simulink model "ImpedanceControl"  (R2017a)
(part 12 of 14)

-((imag(sin(q6).*(cos(q2-q3).*4.698463103929542e-1+sin(q2-q3).*sin(q4).*6.710100716628342e-1+cos(q5).*(cos(q2-q3).*8.191520442889917e-1-sin(q2-q3).*sin(q4).*5.735764363510462e-1).*5.735764363510462e-1-sin(q2-q3).*cos(q4).*sin(q5).*5.735764363510462e-1))+real(sqrt((cos(q2-q3).*3.289899283371657e-1+sin(q2-q3).*sin(q4).*4.698463103929542e-1-cos(q5).*(cos(q2-q3).*8.191520442889917e-1-sin(q2-q3).*sin(q4).*5.735764363510462e-1).*8.191520442889917e-1+sin(q2-q3).*cos(q4).*sin(q5).*8.191520442889917e-1).^2+(sin(q6).*(cos(q2-q3).*sin(q5).*8.191520442889917e-1+sin(q2-q3).*cos(q4).*cos(q5)-sin(q2-q3).*sin(q4).*sin(q5).*5.735764363510462e-1)-cos(q6).*(cos(q2-q3).*4.698463103929542e-1+sin(q2-q3).*sin(q4).*6.710100716628342e-1+cos(q5).*(cos(q2-q3).*8.191520442889917e-1-sin(q2-q3).*sin(q4).*5.735764363510462e-1).*5.735764363510462e-1-sin(q2-q3).*cos(q4).*sin(q5).*5.735764363510462e-1)).^2))+imag(cos(q6).*(cos(q2-q3).*sin(q5).*8.191520442889917e-1+sin(q2-q3).*cos(q4).*cos(q5)-sin(q2-q3).*sin(q4).*sin(q5).*5.735764363510462e-1))).^2.*((real(dq6.*sin(q6).*(cos(q2-q3).*cos(q5).*(-8.191520442889917e-1)+sin(q2-q3).*cos(q4).*sin(q5)+sin(q2-q3).*cos(q5).*sin(q4).*5.735764363510462e-1))-real(cos(q6).*(dq5.*cos(q2-q3).*sin(q5).*8.191520442889917e-1+sin(q2-q3).*cos(q5).*(dq2-dq3).*8.191520442889917e-1+dq4.*sin(q2-q3).*cos(q4).*cos(q5).*5.735764363510462e-1+dq5.*sin(q2-q3).*cos(q4).*cos(q5)-dq4.*sin(q2-q3).*sin(q4).*sin(q5)-dq5.*sin(q2-q3).*sin(q4).*sin(q5).*5.735764363510462e-1+cos(q2-q3).*cos(q4).*sin(q5).*(dq2-dq3)+cos(q2-q3).*cos(q5).*sin(q4).*(dq2-dq3).*5.735764363510462e-1))+imag(1.0./sqrt((cos(q2-q3).*3.289899283371657e-1+sin(q2-q3).*sin(q4).*4.698463103929542e-1-cos(q5).*(cos(q2-q3).*8.191520442889917e-1-sin(q2-q3).*sin(q4).*5.735764363510462e-1).*8.191520442889917e-1+sin(q2-q3).*cos(q4).*sin(q5).*8.191520442889917e-1).^2+(sin(q6).*(cos(q2-q3).*sin(q5).*8.191520442889917e-1+sin(q2-q3).*cos(q4).*cos(q5)-sin(q2-q3).*sin(q4).*sin(q5).*5.735764363510462e-1)-cos(q6).*(cos(q2-q3).*4.698463103929542e-1+sin(q2-q3).*sin(q4).*6.710100716628342e-1+cos(q5).*(cos(q2-q3).*8.191520442889917e-1-sin(q2-q3).*sin(q4).*5.735764363510462e-1).*5.735764363510462e-1-sin(q2-q3).*cos(q4).*sin(q5).*5.735764363510462e-1)).^2).*((cos(q2-q3).*3.289899283371657e-1+sin(q2-q3).*sin(q4).*4.698463103929542e-1-cos(q5).*(cos(q2-q3).*8.191520442889917e-1-sin(q2-q3).*sin(q4).*5.735764363510462e-1).*8.191520442889917e-1+sin(q2-q3).*cos(q4).*sin(q5).*8.191520442889917e-1).*(sin(q5).*(sin(q2-q3).*(dq2-dq3).*8.191520442889917e-1+dq4.*sin(q2-q3).*cos(q4).*5.735764363510462e-1+cos(q2-q3).*sin(q4).*(dq2-dq3).*5.735764363510462e-1).*8.191520442889917e-1-dq5.*cos(q5).*(cos(q2-q3).*8.191520442889917e-1-sin(q2-q3).*sin(q4).*5.735764363510462e-1).*8.191520442889917e-1+dq4.*sin(q2-q3).*cos(q5).*sin(q4).*8.191520442889917e-1+dq5.*sin(q2-q3).*cos(q4).*sin(q5).*8.191520442889917e-1-cos(q2-q3).*cos(q4).*cos(q5).*(dq2-dq3).*8.191520442889917e-1).*2.0-(cos(q6).*(sin(q5).*(cos(q2-q3).*8.191520442889917e-1-sin(q2-q3).*sin(q4).*5.735764363510462e-1).*5.735764363510462e-1+sin(q2-q3).*cos(q4).*cos(q5).*5.735764363510462e-1)-sin(q6).*(cos(q2-q3).*cos(q5).*(-8.191520442889917e-1)+sin(q2-q3).*cos(q4).*sin(q5)+sin(q2-q3).*cos(q5).*sin(q4).*5.735764363510462e-1)).*(cos(q6).*(cos(q5).*(sin(q2-q3).*(dq2-dq3).*8.191520442889917e-1+dq4.*sin(q2-q3).*cos(q4).*5.735764363510462e-1+cos(q2-q3).*sin(q4).*(dq2-dq3).*5.735764363510462e-1).*5.735764363510462e-1+sin(q2-q3).*(dq2-dq3).*4.698463103929542e-1-dq4.*sin(q2-q3).*cos(q4).*6.710100716628342e-1-cos(q2-q3).*sin(q4).*(dq2-dq3).*6.710100716628342e-1+dq5.*sin(q5).*(cos(q2-q3).*8.191520442889917e-1-sin(q2-q3).*sin(q4).*5.735764363510462e-1).*5.735764363510462e-1+dq5.*sin(q2-q3).*cos(q4).*cos(q5).*5.735764363510462e-1-dq4.*sin(q2-q3).*sin(q4).*sin(q5).*5.735764363510462e-1+cos(q2-q3).*cos(q4).*sin(q5).*(dq2-dq3).*5.735764363510462e-1)-sin(q6).*(dq5.*cos(q2-q3).*cos(q5).*(-8.191520442889917e-1)+sin(q2-q3).*sin(q5).*(dq2-dq3).*8.191520442889917e-1+dq4.*sin(q2-q3).*cos(q4).*sin(q5).*5.735764363510462e-1+dq4.*sin(q2-q3).*cos(q5).*sin(q4)+dq5.*sin(q2-q3).*cos(q4).*sin(q5)+dq5.*sin(q2-q3).*cos(q5).*sin(q4).*5.735764363510462e-1-cos(q2-q3).*cos(q4).*cos(q5).*(dq2-dq3)+cos(q2-q3).*sin(q4).*sin(q5).*(dq2-dq3).*5.735764363510462e-1)+dq6.*sin(q6).*(cos(q2-q3).*4.698463103929542e-1+sin(q2-q3).*sin(q4).*6.710100716628342e-1+cos(q5).*(cos(q2-q3).*8.191520442889917e-1-sin(q2-q3).*sin(q4).*5.735764363510462e-1).*5.735764363510462e-1-sin(q2-q3).*cos(q4).*sin(q5).*5.735764363510462e-1)+dq6.*cos(q6).*(cos(q2-q3).*sin(q5).*8.191520442889917e-1+sin(q2-q3).*cos(q4).*cos(q5)-sin(q2-q3).*sin(q4).*sin(q5).*5.735764363510462e-1)).*2.0-(sin(q5).*(cos(q2-q3).*8.191520442889917e-1-sin(q2-q3).*sin(q4).*5.735764363510462e-1).*8.191520442889917e-1+sin(q2-q3).*cos(q4).*cos(q5).*8.191520442889917e-1).*(cos(q5).*(sin(q2-q3).*(dq2-dq3).*8.191520442889917e-1+dq4.*sin(q2-q3).*cos(q4).*5.735764363510462e-1+cos(q2-q3).*sin(q4).*(dq2-dq3).*5.735764363510462e-1).*8.191520442889917e-1-sin(q2-q3).*(dq2-dq3).*3.289899283371657e-1+dq4.*sin(q2-q3).*cos(q4).*4.698463103929542e-1+cos(q2-q3).*sin(q4).*(dq2-dq3).*4.698463103929542e-1+dq5.*sin(q5).*(cos(q2-q3).*8.191520442889917e-1-sin(q2-q3).*sin(q4).*5.735764363510462e-1).*8.191520442889917e-1+dq5.*sin(q2-q3).*cos(q4).*cos(q5).*8.191520442889917e-1-dq4.*sin(q2-q3).*sin(q4).*sin(q5).*8.191520442889917e-1+cos(q2-q3).*cos(q4).*sin(q5).*(dq2-dq3).*8.191520442889917e-1).*2.0+(sin(q6).*(cos(q2-q3).*sin(q5).*8.191520442889917e-1+sin(q2-q3).*cos(q4).*cos(q5)-sin(q2-q3).*sin(q4).*sin(q5).*5.735764363510462e-1)-cos(q6).*(cos(q2-q3).*4.698463103929542e-1+sin(q2-q3).*sin(q4).*6.710100716628342e-1+cos(q5).*(cos(q2-q3).*8.191520442889917e-1-sin(q2-q3).*sin(q4).*5.735764363510462e-1).*5.735764363510462e-1-sin(q2-q3).*cos(q4).*sin(q5).*5.735764363510462e-1)).*(cos(q6).*(sin(q5).*(sin(q2-q3).*(dq2-dq3).*8.191520442889917e-1+dq4.*sin(q2-q3).*cos(q4).*5.735764363510462e-1+cos(q2-q3).*sin(q4).*(dq2-dq3).*5.735764363510462e-1).*5.735764363510462e-1-dq5.*cos(q5).*(cos(q2-q3).*8.191520442889917e-1-sin(q2-q3).*sin(q4).*5.735764363510462e-1).*5.735764363510462e-1+dq4.*sin(q2-q3).*cos(q5).*sin(q4).*5.735764363510462e-1+dq5.*sin(q2-q3).*cos(q4).*sin(q5).*5.735764363510462e-1-cos(q2-q3).*cos(q4).*cos(q5).*(dq2-dq3).*5.735764363510462e-1)+sin(q6).*(dq5.*cos(q2-q3).*sin(q5).*8.191520442889917e-1+sin(q2-q3).*cos(q5).*(dq2-dq3).*8.191520442889917e-1+dq4.*sin(q2-q3).*cos(q4).*cos(q5).*5.735764363510462e-1+dq5.*sin(q2-q3).*cos(q4).*cos(q5)-dq4.*sin(q2-q3).*sin(q4).*sin(q5)-dq5.*sin(q2-q3).*sin(q4).*sin(q5).*5.735764363510462e-1+cos(q2-q3).*cos(q4).*sin(q5).*(dq2-dq3)+cos(q2-q3).*cos(q5).*sin(q4).*(dq2-dq3).*5.735764363510462e-1)+dq6.*sin(q6).*(sin(q5).*(cos(q2-q3).*8.191520442889917e-1-sin(q2-q3).*sin(q4).*5.735764363510462e-1).*5.735764363510462e-1+sin(q2-q3).*cos(q4).*cos(q5).*5.735764363510462e-1)+dq6.*cos(q6).*(cos(q2-q3).*cos(q5).*(-8.191520442889917e-1)+sin(q2-q3).*cos(q4).*sin(q5)+sin(q2-q3).*cos(q5).*sin(q4).*5.735764363510462e-1)).*2.0)).*(1.0./2.0)+imag(1.0./((cos(q2-q3).*3.289899283371657e-1+sin(q2-q3).*sin(q4).*4.698463103929542e-1-cos(q5).*(cos(q2-q3).*8.191520442889917e-1-sin(q2-q3).*sin(q4).*5.735764363510462e-1).*8.191520442889917e-1+sin(q2-q3).*cos(q4).*sin(q5).*8.191520442889917e-1).^2+(sin(q6).*(cos(q2-q3).*sin(q5).*8.191520442889917e-1+sin(q2-q3).*cos(q4).*cos(q5)-sin(q2-q3).*sin(q4).*sin(q5).*5.735764363510462e-1)-cos(q6).*(cos(q2-q3).*4.698463103929542e-1+sin(q2-q3).*sin(q4).*6.710100716628342e-1+cos(q5).*(cos(q2-q3).*8.191520442889917e-1-sin(q2-q3).*sin(q4).*5.735764363510462e-1).*5.735764363510462e-1-sin(q2-q3).*cos(q4).*sin(q5).*5.735764363510462e-1)).^2).^(3.0./2.0).*((sin(q6).*(cos(q2-q3).*sin(q5).*8.191520442889917e-1+sin(q2-q3).*cos(q4).*cos(q5)-sin(q2-q3).*sin(q4).*sin(q5).*5.735764363510462e-1)-cos(q6).*(cos(q2-q3).*4.698463103929542e-1+sin(q2-q3).*sin(q4).*6.710100716628342e-1+cos(q5).*(cos(q2-q3).*8.191520442889917e-1-sin(q2-q3).*sin(q4).*5.735764363510462e-1).*5.735764363510462e-1-sin(q2-q3).*cos(q4).*sin(q5).*5.735764363510462e-1)).*(cos(q6).*(cos(q5).*(sin(q2-q3).*(dq2-dq3).*8.191520442889917e-1+dq4.*sin(q2-q3).*cos(q4).*5.735764363510462e-1+cos(q2-q3).*sin(q4).*(dq2-dq3).*5.735764363510462e-1).*5.735764363510462e-1+sin(q2-q3).*(dq2-dq3).*4.698463103929542e-1-dq4.*sin(q2-q3).*cos(q4).*6.710100716628342e-1-cos(q2-q3).*sin(q4).*(dq2-dq3).*6.710100716628342e-1+dq5.*sin(q5).*(cos(q2-q3).*8.191520442889917e-1-sin(q2-q3).*sin(q4).*5.735764363510462e-1).*5.735764363510462e-1+dq5.*sin(q2-q3).*cos(q4).*cos(q5).*5.735764363510462e-1-dq4.*sin(q2-q3).*sin(q4).*sin(q5).*5.735764363510462e-1+cos(q2-q3).*cos(q4).*sin(q5).*(dq2-dq3).*5.735764363510462e-1)-sin(q6).*(dq5.*cos(q2-q3).*cos(q5).*(-8.191520442889917e-1)+sin(q2-q3).*sin(q5).*(dq2-dq3).*8.191520442889917e-1+dq4.*sin(q2-q3).*cos(q4).*sin(q5).*5.735764363510462e-1+dq4.*sin(q2-q3).*cos(q5).*sin(q4)+dq5.*sin(q2-q3).*cos(q4).*sin(q5)+dq5.*sin(q2-q3).*cos(q5).*sin(q4).*5.735764363510462e-1-cos(q2-q3).*cos(q4).*cos(q5).*(dq2-dq3)+cos(q2-q3).*sin(q4).*sin(q5).*(dq2-dq3).*5.735764363510462e-1)+dq6.*sin(q6).*(cos(q2-q3).*4.698463103929542e-1+sin(q2-q3).*sin(q4).*6.710100716628342e-1+cos(q5).*(cos(q2-q3).*8.191520442889917e-1-sin(q2-q3).*sin(q4).*5.735764363510462e-1).*5.735764363510462e-1-sin(q2-q3).*cos(q4).*sin(q5).*5.735764363510462e-1)+dq6.*cos(q6).*(cos(q2-q3).*sin(q5).*8.191520442889917e-1+sin(q2-q3).*cos(q4).*cos(q5)-sin(q2-q3).*sin(q4).*sin(q5).*5.735764363510462e-1)).*2.0+(cos(q2-q3).*3.289899283371657e-1+sin(q2-q3).*sin(q4).*4.698463103929542e-1-cos(q5).*(cos(q2-q3).*8.191520442889917e-1-sin(q2-q3).*sin(q4).*5.735764363510462e-1).*8.191520442889917e-1+sin(q2-q3).*cos(q4).*sin(q5).*8.191520442889917e-1).*(cos(q5).*(sin(q2-q3).*(dq2-dq3).*8.191520442889917e-1+dq4.*sin(q2-q3).*cos(q4).*5.735764363510462e-1+cos(q2-q3).*sin(q4).*(dq2-dq3).*5.735764363510462e-1).*8.191520442889917e-1-sin(q2-q3).*(dq2-dq3).*3.289899283371657e-1+dq4.*sin(q2-q3).*cos(q4).*4.698463103929542e-1+cos(q2-q3).*sin(q4).*(dq2-dq3).*4.698463103929542e-1+dq5.*sin(q5).*(cos(q2-q3).*8.191520442889917e-1-sin(q2-q3).*sin(q4).*5.735764363510462e-1).*8.191520442889917e-1+dq5.*sin(q2-q3).*cos(q4).*cos(q5).*8.191520442889917e-1-dq4.*sin(q2-q3).*sin(q4).*sin(q5).*8.191520442889917e-1+cos(q2-q3).*cos(q4).*sin(q5).*(dq2-dq3).*8.191520442889917e-1).*2.0).*((sin(q6).*(cos(q2-q3).*sin(q5).*8.191520442889917e-1+sin(q2-q3).*cos(q4).*cos(q5)-sin(q2-q3).*sin(q4).*sin(q5).*5.735764363510462e-1)-cos(q6).*(cos(q2-q3).*4.698463103929542e-1+sin(q2-q3).*sin(q4).*6.710100716628342e-1+cos(q5).*(cos(q2-q3).*8.191520442889917e-1-sin(q2-q3).*sin(q4).*5.735764363510462e-1).*5.735764363510462e-1-sin(q2-q3).*cos(q4).*sin(q5).*5.735764363510462e-1)).*(cos(q6).*(sin(q5).*(cos(q2-q3).*8.191520442889917e-1-sin(q2-q3).*sin(q4).*5.735764363510462e-1).*5.735764363510462e-1+sin(q2-q3).*cos(q4).*cos(q5).*5.735764363510462e-1)-sin(q6).*(cos(q2-q3).*cos(q5).*(-8.191520442889917e-1)+sin(q2-q3).*cos(q4).*sin(q5)+sin(q2-q3).*cos(q5).*sin(q4).*5.735764363510462e-1)).*2.0+(sin(q5).*(cos(q2-q3).*8.191520442889917e-1-sin(q2-q3).*sin(q4).*5.735764363510462e-1).*8.191520442889917e-1+sin(q2-q3).*cos(q4).*cos(q5).*8.191520442889917e-1).*(cos(q2-q3).*3.289899283371657e-1+sin(q2-q3).*sin(q4).*4.698463103929542e-1-cos(q5).*(cos(q2-q3).*8.191520442889917e-1-sin(q2-q3).*sin(q4).*5.735764363510462e-1).*8.191520442889917e-1+sin(q2-q3).*cos(q4).*sin(q5).*8.191520442889917e-1).*2.0)).*(1.0./4.0)+real(sin(q6).*(sin(q5).*(sin(q2-q3).*(dq2-dq3).*8.191520442889917e-1+dq4.*sin(q2-q3).*cos(q4).*5.735764363510462e-1+cos(q2-q3).*sin(q4).*(dq2-dq3).*5.735764363510462e-1).*5.735764363510462e-1-dq5.*cos(q5).*(cos(q2-q3).*8.191520442889917e-1-sin(q2-q3).*sin(q4).*5.735764363510462e-1).*5.735764363510462e-1+dq4.*sin(q2-q3).*cos(q5).*sin(q4).*5.735764363510462e-1+dq5.*sin(q2-q3).*cos(q4).*sin(q5).*5.735764363510462e-1-cos(q2-q3).*cos(q4).*cos(q5).*(dq2-dq3).*5.735764363510462e-1))-real(dq6.*cos(q6).*(sin(q5).*(cos(q2-q3).*8.191520442889917e-1-sin(q2-q3).*sin(q4).*5.735764363510462e-1).*5.735764363510462e-1+sin(q2-q3).*cos(q4).*cos(q5).*5.735764363510462e-1)))./(imag(sin(q6).*(cos(q2-q3).*4.698463103929542e-1+sin(q2-q3).*sin(q4).*6.710100716628342e-1+cos(q5).*(cos(q2-q3).*8.191520442889917e-1-sin(q2-q3).*sin(q4).*5.735764363510462e-1).*5.735764363510462e-1-sin(q2-q3).*cos(q4).*sin(q5).*5.735764363510462e-1))+real(sqrt((cos(q2-q3).*3.289899283371657e-1+sin(q2-q3).*sin(q4).*4.698463103929542e-1-cos(q5).*(cos(q2-q3).*8.191520442889917e-1-sin(q2-q3).*sin(q4).*5.735764363510462e-1).*8.191520442889917e-1+sin(q2-q3).*cos(q4).*sin(q5).*8.191520442889917e-1).^2+(sin(q6).*(cos(q2-q3).*sin(q5).*8.191520442889917e-1+sin(q2-q3).*cos(q4).*cos(q5)-sin(q2-q3).*sin(q4).*sin(q5).*5.735764363510462e-1)-cos(q6).*(cos(q2-q3).*4.698463103929542e-1+sin(q2-q3).*sin(q4).*6.710100716628342e-1+cos(q5).*(cos(q2-q3).*8.191520442889917e-1-sin(q2-q3).*sin(q4).*5.735764363510462e-1).*5.735764363510462e-1-sin(q2-q3).*cos(q4).*sin(q5).*5.735764363510462e-1)).^2))+imag(cos(q6).*(cos(q2-q3).*sin(q5).*8.191520442889917e-1+sin(q2-q3).*cos(q4).*cos(q5)-sin(q2-q3).*sin(q4).*sin(q5).*5.735764363510462e-1)))+1.0./(imag(sin(q6).*(cos(q2-q3).*4.698463103929542e-1+sin(q2-q3).*sin(q4).*6.710100716628342e-1+cos(q5).*(cos(q2-q3).*8.191520442889917e-1-sin(q2-q3).*sin(q4).*5.735764363510462e-1).*5.735764363510462e-1-sin(q2-q3).*cos(q4).*sin(q5).*5.735764363510462e-1))+real(sqrt((cos(q2-q3).*3.289899283371657e-1+sin(q2-q3).*sin(q4).*4.698463103929542e-1-cos(q5).*(cos(q2-q3).*8.191520442889917e-1-sin(q2-q3).*sin(q4).*5.735764363510462e-1).*8.191520442889917e-1+sin(q2-q3).*cos(q4).*sin(q5).*8.191520442889917e-1).^2+(sin(q6).*(cos(q2-q3).*sin(q5).*8.191520442889917e-1+sin(q2-q3).*cos(q4).*cos(q5)-sin(q2-q3).*sin(q4).*sin(q5).*5.735764363510462e-1)-cos(q6).*(cos(q2-q3).*4.698463103929542e-1+sin(q2-q3).*sin(q4).*6.710100716628342e-1+cos(q5).*(cos(q2-q3).*8.191520442889917e-1-sin(q2-q3).*sin(q4).*5.735764363510462e-1).*5.735764363510462e-1-sin(q2-q3).*cos(q4).*sin(q5).*5.735764363510462e-1)).^2))+imag(cos(q6).*(cos(q2-q3).*sin(q5).*8.191520442889917e-1+sin(q2-q3).*cos(q4).*cos(q5)-sin(q2-q3).*sin(q4).*sin(q5).*5.735764363510462e-1))).^2.*(real(sin(q6).*(cos(q2-q3).*4.698463103929542e-1+sin(q2-q3).*sin(q4).*6.710100716628342e-1+cos(q5).*(cos(q2-q3).*8.191520442889917e-1-sin(q2-q3).*sin(q4).*5.735764363510462e-1).*5.735764363510462e-1-sin(q2-q3).*cos(q4).*sin(q5).*5.735764363510462e-1))-imag(sqrt((cos(q2-q3).*3.289899283371657e-1+sin(q2-q3).*sin(q4).*4.698463103929542e-1-cos(q5).*(cos(q2-q3).*8.191520442889917e-1-sin(q2-q3).*sin(q4).*5.735764363510462e-1).*8.191520442889917e-1+sin(q2-q3).*cos(q4).*sin(q5).*8.191520442889917e-1).^2+(sin(q6).*(cos(q2-q3).*sin(q5).*8.191520442889917e-1+sin(q2-q3).*cos(q4).*cos(q5)-sin(q2-q3).*sin(q4).*sin(q5).*5.735764363510462e-1)-cos(q6).*(cos(q2-q3).*4.698463103929542e-1+sin(q2-q3).*sin(q4).*6.710100716628342e-1+cos(q5).*(cos(q2-q3).*8.191520442889917e-1-sin(q2-q3).*sin(q4).*5.735764363510462e-1).*5.735764363510462e-1-sin(q2-q3).*cos(q4).*sin(q5).*5.735764363510462e-1)).^2))+real(cos(q6).*(cos(q2-q3).*sin(q5).*8.191520442889917e-1+sin(q2-q3).*cos(q4).*cos(q5)-sin(q2-q3).*sin(q4).*sin(q5).*5.735764363510462e-1))).*(-imag(dq6.*sin(q6).*(cos(q2-q3).*cos(q5).*(-8.191520442889917e-1)+sin(q2-q3).*cos(q4).*sin(q5)+sin(q2-q3).*cos(q5).*sin(q4).*5.735764363510462e-1))+imag(cos(q6).*(dq5.*cos(q2-q3).*sin(q5).*8.191520442889917e-1+sin(q2-q3).*cos(q5).*(dq2-dq3).*8.191520442889917e-1+dq4.*sin(q2-q3).*cos(q4).*cos(q5).*5.735764363510462e-1+dq5.*sin(q2-q3).*cos(q4).*cos(q5)-dq4.*sin(q2-q3).*sin(q4).*sin(q5)-dq5.*sin(q2-q3).*sin(q4).*sin(q5).*5.735764363510462e-1+cos(q2-q3).*cos(q4).*sin(q5).*(dq2-dq3)+cos(q2-q3).*cos(q5).*sin(q4).*(dq2-dq3).*5.735764363510462e-1))+real(1.0./sqrt((cos(q2-q3).*3.289899283371657e-1+sin(q2-q3).*sin(q4).*4.698463103929542e-1-cos(q5).*(cos(q2-q3).*8.191520442889917e-1-sin(q2-q3).*sin(q4).*5.735764363510462e-1).*8.191520442889917e-1+sin(q2-q3).*cos(q4).*sin(q5).*8.191520442889917e-1).^2+(sin(q6).*(cos(q2-q3).*sin(q5).*8.191520442889917e-1+sin(q2-q3).*cos(q4).*cos(q5)-sin(q2-q3).*sin(q4).*sin(q5).*5.735764363510462e-1)-cos(q6).*(cos(q2-q3).*4.698463103929542e-1+sin(q2-q3).*sin(q4).*6.710100716628342e-1+cos(q5).*(cos(q2-q3).*8.191520442889917e-1-sin(q2-q3).*sin(q4).*5.735764363510462e-1).*5.735764363510462e-1-sin(q2-q3).*cos(q4).*sin(q5).*5.735764363510462e-1)).^2).*((cos(q2-q3).*3.289899283371657e-1+sin(q2-q3).*sin(q4).*4.698463103929542e-1-cos(q5).*(cos(q2-q3).*8.191520442889917e-1-sin(q2-q3).*sin(q4).*5.735764363510462e-1).*8.191520442889917e-1+sin(q2-q3).*cos(q4).*sin(q5).*8.191520442889917e-1).*(sin(q5).*(sin(q2-q3).*(dq2-dq3).*8.191520442889917e-1+dq4.*sin(q2-q3).*cos(q4).*5.735764363510462e-1+cos(q2-q3).*sin(q4).*(dq2-dq3).*5.735764363510462e-1).*8.191520442889917e-1-dq5.*cos(q5).*(cos(q2-q3).*8.191520442889917e-1-sin(q2-q3).*sin(q4).*5.735764363510462e-1).*8.191520442889917e-1+dq4.*sin(q2-q3).*cos(q5).*sin(q4).*8.191520442889917e-1+dq5.*sin(q2-q3).*cos(q4).*sin(q5).*8.191520442889917e-1-cos(q2-q3).*cos(q4).*cos(q5).*(dq2-dq3).*8.191520442889917e-1).*2.0-(cos(q6).*(sin(q5).*(cos(q2-q3).*8.191520442889917e-1-sin(q2-q3).*sin(q4).*5.735764363510462e-1).*5.735764363510462e-1+sin(q2-q3).*cos(q4).*cos(q5).*5.735764363510462e-1)-sin(q6).*(cos(q2-q3).*cos(q5).*(-8.191520442889917e-1)+sin(q2-q3).*cos(q4).*sin(q5)+sin(q2-q3).*cos(q5).*sin(q4).*5.735764363510462e-1)).*(cos(q6).*(cos(q5).*(sin(q2-q3).*(dq2-dq3).*8.191520442889917e-1+dq4.*sin(q2-q3).*cos(q4).*5.735764363510462e-1+cos(q2-q3).*sin(q4).*(dq2-dq3).*5.735764363510462e-1).*5.735764363510462e-1+sin(q2-q3).*(dq2-dq3).*4.698463103929542e-1-dq4.*sin(q2-q3).*cos(q4).*6.710100716628342e-1-cos(q2-q3).*sin(q4).*(dq2-dq3).*6.710100716628342e-1+dq5.*sin(q5).*(cos(q2-q3).*8.191520442889917e-1-sin(q2-q3).*sin(q4).*5.735764363510462e-1).*5.735764363510462e-1+dq5.*sin(q2-q3).*cos(q4).*cos(q5).*5.735764363510462e-1-dq4.*sin(q2-q3).*sin(q4).*sin(q5).*5.735764363510462e-1+cos(q2-q3).*cos(q4).*sin(q5).*(dq2-dq3).*5.735764363510462e-1)-sin(q6).*(dq5.*cos(q2-q3).*cos(q5).*(-8.191520442889917e-1)+sin(q2-q3).*sin(q5).*(dq2-dq3).*8.191520442889917e-1+dq4.*sin(q2-q3).*cos(q4).*sin(q5).*5.735764363510462e-1+dq4.*sin(q2-q3).*cos(q5).*sin(q4)+dq5.*sin(q2-q3).*cos(q4).*sin(q5)+dq5.*sin(q2-q3).*cos(q5).*sin(q4).*5.735764363510462e-1-cos(q2-q3).*cos(q4).*cos(q5).*(dq2-dq3)+cos(q2-q3).*sin(q4).*sin(q5).*(dq2-dq3).*5.735764363510462e-1)+dq6.*sin(q6).*(cos(q2-q3).*4.698463103929542e-1+sin(q2-q3).*sin(q4).*6.710100716628342e-1+cos(q5).*(cos(q2-q3).*8.191520442889917e-1-sin(q2-q3).*sin(q4).*5.735764363510462e-1).*5.735764363510462e-1-sin(q2-q3).*cos(q4).*sin(q5).*5.735764363510462e-1)+dq6.*cos(q6).*(cos(q2-q3).*sin(q5).*8.191520442889917e-1+sin(q2-q3).*cos(q4).*cos(q5)-sin(q2-q3).*sin(q4).*sin(q5).*5.735764363510462e-1)).*2.0-(sin(q5).*(cos(q2-q3).*8.191520442889917e-1-sin(q2-q3).*sin(q4).*5.735764363510462e-1).*8.191520442889917e-1+sin(q2-q3).*cos(q4).*cos(q5).*8.191520442889917e-1).*(cos(q5).*(sin(q2-q3).*(dq2-dq3).*8.191520442889917e-1+dq4.*sin(q2-q3).*cos(q4).*5.735764363510462e-1+cos(q2-q3).*sin(q4).*(dq2-dq3).*5.735764363510462e-1).*8.191520442889917e-1-sin(q2-q3).*(dq2-dq3).*3.289899283371657e-1+dq4.*sin(q2-q3).*cos(q4).*4.698463103929542e-1+cos(q2-q3).*sin(q4).*(dq2-dq3).*4.698463103929542e-1+dq5.*sin(q5).*(cos(q2-q3).*8.191520442889917e-1-sin(q2-q3).*sin(q4).*5.735764363510462e-1).*8.191520442889917e-1+dq5.*sin(q2-q3).*cos(q4).*cos(q5).*8.191520442889917e-1-dq4.*sin(q2-q3).*sin(q4).*sin(q5).*8.191520442889917e-1+cos(q2-q3).*cos(q4).*sin(q5).*(dq2-dq3).*8.191520442889917e-1).*2.0+(sin(q6).*(cos(q2-q3).*sin(q5).*8.191520442889917e-1+sin(q2-q3).*cos(q4).*cos(q5)-sin(q2-q3).*sin(q4).*sin(q5).*5.735764363510462e-1)-cos(q6).*(cos(q2-q3).*4.698463103929542e-1+sin(q2-q3).*sin(q4).*6.710100716628342e-1+cos(q5).*(cos(q2-q3).*8.191520442889917e-1-sin(q2-q3).*sin(q4).*5.735764363510462e-1).*5.735764363510462e-1-sin(q2-q3).*cos(q4).*sin(q5).*5.735764363510462e-1)).*(cos(q6).*(sin(q5).*(sin(q2-q3).*(dq2-dq3).*8.191520442889917e-1+dq4.*sin(q2-q3).*cos(q4).*5.735764363510462e-1+cos(q2-q3).*sin(q4).*(dq2-dq3).*5.735764363510462e-1).*5.735764363510462e-1-dq5.*cos(q5).*(cos(q2-q3).*8.191520442889917e-1-sin(q2-q3).*sin(q4).*5.735764363510462e-1).*5.735764363510462e-1+dq4.*sin(q2-q3).*cos(q5).*sin(q4).*5.735764363510462e-1+dq5.*sin(q2-q3).*cos(q4).*sin(q5).*5.735764363510462e-1-cos(q2-q3).*cos(q4).*cos(q5).*(dq2-dq3).*5.735764363510462e-1)+sin(q6).*(dq5.*cos(q2-q3).*sin(q5).*8.191520442889917e-1+sin(q2-q3).*cos(q5).*(dq2-dq3).*8.191520442889917e-1+dq4.*sin(q2-q3).*cos(q4).*cos(q5).*5.735764363510462e-1+dq5.*sin(q2-q3).*cos(q4).*cos(q5)-dq4.*sin(q2-q3).*sin(q4).*sin(q5)-dq5.*sin(q2-q3).*sin(q4).*sin(q5).*5.735764363510462e-1+cos(q2-q3).*cos(q4).*sin(q5).*(dq2-dq3)+cos(q2-q3).*cos(q5).*sin(q4).*(dq2-dq3).*5.735764363510462e-1)+dq6.*sin(q6).*(sin(q5).*(cos(q2-q3).*8.191520442889917e-1-sin(q2-q3).*sin(q4).*5.735764363510462e-1).*5.735764363510462e-1+sin(q2-q3).*cos(q4).*cos(q5).*5.735764363510462e-1)+dq6.*cos(q6).*(cos(q2-q3).*cos(q5).*(-8.191520442889917e-1)+sin(q2-q3).*cos(q4).*sin(q5)+sin(q2-q3).*cos(q5).*sin(q4).*5.735764363510462e-1)).*2.0)).*(1.0./2.0)+real(1.0./((cos(q2-q3).*3.289899283371657e-1+sin(q2-q3).*sin(q4).*4.698463103929542e-1-cos(q5).*(cos(q2-q3).*8.191520442889917e-1-sin(q2-q3).*sin(q4).*5.735764363510462e-1).*8.191520442889917e-1+sin(q2-q3).*cos(q4).*sin(q5).*8.191520442889917e-1).^2+(sin(q6).*(cos(q2-q3).*sin(q5).*8.191520442889917e-1+sin(q2-q3).*cos(q4).*cos(q5)-sin(q2-q3).*sin(q4).*sin(q5).*5.735764363510462e-1)-cos(q6).*(cos(q2-q3).*4.698463103929542e-1+sin(q2-q3).*sin(q4).*6.710100716628342e-1+cos(q5).*(cos(q2-q3).*8.191520442889917e-1-sin(q2-q3).*sin(q4).*5.735764363510462e-1).*5.735764363510462e-1-sin(q2-q3).*cos(q4).*sin(q5).*5.735764363510462e-1)).^2).^(3.0./2.0).*((sin(q6).*(cos(q2-q3).*sin(q5).*8.191520442889917e-1+sin(q2-q3).*cos(q4).*cos(q5)-sin(q2-q3).*sin(q4).*sin(q5).*5.735764363510462e-1)-cos(q6).*(cos(q2-q3).*4.698463103929542e-1+sin(q2-q3).*sin(q4).*6.710100716628342e-1+cos(q5).*(cos(q2-q3).*8.191520442889917e-1-sin(q2-q3).*sin(q4).*5.735764363510462e-1).*5.735764363510462e-1-sin(q2-q3).*cos(q4).*sin(q5).*5.735764363510462e-1)).*(cos(q6).*(cos(q5).*(sin(q2-q3).*(dq2-dq3).*8.191520442889917e-1+dq4.*sin(q2-q3).*cos(q4).*5.735764363510462e-1+cos(q2-q3).*sin(q4).*(dq2-dq3).*5.735764363510462e-1).*5.735764363510462e-1+sin(q2-q3).*(dq2-dq3).*4.698463103929542e-1-dq4.*sin(q2-q3).*cos(q4).*6.710100716628342e-1-cos(q2-q3).*sin(q4).*(dq2-dq3).*6.710100716628342e-1+dq5.*sin(q5).*(cos(q2-q3).*8.191520442889917e-1-sin(q2-q3).*sin(q4).*5.735764363510462e-1).*5.735764363510462e-1+dq5.*sin(q2-q3).*cos(q4).*cos(q5).*5.735764363510462e-1-dq4.*sin(q2-q3).*sin(q4).*sin(q5).*5.735764363510462e-1+cos(q2-q3).*cos(q4).*sin(q5).*(dq2-dq3).*5.735764363510462e-1)-sin(q6).*(dq5.*cos(q2-q3).*cos(q5).*(-8.191520442889917e-1)+sin(q2-q3).*sin(q5).*(dq2-dq3).*8.191520442889917e-1+dq4.*sin(q2-q3).*cos(q4).*sin(q5).*5.735764363510462e-1+dq4.*sin(q2-q3).*cos(q5).*sin(q4)+dq5.*sin(q2-q3).*cos(q4).*sin(q5)+dq5.*sin(q2-q3).*cos(q5).*sin(q4).*5.735764363510462e-1-cos(q2-q3).*cos(q4).*cos(q5).*(dq2-dq3)+cos(q2-q3).*sin(q4).*sin(q5).*(dq2-dq3).*5.735764363510462e-1)+dq6.*sin(q6).*(cos(q2-q3).*4.698463103929542e-1+sin(q2-q3).*sin(q4).*6.710100716628342e-1+cos(q5).*(cos(q2-q3).*8.191520442889917e-1-sin(q2-q3).*sin(q4).*5.735764363510462e-1).*5.735764363510462e-1-sin(q2-q3).*cos(q4).*sin(q5).*5.735764363510462e-1)+dq6.*cos(q6).*(cos(q2-q3).*sin(q5).*8.191520442889917e-1+sin(q2-q3).*cos(q4).*cos(q5)-sin(q2-q3).*sin(q4).*sin(q5).*5.735764363510462e-1)).*2.0+(cos(q2-q3).*3.289899283371657e-1+sin(q2-q3).*sin(q4).*4.698463103929542e-1-cos(q5).*(cos(q2-q3).*8.191520442889917e-1-sin(q2-q3).*sin(q4).*5.735764363510462e-1).*8.191520442889917e-1+sin(q2-q3).*cos(q4).*sin(q5).*8.191520442889917e-1).*(cos(q5).*(sin(q2-q3).*(dq2-dq3).*8.191520442889917e-1+dq4.*sin(q2-q3).*cos(q4).*5.735764363510462e-1+cos(q2-q3).*sin(q4).*(dq2-dq3).*5.735764363510462e-1).*8.191520442889917e-1-sin(q2-q3).*(dq2-dq3).*3.289899283371657e-1+dq4.*sin(q2-q3).*cos(q4).*4.698463103929542e-1+cos(q2-q3).*sin(q4).*(dq2-dq3).*4.698463103929542e-1+dq5.*sin(q5).*(cos(q2-q3).*8.191520442889917e-1-sin(q2-q3).*sin(q4).*5.735764363510462e-1).*8.191520442889917e-1+dq5.*sin(q2-q3).*cos(q4).*cos(q5).*8.191520442889917e-1-dq4.*sin(q2-q3).*sin(q4).*sin(q5).*8.191520442889917e-1+cos(q2-q3).*cos(q4).*sin(q5).*(dq2-dq3).*8.191520442889917e-1).*2.0).*((sin(q6).*(cos(q2-q3).*sin(q5).*8.191520442889917e-1+sin(q2-q3).*cos(q4).*cos(q5)-sin(q2-q3).*sin(q4).*sin(q5).*5.735764363510462e-1)-cos(q6).*(cos(q2-q3).*4.698463103929542e-1+sin(q2-q3).*sin(q4).*6.710100716628342e-1+cos(q5).*(cos(q2-q3).*8.191520442889917e-1-sin(q2-q3).*sin(q4).*5.735764363510462e-1).*5.735764363510462e-1-sin(q2-q3).*cos(q4).*sin(q5).*5.735764363510462e-1)).*(cos(q6).*(sin(q5).*(cos(q2-q3).*8.191520442889917e-1-sin(q2-q3).*sin(q4).*5.735764363510462e-1).*5.735764363510462e-1+sin(q2-q3).*cos(q4).*cos(q5).*5.735764363510462e-1)-sin(q6).*(cos(q2-q3).*cos(q5).*(-8.191520442889917e-1)+sin(q2-q3).*cos(q4).*sin(q5)+sin(q2-q3).*cos(q5).*sin(q4).*5.735764363510462e-1)).*2.0+(sin(q5).*(cos(q2-q3).*8.191520442889917e-1-sin(q2-q3).*sin(q4).*5.735764363510462e-1).*8.191520442889917e-1+sin(q2-q3).*cos(q4).*cos(q5).*8.191520442889917e-1).*(cos(q2-q3).*3.289899283371657e-1+sin(q2-q3).*sin(q4).*4.698463103929542e-1-cos(q5).*(cos(q2-q3).*8.191520442889917e-1-sin(q2-q3).*sin(q4).*5.735764363510462e-1).*8.191520442889917e-1+sin(q2-q3).*cos(q4).*sin(q5).*8.191520442889917e-1).*2.0)).*(1.0./4.0)-imag(sin(q6).*(sin(q5).*(sin(q2-q3).*(dq2-dq3).*8.191520442889917e-1+dq4.*sin(q2-q3).*cos(q4).*5.735764363510462e-1+cos(q2-q3).*sin(q4).*(dq2-dq3).*5.735764363510462e-1).*5.735764363510462e-1-dq5.*cos(q5).*(cos(q2-q3).*8.191520442889917e-1-sin(q2-q3).*sin(q4).*5.735764363510462e-1).*5.735764363510462e-1+dq4.*sin(q2-q3).*cos(q5).*sin(q4).*5.735764363510462e-1+dq5.*sin(q2-q3).*cos(q4).*sin(q5).*5.735764363510462e-1-cos(q2-q3).*cos(q4).*cos(q5).*(dq2-dq3).*5.735764363510462e-1))+imag(dq6.*cos(q6).*(sin(q5).*(cos(q2-q3).*8.191520442889917e-1-sin(q2-q3).*sin(q4).*5.735764363510462e-1).*5.735764363510462e-1+sin(q2-q3).*cos(q4).*cos(q5).*5.735764363510462e-1)))-1.0./(imag(sin(q6).*(cos(q2-q3).*4.698463103929542e-1+sin(q2-q3).*sin(q4).*6.710100716628342e-1+cos(q5).*(cos(q2-q3).*8.191520442889917e-1-sin(q2-q3).*sin(q4).*5.735764363510462e-1).*5.735764363510462e-1-sin(q2-q3).*cos(q4).*sin(q5).*5.735764363510462e-1))+real(sqrt((cos(q2-q3).*3.289899283371657e-1+sin(q2-q3).*sin(q4).*4.698463103929542e-1-cos(q5).*(cos(q2-q3).*8.191520442889917e-1-sin(q2-q3).*sin(q4).*5.735764363510462e-1).*8.191520442889917e-1+sin(q2-q3).*cos(q4).*sin(q5).*8.191520442889917e-1).^2+(sin(q6).*(cos(q2-q3).*sin(q5).*8.191520442889917e-1+sin(q2-q3).*cos(q4).*cos(q5)-sin(q2-q3).*sin(q4).*sin(q5).*5.735764363510462e-1)-cos(q6).*(cos(q2-q3).*4.698463103929542e-1+sin(q2-q3).*sin(q4).*6.710100716628342e-1+cos(q5).*(cos(q2-q3).*8.191520442889917e-1-sin(q2-q3).*sin(q4).*5.735764363510462e-1).*5.735764363510462e-1-sin(q2-q3).*cos(q4).*sin(q5).*5.735764363510462e-1)).^2))+imag(cos(q6).*(cos(q2-q3).*sin(q5).*8.191520442889917e-1+sin(q2-q3).*cos(q4).*cos(q5)-sin(q2-q3).*sin(q4).*sin(q5).*5.735764363510462e-1))).^2.*(real(sin(q6).*(sin(q5).*(cos(q2-q3).*8.191520442889917e-1-sin(q2-q3).*sin(q4).*5.735764363510462e-1).*5.735764363510462e-1+sin(q2-q3).*cos(q4).*cos(q5).*5.735764363510462e-1))+imag(1.0./sqrt((cos(q2-q3).*3.289899283371657e-1+sin(q2-q3).*sin(q4).*4.698463103929542e-1-cos(q5).*(cos(q2-q3).*8.191520442889917e-1-sin(q2-q3).*sin(q4).*5.735764363510462e-1).*8.191520442889917e-1+sin(q2-q3).*cos(q4).*sin(q5).*8.191520442889917e-1).^2+(sin(q6).*(cos(q2-q3).*sin(q5).*8.191520442889917e-1+sin(q2-q3).*cos(q4).*cos(q5)-sin(q2-q3).*sin(q4).*sin(q5).*5.735764363510462e-1)-cos(q6).*(cos(q2-q3).*4.698463103929542e-1+sin(q2-q3).*sin(q4).*6.710100716628342e-1+cos(q5).*(cos(q2-q3).*8.191520442889917e-1-sin(q2-q3).*sin(q4).*5.735764363510462e-1).*5.735764363510462e-1-sin(q2-q3).*cos(q4).*sin(q5).*5.735764363510462e-1)).^2).*((sin(q6).*(cos(q2-q3).*sin(q5).*8.191520442889917e-1+sin(q2-q3).*cos(q4).*cos(q5)-sin(q2-q3).*sin(q4).*sin(q5).*5.735764363510462e-1)-cos(q6).*(cos(q2-q3).*4.698463103929542e-1+sin(q2-q3).*sin(q4).*6.710100716628342e-1+cos(q5).*(cos(q2-q3).*8.191520442889917e-1-sin(q2-q3).*sin(q4).*5.735764363510462e-1).*5.735764363510462e-1-sin(q2-q3).*cos(q4).*sin(q5).*5.735764363510462e-1)).*(cos(q6).*(sin(q5).*(cos(q2-q3).*8.191520442889917e-1-sin(q2-q3).*sin(q4).*5.735764363510462e-1).*5.735764363510462e-1+sin(q2-q3).*cos(q4).*cos(q5).*5.735764363510462e-1)-sin(q6).*(cos(q2-q3).*cos(q5).*(-8.191520442889917e-1)+sin(q2-q3).*cos(q4).*sin(q5)+sin(q2-q3).*cos(q5).*sin(q4).*5.735764363510462e-1)).*2.0+(sin(q5).*(cos(q2-q3).*8.191520442889917e-1-sin(q2-q3).*sin(q4).*5.735764363510462e-1).*8.191520442889917e-1+sin(q2-q3).*cos(q4).*cos(q5).*8.191520442889917e-1).*(cos(q2-q3).*3.289899283371657e-1+sin(q2-q3).*sin(q4).*4.698463103929542e-1-cos(q5).*(cos(q2-q3).*8.191520442889917e-1-sin(q2-q3).*sin(q4).*5.735764363510462e-1).*8.191520442889917e-1+sin(q2-q3).*cos(q4).*sin(q5).*8.191520442889917e-1).*2.0)).*(1.0./2.0)+real(cos(q6).*(cos(q2-q3).*cos(q5).*(-8.191520442889917e-1)+sin(q2-q3).*cos(q4).*sin(q5)+sin(q2-q3).*cos(q5).*sin(q4).*5.735764363510462e-1))).*(imag(dq6.*sin(q6).*(cos(q2-q3).*sin(q5).*8.191520442889917e-1+sin(q2-q3).*cos(q4).*cos(q5)-sin(q2-q3).*sin(q4).*sin(q5).*5.735764363510462e-1))+imag(cos(q6).*(dq5.*cos(q2-q3).*cos(q5).*(-8.191520442889917e-1)+sin(q2-q3).*sin(q5).*(dq2-dq3).*8.191520442889917e-1+dq4.*sin(q2-q3).*cos(q4).*sin(q5).*5.735764363510462e-1+dq4.*sin(q2-q3).*cos(q5).*sin(q4)+dq5.*sin(q2-q3).*cos(q4).*sin(q5)+dq5.*sin(q2-q3).*cos(q5).*sin(q4).*5.735764363510462e-1-cos(q2-q3).*cos(q4).*cos(q5).*(dq2-dq3)+cos(q2-q3).*sin(q4).*sin(q5).*(dq2-dq3).*5.735764363510462e-1))-imag(dq6.*cos(q6).*(cos(q2-q3).*4.698463103929542e-1+sin(q2-q3).*sin(q4).*6.710100716628342e-1+cos(q5).*(cos(q2-q3).*8.191520442889917e-1-sin(q2-q3).*sin(q4).*5.735764363510462e-1).*5.735764363510462e-1-sin(q2-q3).*cos(q4).*sin(q5).*5.735764363510462e-1))+imag(sin(q6).*(cos(q5).*(sin(q2-q3).*(dq2-dq3).*8.191520442889917e-1+dq4.*sin(q2-q3).*cos(q4).*5.735764363510462e-1+cos(q2-q3).*sin(q4).*(dq2-dq3).*5.735764363510462e-1).*5.735764363510462e-1+sin(q2-q3).*(dq2-dq3).*4.698463103929542e-1-dq4.*sin(q2-q3).*cos(q4).*6.710100716628342e-1-cos(q2-q3).*sin(q4).*(dq2-dq3).*6.710100716628342e-1+dq5.*sin(q5).*(cos(q2-q3).*8.191520442889917e-1-sin(q2-q3).*sin(q4).*5.735764363510462e-1).*5.735764363510462e-1+dq5.*sin(q2-q3).*cos(q4).*cos(q5).*5.735764363510462e-1-dq4.*sin(q2-q3).*sin(q4).*sin(q5).*5.735764363510462e-1+cos(q2-q3).*cos(q4).*sin(q5).*(dq2-dq3).*5.735764363510462e-1))-real(1.0./sqrt((cos(q2-q3).*3.289899283371657e-1+sin(q2-q3).*sin(q4).*4.698463103929542e-1-cos(q5).*(cos(q2-q3).*8.191520442889917e-1-sin(q2-q3).*sin(q4).*5.735764363510462e-1).*8.191520442889917e-1+sin(q2-q3).*cos(q4).*sin(q5).*8.191520442889917e-1).^2+(sin(q6).*(cos(q2-q3).*sin(q5).*8.191520442889917e-1+sin(q2-q3).*cos(q4).*cos(q5)-sin(q2-q3).*sin(q4).*sin(q5).*5.735764363510462e-1)-cos(q6).*(cos(q2-q3).*4.698463103929542e-1+sin(q2-q3).*sin(q4).*6.710100716628342e-1+cos(q5).*(cos(q2-q3).*8.191520442889917e-1-sin(q2-q3).*sin(q4).*5.735764363510462e-1).*5.735764363510462e-1-sin(q2-q3).*cos(q4).*sin(q5).*5.735764363510462e-1)).^2).*((sin(q6).*(cos(q2-q3).*sin(q5).*8.191520442889917e-1+sin(q2-q3).*cos(q4).*cos(q5)-sin(q2-q3).*sin(q4).*sin(q5).*5.735764363510462e-1)-cos(q6).*(cos(q2-q3).*4.698463103929542e-1+sin(q2-q3).*sin(q4).*6.710100716628342e-1+cos(q5).*(cos(q2-q3).*8.191520442889917e-1-sin(q2-q3).*sin(q4).*5.735764363510462e-1).*5.735764363510462e-1-sin(q2-q3).*cos(q4).*sin(q5).*5.735764363510462e-1)).*(cos(q6).*(cos(q5).*(sin(q2-q3).*(dq2-dq3).*8.191520442889917e-1+dq4.*sin(q2-q3).*cos(q4).*5.735764363510462e-1+cos(q2-q3).*sin(q4).*(dq2-dq3).*5.735764363510462e-1).*5.735764363510462e-1+sin(q2-q3).*(dq2-dq3).*4.698463103929542e-1-dq4.*sin(q2-q3).*cos(q4).*6.710100716628342e-1-cos(q2-q3).*sin(q4).*(dq2-dq3).*6.710100716628342e-1+dq5.*sin(q5).*(cos(q2-q3).*8.191520442889917e-1-sin(q2-q3).*sin(q4).*5.735764363510462e-1).*5.735764363510462e-1+dq5.*sin(q2-q3).*cos(q4).*cos(q5).*5.735764363510462e-1-dq4.*sin(q2-q3).*sin(q4).*sin(q5).*5.735764363510462e-1+cos(q2-q3).*cos(q4).*sin(q5).*(dq2-dq3).*5.735764363510462e-1)-sin(q6).*(dq5.*cos(q2-q3).*cos(q5).*(-8.191520442889917e-1)+sin(q2-q3).*sin(q5).*(dq2-dq3).*8.191520442889917e-1+dq4.*sin(q2-q3).*cos(q4).*sin(q5).*5.735764363510462e-1+dq4.*sin(q2-q3).*cos(q5).*sin(q4)+dq5.*sin(q2-q3).*cos(q4).*sin(q5)+dq5.*sin(q2-q3).*cos(q5).*sin(q4).*5.735764363510462e-1-cos(q2-q3).*cos(q4).*cos(q5).*(dq2-dq3)+cos(q2-q3).*sin(q4).*sin(q5).*(dq2-dq3).*5.735764363510462e-1)+dq6.*sin(q6).*(cos(q2-q3).*4.698463103929542e-1+sin(q2-q3).*sin(q4).*6.710100716628342e-1+cos(q5).*(cos(q2-q3).*8.191520442889917e-1-sin(q2-q3).*sin(q4).*5.735764363510462e-1).*5.735764363510462e-1-sin(q2-q3).*cos(q4).*sin(q5).*5.735764363510462e-1)+dq6.*cos(q6).*(cos(q2-q3).*sin(q5).*8.191520442889917e-1+sin(q2-q3).*cos(q4).*cos(q5)-sin(q2-q3).*sin(q4).*sin(q5).*5.735764363510462e-1)).*2.0+(cos(q2-q3).*3.289899283371657e-1+sin(q2-q3).*sin(q4).*4.698463103929542e-1-cos(q5).*(cos(q2-q3).*8.191520442889917e-1-sin(q2-q3).*sin(q4).*5.735764363510462e-1).*8.191520442889917e-1+sin(q2-q3).*cos(q4).*sin(q5).*8.191520442889917e-1).*(cos(q5).*(sin(q2-q3).*(dq2-dq3).*8.191520442889917e-1+dq4.*sin(q2-q3).*cos(q4).*5.735764363510462e-1+cos(q2-q3).*sin(q4).*(dq2-dq3).*5.735764363510462e-1).*8.191520442889917e-1-sin(q2-q3).*(dq2-dq3).*3.289899283371657e-1+dq4.*sin(q2-q3).*cos(q4).*4.698463103929542e-1+cos(q2-q3).*sin(q4).*(dq2-dq3).*4.698463103929542e-1+dq5.*sin(q5).*(cos(q2-q3).*8.191520442889917e-1-sin(q2-q3).*sin(q4).*5.735764363510462e-1).*8.191520442889917e-1+dq5.*sin(q2-q3).*cos(q4).*cos(q5).*8.191520442889917e-1-dq4.*sin(q2-q3).*sin(q4).*sin(q5).*8.191520442889917e-1+cos(q2-q3).*cos(q4).*sin(q5).*(dq2-dq3).*8.191520442889917e-1).*2.0)).*(1.0./2.0))-1.0./(imag(sin(q6).*(cos(q2-q3).*4.698463103929542e-1+sin(q2-q3).*sin(q4).*6.710100716628342e-1+cos(q5).*(cos(q2-q3).*8.191520442889917e-1-sin(q2-q3).*sin(q4).*5.735764363510462e-1).*5.735764363510462e-1-sin(q2-q3).*cos(q4).*sin(q5).*5.735764363510462e-1))+real(sqrt((cos(q2-q3).*3.289899283371657e-1+sin(q2-q3).*sin(q4).*4.698463103929542e-1-cos(q5).*(cos(q2-q3).*8.191520442889917e-1-sin(q2-q3).*sin(q4).*5.735764363510462e-1).*8.191520442889917e-1+sin(q2-q3).*cos(q4).*sin(q5).*8.191520442889917e-1).^2+(sin(q6).*(cos(q2-q3).*sin(q5).*8.191520442889917e-1+sin(q2-q3).*cos(q4).*cos(q5)-sin(q2-q3).*sin(q4).*sin(q5).*5.735764363510462e-1)-cos(q6).*(cos(q2-q3).*4.698463103929542e-1+sin(q2-q3).*sin(q4).*6.710100716628342e-1+cos(q5).*(cos(q2-q3).*8.191520442889917e-1-sin(q2-q3).*sin(q4).*5.735764363510462e-1).*5.735764363510462e-1-sin(q2-q3).*cos(q4).*sin(q5).*5.735764363510462e-1)).^2))+imag(cos(q6).*(cos(q2-q3).*sin(q5).*8.191520442889917e-1+sin(q2-q3).*cos(q4).*cos(q5)-sin(q2-q3).*sin(q4).*sin(q5).*5.735764363510462e-1))).^2.*(imag(sin(q6).*(sin(q5).*(cos(q2-q3).*8.191520442889917e-1-sin(q2-q3).*sin(q4).*5.735764363510462e-1).*5.735764363510462e-1+sin(q2-q3).*cos(q4).*cos(q5).*5.735764363510462e-1))+imag(cos(q6).*(cos(q2-q3).*cos(q5).*(-8.191520442889917e-1)+sin(q2-q3).*cos(q4).*sin(q5)+sin(q2-q3).*cos(q5).*sin(q4).*5.735764363510462e-1))-real(1.0./sqrt((cos(q2-q3).*3.289899283371657e-1+sin(q2-q3).*sin(q4).*4.698463103929542e-1-cos(q5).*(cos(q2-q3).*8.191520442889917e-1-sin(q2-q3).*sin(q4).*5.735764363510462e-1).*8.191520442889917e-1+sin(q2-q3).*cos(q4).*sin(q5).*8.191520442889917e-1).^2+(sin(q6).*(cos(q2-q3).*sin(q5).*8.191520442889917e-1+sin(q2-q3).*cos(q4).*cos(q5)-sin(q2-q3).*sin(q4).*sin(q5).*5.735764363510462e-1)-cos(q6).*(cos(q2-q3).*4.698463103929542e-1+sin(q2-q3).*sin(q4).*6.710100716628342e-1+cos(q5).*(cos(q2-q3).*8.191520442889917e-1-sin(q2-q3).*sin(q4).*5.735764363510462e-1).*5.735764363510462e-1-sin(q2-q3).*cos(q4).*sin(q5).*5.735764363510462e-1)).^2).*((sin(q6).*(cos(q2-q3).*sin(q5).*8.191520442889917e-1+sin(q2-q3).*cos(q4).*cos(q5)-sin(q2-q3).*sin(q4).*sin(q5).*5.735764363510462e-1)-cos(q6).*(cos(q2-q3).*4.698463103929542e-1+sin(q2-q3).*sin(q4).*6.710100716628342e-1+cos(q5).*(cos(q2-q3).*8.191520442889917e-1-sin(q2-q3).*sin(q4).*5.735764363510462e-1).*5.735764363510462e-1-sin(q2-q3).*cos(q4).*sin(q5).*5.735764363510462e-1)).*(cos(q6).*(sin(q5).*(cos(q2-q3).*8.191520442889917e-1-sin(q2-q3).*sin(q4).*5.735764363510462e-1).*5.735764363510462e-1+sin(q2-q3).*cos(q4).*cos(q5).*5.735764363510462e-1)-sin(q6).*(cos(q2-q3).*cos(q5).*(-8.191520442889917e-1)+sin(q2-q3).*cos(q4).*sin(q5)+sin(q2-q3).*cos(q5).*sin(q4).*5.735764363510462e-1)).*2.0+(sin(q5).*(cos(q2-q3).*8.191520442889917e-1-sin(q2-q3).*sin(q4).*5.735764363510462e-1).*8.191520442889917e-1+sin(q2-q3).*cos(q4).*cos(q5).*8.191520442889917e-1).*(cos(q2-q3).*3.289899283371657e-1+sin(q2-q3).*sin(q4).*4.698463103929542e-1-cos(q5).*(cos(q2-q3).*8.191520442889917e-1-sin(q2-q3).*sin(q4).*5.735764363510462e-1).*8.191520442889917e-1+sin(q2-q3).*cos(q4).*sin(q5).*8.191520442889917e-1).*2.0)).*(1.0./2.0)).*(real(dq6.*sin(q6).*(cos(q2-q3).*sin(q5).*8.191520442889917e-1+sin(q2-q3).*cos(q4).*cos(q5)-sin(q2-q3).*sin(q4).*sin(q5).*5.735764363510462e-1))+real(cos(q6).*(dq5.*cos(q2-q3).*cos(q5).*(-8.191520442889917e-1)+sin(q2-q3).*sin(q5).*(dq2-dq3).*8.191520442889917e-1+dq4.*sin(q2-q3).*cos(q4).*sin(q5).*5.735764363510462e-1+dq4.*sin(q2-q3).*cos(q5).*sin(q4)+dq5.*sin(q2-q3).*cos(q4).*sin(q5)+dq5.*sin(q2-q3).*cos(q5).*sin(q4).*5.735764363510462e-1-cos(q2-q3).*cos(q4).*cos(q5).*(dq2-dq3)+cos(q2-q3).*sin(q4).*sin(q5).*(dq2-dq3).*5.735764363510462e-1))-real(dq6.*cos(q6).*(cos(q2-q3).*4.698463103929542e-1+sin(q2-q3).*sin(q4).*6.710100716628342e-1+cos(q5).*(cos(q2-q3).*8.191520442889917e-1-sin(q2-q3).*sin(q4).*5.735764363510462e-1).*5.735764363510462e-1-sin(q2-q3).*cos(q4).*sin(q5).*5.735764363510462e-1))+real(sin(q6).*(cos(q5).*(sin(q2-q3).*(dq2-dq3).*8.191520442889917e-1+dq4.*sin(q2-q3).*cos(q4).*5.735764363510462e-1+cos(q2-q3).*sin(q4).*(dq2-dq3).*5.735764363510462e-1).*5.735764363510462e-1+sin(q2-q3).*(dq2-dq3).*4.698463103929542e-1-dq4.*sin(q2-q3).*cos(q4).*6.710100716628342e-1-cos(q2-q3).*sin(q4).*(dq2-dq3).*6.710100716628342e-1+dq5.*sin(q5).*(cos(q2-q3).*8.191520442889917e-1-sin(q2-q3).*sin(q4).*5.735764363510462e-1).*5.735764363510462e-1+dq5.*sin(q2-q3).*cos(q4).*cos(q5).*5.735764363510462e-1-dq4.*sin(q2-q3).*sin(q4).*sin(q5).*5.735764363510462e-1+cos(q2-q3).*cos(q4).*sin(q5).*(dq2-dq3).*5.735764363510462e-1))+imag(1.0./sqrt((cos(q2-q3).*3.289899283371657e-1+sin(q2-q3).*sin(q4).*4.698463103929542e-1-cos(q5).*(cos(q2-q3).*8.191520442889917e-1-sin(q2-q3).*sin(q4).*5.735764363510462e-1).*8.191520442889917e-1+sin(q2-q3).*cos(q4).*sin(q5).*8.191520442889917e-1).^2+(sin(q6).*(cos(q2-q3).*sin(q5).*8.191520442889917e-1+sin(q2-q3).*cos(q4).*cos(q5)-sin(q2-q3).*sin(q4).*sin(q5).*5.735764363510462e-1)-cos(q6).*(cos(q2-q3).*4.698463103929542e-1+sin(q2-q3).*sin(q4).*6.710100716628342e-1+cos(q5).*(cos(q2-q3).*8.191520442889917e-1-sin(q2-q3).*sin(q4).*5.735764363510462e-1).*5.735764363510462e-1-sin(q2-q3).*cos(q4).*sin(q5).*5.735764363510462e-1)).^2).*((sin(q6).*(cos(q2-q3).*sin(q5).*8.191520442889917e-1+sin(q2-q3).*cos(q4).*cos(q5)-sin(q2-q3).*sin(q4).*sin(q5).*5.735764363510462e-1)-cos(q6).*(cos(q2-q3).*4.698463103929542e-1+sin(q2-q3).*sin(q4).*6.710100716628342e-1+cos(q5).*(cos(q2-q3).*8.191520442889917e-1-sin(q2-q3).*sin(q4).*5.735764363510462e-1).*5.735764363510462e-1-sin(q2-q3).*cos(q4).*sin(q5).*5.735764363510462e-1)).*(cos(q6).*(cos(q5).*(sin(q2-q3).*(dq2-dq3).*8.191520442889917e-1+dq4.*sin(q2-q3).*cos(q4).*5.735764363510462e-1+cos(q2-q3).*sin(q4).*(dq2-dq3).*5.735764363510462e-1).*5.735764363510462e-1+sin(q2-q3).*(dq2-dq3).*4.698463103929542e-1-dq4.*sin(q2-q3).*cos(q4).*6.710100716628342e-1-cos(q2-q3).*sin(q4).*(dq2-dq3).*6.710100716628342e-1+dq5.*sin(q5).*(cos(q2-q3).*8.191520442889917e-1-sin(q2-q3).*sin(q4).*5.735764363510462e-1).*5.735764363510462e-1+dq5.*sin(q2-q3).*cos(q4).*cos(q5).*5.735764363510462e-1-dq4.*sin(q2-q3).*sin(q4).*sin(q5).*5.735764363510462e-1+cos(q2-q3).*cos(q4).*sin(q5).*(dq2-dq3).*5.735764363510462e-1)-sin(q6).*(dq5.*cos(q2-q3).*cos(q5).*(-8.191520442889917e-1)+sin(q2-q3).*sin(q5).*(dq2-dq3).*8.191520442889917e-1+dq4.*sin(q2-q3).*cos(q4).*sin(q5).*5.735764363510462e-1+dq4.*sin(q2-q3).*cos(q5).*sin(q4)+dq5.*sin(q2-q3).*cos(q4).*sin(q5)+dq5.*sin(q2-q3).*cos(q5).*sin(q4).*5.735764363510462e-1-cos(q2-q3).*cos(q4).*cos(q5).*(dq2-dq3)+cos(q2-q3).*sin(q4).*sin(q5).*(dq2-dq3).*5.735764363510462e-1)+dq6.*sin(q6).*(cos(q2-q3).*4.698463103929542e-1+sin(q2-q3).*sin(q4).*6.710100716628342e-1+cos(q5).*(cos(q2-q3).*8.191520442889917e-1-sin(q2-q3).*sin(q4).*5.735764363510462e-1).*5.735764363510462e-1-sin(q2-q3).*cos(q4).*sin(q5).*5.735764363510462e-1)+dq6.*cos(q6).*(cos(q2-q3).*sin(q5).*8.191520442889917e-1+sin(q2-q3).*cos(q4).*cos(q5)-sin(q2-q3).*sin(q4).*sin(q5).*5.735764363510462e-1)).*2.0+(cos(q2-q3).*3.289899283371657e-1+sin(q2-q3).*sin(q4).*4.698463103929542e-1-cos(q5).*(cos(q2-q3).*8.191520442889917e-1-sin(q2-q3).*sin(q4).*5.735764363510462e-1).*8.191520442889917e-1+sin(q2-q3).*cos(q4).*sin(q5).*8.191520442889917e-1).*(cos(q5).*(sin(q2-q3).*(dq2-dq3).*8.191520442889917e-1+dq4.*sin(q2-q3).*cos(q4).*5.735764363510462e-1+cos(q2-q3).*sin(q4).*(dq2-dq3).*5.735764363510462e-1).*8.191520442889917e-1-sin(q2-q3).*(dq2-dq3).*3.289899283371657e-1+dq4.*sin(q2-q3).*cos(q4).*4.698463103929542e-1+cos(q2-q3).*sin(q4).*(dq2-dq3).*4.698463103929542e-1+dq5.*sin(q5).*(cos(q2-q3).*8.191520442889917e-1-sin(q2-q3).*sin(q4).*5.735764363510462e-1).*8.191520442889917e-1+dq5.*sin(q2-q3).*cos(q4).*cos(q5).*8.191520442889917e-1-dq4.*sin(q2-q3).*sin(q4).*sin(q5).*8.191520442889917e-1+cos(q2-q3).*cos(q4).*sin(q5).*(dq2-dq3).*8.191520442889917e-1).*2.0)).*(1.0./2.0))+1.0./(imag(sin(q6).*(cos(q2-q3).*4.698463103929542e-1+sin(q2-q3).*sin(q4).*6.710100716628342e-1+cos(q5).*(cos(q2-q3).*8.191520442889917e-1-sin(q2-q3).*sin(q4).*5.735764363510462e-1).*5.735764363510462e-1-sin(q2-q3).*cos(q4).*sin(q5).*5.735764363510462e-1))+real(sqrt((cos(q2-q3).*3.289899283371657e-1+sin(q2-q3).*sin(q4).*4.698463103929542e-1-cos(q5).*(cos(q2-q3).*8.191520442889917e-1-sin(q2-q3).*sin(q4).*5.735764363510462e-1).*8.191520442889917e-1+sin(q2-q3).*cos(q4).*sin(q5).*8.191520442889917e-1).^2+(sin(q6).*(cos(q2-q3).*sin(q5).*8.191520442889917e-1+sin(q2-q3).*cos(q4).*cos(q5)-sin(q2-q3).*sin(q4).*sin(q5).*5.735764363510462e-1)-cos(q6).*(cos(q2-q3).*4.698463103929542e-1+sin(q2-q3).*sin(q4).*6.710100716628342e-1+cos(q5).*(cos(q2-q3).*8.191520442889917e-1-sin(q2-q3).*sin(q4).*5.735764363510462e-1).*5.735764363510462e-1-sin(q2-q3).*cos(q4).*sin(q5).*5.735764363510462e-1)).^2))+imag(cos(q6).*(cos(q2-q3).*sin(q5).*8.191520442889917e-1+sin(q2-q3).*cos(q4).*cos(q5)-sin(q2-q3).*sin(q4).*sin(q5).*5.735764363510462e-1))).^3.*(imag(sin(q6).*(sin(q5).*(cos(q2-q3).*8.191520442889917e-1-sin(q2-q3).*sin(q4).*5.735764363510462e-1).*5.735764363510462e-1+sin(q2-q3).*cos(q4).*cos(q5).*5.735764363510462e-1))+imag(cos(q6).*(cos(q2-q3).*cos(q5).*(-8.191520442889917e-1)+sin(q2-q3).*cos(q4).*sin(q5)+sin(q2-q3).*cos(q5).*sin(q4).*5.735764363510462e-1))-real(1.0./sqrt((cos(q2-q3).*3.289899283371657e-1+sin(q2-q3).*sin(q4).*4.698463103929542e-1-cos(q5).*(cos(q2-q3).*8.191520442889917e-1-sin(q2-q3).*sin(q4).*5.735764363510462e-1).*8.191520442889917e-1+sin(q2-q3).*cos(q4).*sin(q5).*8.191520442889917e-1).^2+(sin(q6).*(cos(q2-q3).*sin(q5).*8.191520442889917e-1+sin(q2-q3).*cos(q4).*cos(q5)-sin(q2-q3).*sin(q4).*sin(q5).*5.735764363510462e-1)-cos(q6).*(cos(q2-q3).*4.698463103929542e-1+sin(q2-q3).*sin(q4).*6.710100716628342e-1+cos(q5).*(cos(q2-q3).*8.191520442889917e-1-sin(q2-q3).*sin(q4).*5.735764363510462e-1).*5.735764363510462e-1-sin(q2-q3).*cos(q4).*sin(q5).*5.735764363510462e-1)).^2).*((sin(q6).*(cos(q2-q3).*sin(q5).*8.191520442889917e-1+sin(q2-q3).*cos(q4).*cos(q5)-sin(q2-q3).*sin(q4).*sin(q5).*5.735764363510462e-1)-cos(q6).*(cos(q2-q3).*4.698463103929542e-1+sin(q2-q3).*sin(q4).*6.710100716628342e-1+cos(q5).*(cos(q2-q3).*8.191520442889917e-1-sin(q2-q3).*sin(q4).*5.735764363510462e-1).*5.735764363510462e-1-sin(q2-q3).*cos(q4).*sin(q5).*5.735764363510462e-1)).*(cos(q6).*(sin(q5).*(cos(q2-q3).*8.191520442889917e-1-sin(q2-q3).*sin(q4).*5.735764363510462e-1).*5.735764363510462e-1+sin(q2-q3).*cos(q4).*cos(q5).*5.735764363510462e-1)-sin(q6).*(cos(q2-q3).*cos(q5).*(-8.191520442889917e-1)+sin(q2-q3).*cos(q4).*sin(q5)+sin(q2-q3).*cos(q5).*sin(q4).*5.735764363510462e-1)).*2.0+(sin(q5).*(cos(q2-q3).*8.191520442889917e-1-sin(q2-q3).*sin(q4).*5.735764363510462e-1).*8.191520442889917e-1+sin(q2-q3).*cos(q4).*cos(q5).*8.191520442889917e-1).*(cos(q2-q3).*3.289899283371657e-1+sin(q2-q3).*sin(q4).*4.698463103929542e-1-cos(q5).*(cos(q2-q3).*8.191520442889917e-1-sin(q2-q3).*sin(q4).*5.735764363510462e-1).*8.191520442889917e-1+sin(q2-q3).*cos(q4).*sin(q5).*8.191520442889917e-1).*2.0)).*(1.0./2.0)).*(real(sin(q6).*(cos(q2-q3).*4.698463103929542e-1+sin(q2-q3).*sin(q4).*6.710100716628342e-1+cos(q5).*(cos(q2-q3).*8.191520442889917e-1-sin(q2-q3).*sin(q4).*5.735764363510462e-1).*5.735764363510462e-1-sin(q2-q3).*cos(q4).*sin(q5).*5.735764363510462e-1))-imag(sqrt((cos(q2-q3).*3.289899283371657e-1+sin(q2-q3).*sin(q4).*4.698463103929542e-1-cos(q5).*(cos(q2-q3).*8.191520442889917e-1-sin(q2-q3).*sin(q4).*5.735764363510462e-1).*8.191520442889917e-1+sin(q2-q3).*cos(q4).*sin(q5).*8.191520442889917e-1).^2+(sin(q6).*(cos(q2-q3).*sin(q5).*8.191520442889917e-1+sin(q2-q3).*cos(q4).*cos(q5)-sin(q2-q3).*sin(q4).*sin(q5).*5.735764363510462e-1)-cos(q6).*(cos(q2-q3).*4.698463103929542e-1+sin(q2-q3).*sin(q4).*6.710100716628342e-1+cos(q5).*(cos(q2-q3).*8.191520442889917e-1-sin(q2-q3).*sin(q4).*5.735764363510462e-1).*5.735764363510462e-1-sin(q2-q3).*cos(q4).*sin(q5).*5.735764363510462e-1)).^2))+real(cos(q6).*(cos(q2-q3).*sin(q5).*8.191520442889917e-1+sin(q2-q3).*cos(q4).*cos(q5)-sin(q2-q3).*sin(q4).*sin(q5).*5.735764363510462e-1))).*(imag(dq6.*sin(q6).*(cos(q2-q3).*sin(q5).*8.191520442889917e-1+sin(q2-q3).*cos(q4).*cos(q5)-sin(q2-q3).*sin(q4).*sin(q5).*5.735764363510462e-1))+imag(cos(q6).*(dq5.*cos(q2-q3).*cos(q5).*(-8.191520442889917e-1)+sin(q2-q3).*sin(q5).*(dq2-dq3).*8.191520442889917e-1+dq4.*sin(q2-q3).*cos(q4).*sin(q5).*5.735764363510462e-1+dq4.*sin(q2-q3).*cos(q5).*sin(q4)+dq5.*sin(q2-q3).*cos(q4).*sin(q5)+dq5.*sin(q2-q3).*cos(q5).*sin(q4).*5.735764363510462e-1-cos(q2-q3).*cos(q4).*cos(q5).*(dq2-dq3)+cos(q2-q3).*sin(q4).*sin(q5).*(dq2-dq3).*5.735764363510462e-1))-imag(dq6.*cos(q6).*(cos(q2-q3).*4.698463103929542e-1+sin(q2-q3).*sin(q4).*6.710100716628342e-1+cos(q5).*(cos(q2-q3).*8.191520442889917e-1-sin(q2-q3).*sin(q4).*5.735764363510462e-1).*5.735764363510462e-1-sin(q2-q3).*cos(q4).*sin(q5).*5.735764363510462e-1))+imag(sin(q6).*(cos(q5).*(sin(q2-q3).*(dq2-dq3).*8.191520442889917e-1+dq4.*sin(q2-q3).*cos(q4).*5.735764363510462e-1+cos(q2-q3).*sin(q4).*(dq2-dq3).*5.735764363510462e-1).*5.735764363510462e-1+sin(q2-q3).*(dq2-dq3).*4.698463103929542e-1-dq4.*sin(q2-q3).*cos(q4).*6.710100716628342e-1-cos(q2-q3).*sin(q4).*(dq2-dq3).*6.710100716628342e-1+dq5.*sin(q5).*(cos(q2-q3).*8.191520442889917e-1-sin(q2-q3).*sin(q4).*5.735764363510462e-1).*5.735764363510462e-1+dq5.*sin(q2-q3).*cos(q4).*cos(q5).*5.735764363510462e-1-dq4.*sin(q2-q3).*sin(q4).*sin(q5).*5.735764363510462e-1+cos(q2-q3).*cos(q4).*sin(q5).*(dq2-dq3).*5.735764363510462e-1))-real(1.0./sqrt((cos(q2-q3).*3.289899283371657e-1+sin(q2-q3).*sin(q4).*4.698463103929542e-1-cos(q5).*(cos(q2-q3).*8.191520442889917e-1-sin(q2-q3).*sin(q4).*5.735764363510462e-1).*8.191520442889917e-1+sin(q2-q3).*cos(q4).*sin(q5).*8.191520442889917e-1).^2+(sin(q6).*(cos(q2-q3).*sin(q5).*8.191520442889917e-1+sin(q2-q3).*cos(q4).*cos(q5)-sin(q2-q3).*sin(q4).*sin(q5).*5.735764363510462e-1)-cos(q6).*(cos(q2-q3).*4.698463103929542e-1+sin(q2-q3).*sin(q4).*6.710100716628342e-1+cos(q5).*(cos(q2-q3).*8.191520442889917e-1-sin(q2-q3).*sin(q4).*5.735764363510462e-1).*5.735764363510462e-1-sin(q2-q3).*cos(q4).*sin(q5).*5.735764363510462e-1)).^2).*((sin(q6).*(cos(q2-q3).*sin(q5).*8.191520442889917e-1+sin(q2-q3).*cos(q4).*cos(q5)-sin(q2-q3).*sin(q4).*sin(q5).*5.735764363510462e-1)-cos(q6).*(cos(q2-q3).*4.698463103929542e-1+sin(q2-q3).*sin(q4).*6.710100716628342e-1+cos(q5).*(cos(q2-q3).*8.191520442889917e-1-sin(q2-q3).*sin(q4).*5.735764363510462e-1).*5.735764363510462e-1-sin(q2-q3).*cos(q4).*sin(q5).*5.735764363510462e-1)).*(cos(q6).*(cos(q5).*(sin(q2-q3).*(dq2-dq3).*8.191520442889917e-1+dq4.*sin(q2-q3).*cos(q4).*5.735764363510462e-1+cos(q2-q3).*sin(q4).*(dq2-dq3).*5.735764363510462e-1).*5.735764363510462e-1+sin(q2-q3).*(dq2-dq3).*4.698463103929542e-1-dq4.*sin(q2-q3).*cos(q4).*6.710100716628342e-1-cos(q2-q3).*sin(q4).*(dq2-dq3).*6.710100716628342e-1+dq5.*sin(q5).*(cos(q2-q3).*8.191520442889917e-1-sin(q2-q3).*sin(q4).*5.735764363510462e-1).*5.735764363510462e-1+dq5.*sin(q2-q3).*cos(q4).*cos(q5).*5.735764363510462e-1-dq4.*sin(q2-q3).*sin(q4).*sin(q5).*5.735764363510462e-1+cos(q2-q3).*cos(q4).*sin(q5).*(dq2-dq3).*5.735764363510462e-1)-sin(q6).*(dq5.*cos(q2-q3).*cos(q5).*(-8.191520442889917e-1)+sin(q2-q3).*sin(q5).*(dq2-dq3).*8.191520442889917e-1+dq4.*sin(q2-q3).*cos(q4).*sin(q5).*5.735764363510462e-1+dq4.*sin(q2-q3).*cos(q5).*sin(q4)+dq5.*sin(q2-q3).*cos(q4).*sin(q5)+dq5.*sin(q2-q3).*cos(q5).*sin(q4).*5.735764363510462e-1-cos(q2-q3).*cos(q4).*cos(q5).*(dq2-dq3)+cos(q2-q3).*sin(q4).*sin(q5).*(dq2-dq3).*5.735764363510462e-1)+dq6.*sin(q6).*(cos(q2-q3).*4.698463103929542e-1+sin(q2-q3).*sin(q4).*6.710100716628342e-1+cos(q5).*(cos(q2-q3).*8.191520442889917e-1-sin(q2-q3).*sin(q4).*5.735764363510462e-1).*5.735764363510462e-1-sin(q2-q3).*cos(q4).*sin(q5).*5.735764363510462e-1)+dq6.*cos(q6).*(cos(q2-q3).*sin(q5).*8.191520442889917e-1+sin(q2-q3).*cos(q4).*cos(q5)-sin(q2-q3).*sin(q4).*sin(q5).*5.735764363510462e-1)).*2.0+(cos(q2-q3).*3.289899283371657e-1+sin(q2-q3).*sin(q4).*4.698463103929542e-1-cos(q5).*(cos(q2-q3).*8.191520442889917e-1-sin(q2-q3).*sin(q4).*5.735764363510462e-1).*8.191520442889917e-1+sin(q2-q3).*cos(q4).*sin(q5).*8.191520442889917e-1).*(cos(q5).*(sin(q2-q3).*(dq2-dq3).*8.191520442889917e-1+dq4.*sin(q2-q3).*cos(q4).*5.735764363510462e-1+cos(q2-q3).*sin(q4).*(dq2-dq3).*5.735764363510462e-1).*8.191520442889917e-1-sin(q2-q3).*(dq2-dq3).*3.289899283371657e-1+dq4.*sin(q2-q3).*cos(q4).*4.698463103929542e-1+cos(q2-q3).*sin(q4).*(dq2-dq3).*4.698463103929542e-1+dq5.*sin(q5).*(cos(q2-q3).*8.191520442889917e-1-sin(q2-q3).*sin(q4).*5.735764363510462e-1).*8.191520442889917e-1+dq5.*sin(q2-q3).*cos(q4).*cos(q5).*8.191520442889917e-1-dq4.*sin(q2-q3).*sin(q4).*sin(q5).*8.191520442889917e-1+cos(q2-q3).*cos(q4).*sin(q5).*(dq2-dq3).*8.191520442889917e-1).*2.0)).*(1.0./2.0)).*2.0))./((real(sin(q6).*(cos(q2-q3).*4.698463103929542e-1+sin(q2-q3).*sin(q4).*6.710100716628342e-1+cos(q5).*(cos(q2-q3).*8.191520442889917e-1-sin(q2-q3).*sin(q4).*5.735764363510462e-1).*5.735764363510462e-1-sin(q2-q3).*cos(q4).*sin(q5).*5.735764363510462e-1))-imag(sqrt((cos(q2-q3).*3.289899283371657e-1+sin(q2-q3).*sin(q4).*4.698463103929542e-1-cos(q5).*(cos(q2-q3).*8.191520442889917e-1-sin(q2-q3).*sin(q4).*5.735764363510462e-1).*8.191520442889917e-1+sin(q2-q3).*cos(q4).*sin(q5).*8.191520442889917e-1).^2+(sin(q6).*(cos(q2-q3).*sin(q5).*8.191520442889917e-1+sin(q2-q3).*cos(q4).*cos(q5)-sin(q2-q3).*sin(q4).*sin(q5).*5.735764363510462e-1)-cos(q6).*(cos(q2-q3).*4.698463103929542e-1+sin(q2-q3).*sin(q4).*6.710100716628342e-1+cos(q5).*(cos(q2-q3).*8.191520442889917e-1-sin(q2-q3).*sin(q4).*5.735764363510462e-1).*5.735764363510462e-1-sin(q2-q3).*cos(q4).*sin(q5).*5.735764363510462e-1)).^2))+real(cos(q6).*(cos(q2-q3).*sin(q5).*8.191520442889917e-1+sin(q2-q3).*cos(q4).*cos(q5)-sin(q2-q3).*sin(q4).*sin(q5).*5.735764363510462e-1))).^2+(imag(sin(q6).*(cos(q2-q3).*4.698463103929542e-1+sin(q2-q3).*sin(q4).*6.710100716628342e-1+cos(q5).*(cos(q2-q3).*8.191520442889917e-1-sin(q2-q3).*sin(q4).*5.735764363510462e-1).*5.735764363510462e-1-sin(q2-q3).*cos(q4).*sin(q5).*5.735764363510462e-1))+real(sqrt((cos(q2-q3).*3.289899283371657e-1+sin(q2-q3).*sin(q4).*4.698463103929542e-1-cos(q5).*(cos(q2-q3).*8.191520442889917e-1-sin(q2-q3).*sin(q4).*5.735764363510462e-1).*8.191520442889917e-1+sin(q2-q3).*cos(q4).*sin(q5).*8.191520442889917e-1).^2+(sin(q6).*(cos(q2-q3).*sin(q5).*8.191520442889917e-1+sin(q2-q3).*cos(q4).*cos(q5)-sin(q2-q3).*sin(q4).*sin(q5).*5.735764363510462e-1)-cos(q6).*(cos(q2-q3).*4.698463103929542e-1+sin(q2-q3).*sin(q4).*6.710100716628342e-1+cos(q5).*(cos(q2-q3).*8.191520442889917e-1-sin(q2-q3).*sin(q4).*5.735764363510462e-1).*5.735764363510462e-1-sin(q2-q3).*cos(q4).*sin(q5).*5.735764363510462e-1)).^2))+imag(cos(q6).*(cos(q2-q3).*sin(q5).*8.191520442889917e-1+sin(q2-q3).*cos(q4).*cos(q5)-sin(q2-q3).*sin(q4).*sin(q5).*5.735764363510462e-1))).^2)+((real(sin(q6).*(cos(q2-q3).*4.698463103929542e-1+sin(q2-q3).*sin(q4).*6.710100716628342e-1+cos(q5).*(cos(q2-q3).*8.191520442889917e-1-sin(q2-q3).*sin(q4).*5.735764363510462e-1).*5.735764363510462e-1-sin(q2-q3).*cos(q4).*sin(q5).*5.735764363510462e-1))-imag(sqrt((cos(q2-q3).*3.289899283371657e-1+sin(q2-q3).*sin(q4).*4.698463103929542e-1-cos(q5).*(cos(q2-q3).*8.191520442889917e-1-sin(q2-q3).*sin(q4).*5.735764363510462e-1).*8.191520442889917e-1+sin(q2-q3).*cos(q4).*sin(q5).*8.191520442889917e-1).^2+(sin(q6).*(cos(q2-q3).*sin(q5).*8.191520442889917e-1+sin(q2-q3).*cos(q4).*cos(q5)-sin(q2-q3).*sin(q4).*sin(q5).*5.735764363510462e-1)-cos(q6).*(cos(q2-q3).*4.698463103929542e-1+sin(q2-q3).*sin(q4).*6.710100716628342e-1+cos(q5).*(cos(q2-q3).*8.191520442889917e-1-sin(q2-q3).*sin(q4).*5.735764363510462e-1).*5.735764363510462e-1-sin(q2-q3).*cos(q4).*sin(q5).*5.735764363510462e-1)).^2))+real(cos(q6).*(cos(q2-q3).*sin(q5).*8.191520442889917e-1+sin(q2-q3).*cos(q4).*cos(q5)-sin(q2-q3).*sin(q4).*sin(q5).*5.735764363510462e-1))).*(real(dq6.*sin(q6).*(cos(q2-q3).*sin(q5).*8.191520442889917e-1+sin(q2-q3).*cos(q4).*cos(q5)-sin(q2-q3).*sin(q4).*sin(q5).*5.735764363510462e-1))+real(cos(q6).*(dq5.*cos(q2-q3).*cos(q5).*(-8.191520442889917e-1)+sin(q2-q3).*sin(q5).*(dq2-dq3).*8.191520442889917e-1+dq4.*sin(q2-q3).*cos(q4).*sin(q5).*5.735764363510462e-1+dq4.*sin(q2-q3).*cos(q5).*sin(q4)+dq5.*sin(q2-q3).*cos(q4).*sin(q5)+dq5.*sin(q2-q3).*cos(q5).*sin(q4).*5.735764363510462e-1-cos(q2-q3).*cos(q4).*cos(q5).*(dq2-dq3)+cos(q2-q3).*sin(q4).*sin(q5).*(dq2-dq3).*5.735764363510462e-1))-real(dq6.*cos(q6).*(cos(q2-q3).*4.698463103929542e-1+sin(q2-q3).*sin(q4).*6.710100716628342e-1+cos(q5).*(cos(q2-q3).*8.191520442889917e-1-sin(q2-q3).*sin(q4).*5.735764363510462e-1).*5.735764363510462e-1-sin(q2-q3).*cos(q4).*sin(q5).*5.735764363510462e-1))+real(sin(q6).*(cos(q5).*(sin(q2-q3).*(dq2-dq3).*8.191520442889917e-1+dq4.*sin(q2-q3).*cos(q4).*5.735764363510462e-1+cos(q2-q3).*sin(q4).*(dq2-dq3).*5.735764363510462e-1).*5.735764363510462e-1+sin(q2-q3).*(dq2-dq3).*4.698463103929542e-1-dq4.*sin(q2-q3).*cos(q4).*6.710100716628342e-1-cos(q2-q3).*sin(q4).*(dq2-dq3).*6.710100716628342e-1+dq5.*sin(q5).*(cos(q2-q3).*8.191520442889917e-1-sin(q2-q3).*sin(q4).*5.735764363510462e-1).*5.735764363510462e-1+dq5.*sin(q2-q3).*cos(q4).*cos(q5).*5.735764363510462e-1-dq4.*sin(q2-q3).*sin(q4).*sin(q5).*5.735764363510462e-1+cos(q2-q3).*cos(q4).*sin(q5).*(dq2-dq3).*5.735764363510462e-1))+imag(1.0./sqrt((cos(q2-q3).*3.289899283371657e-1+sin(q2-q3).*sin(q4).*4.698463103929542e-1-cos(q5).*(cos(q2-q3).*8.191520442889917e-1-sin(q2-q3).*sin(q4).*5.735764363510462e-1).*8.191520442889917e-1+sin(q2-q3).*cos(q4).*sin(q5).*8.191520442889917e-1).^2+(sin(q6).*(cos(q2-q3).*sin(q5).*8.191520442889917e-1+sin(q2-q3).*cos(q4).*cos(q5)-sin(q2-q3).*sin(q4).*sin(q5).*5.735764363510462e-1)-cos(q6).*(cos(q2-q3).*4.698463103929542e-1+sin(q2-q3).*sin(q4).*6.710100716628342e-1+cos(q5).*(cos(q2-q3).*8.191520442889917e-1-sin(q2-q3).*sin(q4).*5.735764363510462e-1).*5.735764363510462e-1-sin(q2-q3).*cos(q4).*sin(q5).*5.735764363510462e-1)).^2).*((sin(q6).*(cos(q2-q3).*sin(q5).*8.191520442889917e-1+sin(q2-q3).*cos(q4).*cos(q5)-sin(q2-q3).*sin(q4).*sin(q5).*5.735764363510462e-1)-cos(q6).*(cos(q2-q3).*4.698463103929542e-1+sin(q2-q3).*sin(q4).*6.710100716628342e-1+cos(q5).*(cos(q2-q3).*8.191520442889917e-1-sin(q2-q3).*sin(q4).*5.735764363510462e-1).*5.735764363510462e-1-sin(q2-q3).*cos(q4).*sin(q5).*5.735764363510462e-1)).*(cos(q6).*(cos(q5).*(sin(q2-q3).*(dq2-dq3).*8.191520442889917e-1+dq4.*sin(q2-q3).*cos(q4).*5.735764363510462e-1+cos(q2-q3).*sin(q4).*(dq2-dq3).*5.735764363510462e-1).*5.735764363510462e-1+sin(q2-q3).*(dq2-dq3).*4.698463103929542e-1-dq4.*sin(q2-q3).*cos(q4).*6.710100716628342e-1-cos(q2-q3).*sin(q4).*(dq2-dq3).*6.710100716628342e-1+dq5.*sin(q5).*(cos(q2-q3).*8.191520442889917e-1-sin(q2-q3).*sin(q4).*5.735764363510462e-1).*5.735764363510462e-1+dq5.*sin(q2-q3).*cos(q4).*cos(q5).*5.735764363510462e-1-dq4.*sin(q2-q3).*sin(q4).*sin(q5).*5.735764363510462e-1+cos(q2-q3).*cos(q4).*sin(q5).*(dq2-dq3).*5.735764363510462e-1)-sin(q6).*(dq5.*cos(q2-q3).*cos(q5).*(-8.191520442889917e-1)+sin(q2-q3).*sin(q5).*(dq2-dq3).*8.191520442889917e-1+dq4.*sin(q2-q3).*cos(q4).*sin(q5).*5.735764363510462e-1+dq4.*sin(q2-q3).*cos(q5).*sin(q4)+dq5.*sin(q2-q3).*cos(q4).*sin(q5)+dq5.*sin(q2-q3).*cos(q5).*sin(q4).*5.735764363510462e-1-cos(q2-q3).*cos(q4).*cos(q5).*(dq2-dq3)+cos(q2-q3).*sin(q4).*sin(q5).*(dq2-dq3).*5.735764363510462e-1)+dq6.*sin(q6).*(cos(q2-q3).*4.698463103929542e-1+sin(q2-q3).*sin(q4).*6.710100716628342e-1+cos(q5).*(cos(q2-q3).*8.191520442889917e-1-sin(q2-q3).*sin(q4).*5.735764363510462e-1).*5.735764363510462e-1-sin(q2-q3).*cos(q4).*sin(q5).*5.735764363510462e-1)+dq6.*cos(q6).*(cos(q2-q3).*sin(q5).*8.191520442889917e-1+sin(q2-q3).*cos(q4).*cos(q5)-sin(q2-q3).*sin(q4).*sin(q5).*5.735764363510462e-1)).*2.0+(cos(q2-q3).*3.289899283371657e-1+sin(q2-q3).*sin(q4).*4.698463103929542e-1-cos(q5).*(cos(q2-q3).*8.191520442889917e-1-sin(q2-q3).*sin(q4).*5.735764363510462e-1).*8.191520442889917e-1+sin(q2-q3).*cos(q4).*sin(q5).*8.191520442889917e-1).*(cos(q5).*(sin(q2-q3).*(dq2-dq3).*8.191520442889917e-1+dq4.*sin(q2-q3).*cos(q4).*5.735764363510462e-1+cos(q2-q3).*sin(q4).*(dq2-dq3).*5.735764363510462e-1).*8.191520442889917e-1-sin(q2-q3).*(dq2-dq3).*3.289899283371657e-1+dq4.*sin(q2-q3).*cos(q4).*4.698463103929542e-1+cos(q2-q3).*sin(q4).*(dq2-dq3).*4.698463103929542e-1+dq5.*sin(q5).*(cos(q2-q3).*8.191520442889917e-1-sin(q2-q3).*sin(q4).*5.735764363510462e-1).*8.191520442889917e-1+dq5.*sin(q2-q3).*cos(q4).*cos(q5).*8.191520442889917e-1-dq4.*sin(q2-q3).*sin(q4).*sin(q5).*8.191520442889917e-1+cos(q2-q3).*cos(q4).*sin(q5).*(dq2-dq3).*8.191520442889917e-1).*2.0)).*(1.0./2.0)).*2.0+(imag(sin(q6).*(cos(q2-q3).*4.698463103929542e-1+sin(q2-q3).*sin(q4).*6.710100716628342e-1+cos(q5).*(cos(q2-q3).*8.191520442889917e-1-sin(q2-q3).*sin(q4).*5.735764363510462e-1).*5.735764363510462e-1-sin(q2-q3).*cos(q4).*sin(q5).*5.735764363510462e-1))+real(sqrt((cos(q2-q3).*3.289899283371657e-1+sin(q2-q3).*sin(q4).*4.698463103929542e-1-cos(q5).*(cos(q2-q3).*8.191520442889917e-1-sin(q2-q3).*sin(q4).*5.735764363510462e-1).*8.191520442889917e-1+sin(q2-q3).*cos(q4).*sin(q5).*8.191520442889917e-1).^2+(sin(q6).*(cos(q2-q3).*sin(q5).*8.191520442889917e-1+sin(q2-q3).*cos(q4).*cos(q5)-sin(q2-q3).*sin(q4).*sin(q5).*5.735764363510462e-1)-cos(q6).*(cos(q2-q3).*4.698463103929542e-1+sin(q2-q3).*sin(q4).*6.710100716628342e-1+cos(q5).*(cos(q2-q3).*8.191520442889917e-1-sin(q2-q3).*sin(q4).*5.735764363510462e-1).*5.735764363510462e-1-sin(q2-q3).*cos(q4).*sin(q5).*5.735764363510462e-1)).^2))+imag(cos(q6).*(cos(q2-q3).*sin(q5).*8.191520442889917e-1+sin(q2-q3).*cos(q4).*cos(q5)-sin(q2-q3).*sin(q4).*sin(q5).*5.735764363510462e-1))).*(imag(dq6.*sin(q6).*(cos(q2-q3).*sin(q5).*8.191520442889917e-1+sin(q2-q3).*cos(q4).*cos(q5)-sin(q2-q3).*sin(q4).*sin(q5).*5.735764363510462e-1))+imag(cos(q6).*(dq5.*cos(q2-q3).*cos(q5).*(-8.191520442889917e-1)+sin(q2-q3).*sin(q5).*(dq2-dq3).*8.191520442889917e-1+dq4.*sin(q2-q3).*cos(q4).*sin(q5).*5.735764363510462e-1+dq4.*sin(q2-q3).*cos(q5).*sin(q4)+dq5.*sin(q2-q3).*cos(q4).*sin(q5)+dq5.*sin(q2-q3).*cos(q5).*sin(q4).*5.735764363510462e-1-cos(q2-q3).*cos(q4).*cos(q5).*(dq2-dq3)+cos(q2-q3).*sin(q4).*sin(q5).*(dq2-dq3).*5.735764363510462e-1))-imag(dq6.*cos(q6).*(cos(q2-q3).*4.698463103929542e-1+sin(q2-q3).*sin(q4).*6.710100716628342e-1+cos(q5).*(cos(q2-q3).*8.191520442889917e-1-sin(q2-q3).*sin(q4).*5.735764363510462e-1).*5.735764363510462e-1-sin(q2-q3).*cos(q4).*sin(q5).*5.735764363510462e-1))+imag(sin(q6).*(cos(q5).*(sin(q2-q3).*(dq2-dq3).*8.191520442889917e-1+dq4.*sin(q2-q3).*cos(q4).*5.735764363510462e-1+cos(q2-q3).*sin(q4).*(dq2-dq3).*5.735764363510462e-1).*5.735764363510462e-1+sin(q2-q3).*(dq2-dq3).*4.698463103929542e-1-dq4.*sin(q2-q3).*cos(q4).*6.710100716628342e-1-cos(q2-q3).*sin(q4).*(dq2-dq3).*6.710100716628342e-1+dq5.*sin(q5).*(cos(q2-q3).*8.191520442889917e-1-sin(q2-q3).*sin(q4).*5.735764363510462e-1).*5.735764363510462e-1+dq5.*sin(q2-q3).*cos(q4).*cos(q5).*5.735764363510462e-1-dq4.*sin(q2-q3).*sin(q4).*sin(q5).*5.735764363510462e-1+cos(q2-q3).*cos(q4).*sin(q5).*(dq2-dq3).*5.735764363510462e-1))-real(1.0./sqrt((cos(q2-q3).*3.289899283371657e-1+sin(q2-q3).*sin(q4).*4.698463103929542e-1-cos(q5).*(cos(q2-q3).*8.191520442889917e-1-sin(q2-q3).*sin(q4).*5.735764363510462e-1).*8.191520442889917e-1+sin(q2-q3).*cos(q4).*sin(q5).*8.191520442889917e-1).^2+(sin(q6).*(cos(q2-q3).*sin(q5).*8.191520442889917e-1+sin(q2-q3).*cos(q4).*cos(q5)-sin(q2-q3).*sin(q4).*sin(q5).*5.735764363510462e-1)-cos(q6).*(cos(q2-q3).*4.698463103929542e-1+sin(q2-q3).*sin(q4).*6.710100716628342e-1+cos(q5).*(cos(q2-q3).*8.191520442889917e-1-sin(q2-q3).*sin(q4).*5.735764363510462e-1).*5.735764363510462e-1-sin(q2-q3).*cos(q4).*sin(q5).*5.735764363510462e-1)).^2).*((sin(q6).*(cos(q2-q3).*sin(q5).*8.191520442889917e-1+sin(q2-q3).*cos(q4).*cos(q5)-sin(q2-q3).*sin(q4).*sin(q5).*5.735764363510462e-1)-cos(q6).*(cos(q2-q3).*4.698463103929542e-1+sin(q2-q3).*sin(q4).*6.710100716628342e-1+cos(q5).*(cos(q2-q3).*8.191520442889917e-1-sin(q2-q3).*sin(q4).*5.735764363510462e-1).*5.735764363510462e-1-sin(q2-q3).*cos(q4).*sin(q5).*5.735764363510462e-1)).*(cos(q6).*(cos(q5).*(sin(q2-q3).*(dq2-dq3).*8.191520442889917e-1+dq4.*sin(q2-q3).*cos(q4).*5.735764363510462e-1+cos(q2-q3).*sin(q4).*(dq2-dq3).*5.735764363510462e-1).*5.735764363510462e-1+sin(q2-q3).*(dq2-dq3).*4.698463103929542e-1-dq4.*sin(q2-q3).*cos(q4).*6.710100716628342e-1-cos(q2-q3).*sin(q4).*(dq2-dq3).*6.710100716628342e-1+dq5.*sin(q5).*(cos(q2-q3).*8.191520442889917e-1-sin(q2-q3).*sin(q4).*5.735764363510462e-1).*5.735764363510462e-1+dq5.*sin(q2-q3).*cos(q4).*cos(q5).*5.735764363510462e-1-dq4.*sin(q2-q3).*sin(q4).*sin(q5).*5.735764363510462e-1+cos(q2-q3).*cos(q4).*sin(q5).*(dq2-dq3).*5.735764363510462e-1)-sin(q6).*(dq5.*cos(q2-q3).*cos(q5).*(-8.191520442889917e-1)+sin(q2-q3).*sin(q5).*(dq2-dq3).*8.191520442889917e-1+dq4.*sin(q2-q3).*cos(q4).*sin(q5).*5.735764363510462e-1+dq4.*sin(q2-q3).*cos(q5).*sin(q4)+dq5.*sin(q2-q3).*cos(q4).*sin(q5)+dq5.*sin(q2-q3).*cos(q5).*sin(q4).*5.735764363510462e-1-cos(q2-q3).*cos(q4).*cos(q5).*(dq2-dq3)+cos(q2-q3).*sin(q4).*sin(q5).*(dq2-dq3).*5.735764363510462e-1)+dq6.*sin(q6).*(cos(q2-q3).*4.698463103929542e-1+sin(q2-q3).*sin(q4).*6.710100716628342e-1+cos(q5).*(cos(q2-q3).*8.191520442889917e-1-sin(q2-q3).*sin(q4).*5.735764363510462e-1).*5.735764363510462e-1-sin(q2-q3).*cos(q4).*sin(q5).*5.735764363510462e-1)+dq6.*cos(q6).*(cos(q2-q3).*sin(q5).*8.191520442889917e-1+sin(q2-q3).*cos(q4).*cos(q5)-sin(q2-q3).*sin(q4).*sin(q5).*5.735764363510462e-1)).*2.0+(cos(q2-q3).*3.289899283371657e-1+sin(q2-q3).*sin(q4).*4.698463103929542e-1-cos(q5).*(cos(q2-q3).*8.191520442889917e-1-sin(q2-q3).*sin(q4).*5.735764363510462e-1).*8.191520442889917e-1+sin(q2-q3).*cos(q4).*sin(q5).*8.191520442889917e-1).*(cos(q5).*(sin(q2-q3).*(dq2-dq3).*8.191520442889917e-1+dq4.*sin(q2-q3).*cos(q4).*5.735764363510462e-1+cos(q2-q3).*sin(q4).*(dq2-dq3).*5.735764363510462e-1).*8.191520442889917e-1-sin(q2-q3).*(dq2-dq3).*3.289899283371657e-1+dq4.*sin(q2-q3).*cos(q4).*4.698463103929542e-1+cos(q2-q3).*sin(q4).*(dq2-dq3).*4.698463103929542e-1+dq5.*sin(q5).*(cos(q2-q3).*8.191520442889917e-1-sin(q2-q3).*sin(q4).*5.735764363510462e-1).*8.191520442889917e-1+dq5.*sin(q2-q3).*cos(q4).*cos(q5).*8.191520442889917e-1-dq4.*sin(q2-q3).*sin(q4).*sin(q5).*8.191520442889917e-1+cos(q2-q3).*cos(q4).*sin(q5).*(dq2-dq3).*8.191520442889917e-1).*2.0)).*(1.0./2.0)).*2.0).*1.0./((real(sin(q6).*(cos(q2-q3).*4.698463103929542e-1+sin(q2-q3).*sin(q4).*6.710100716628342e-1+cos(q5).*(cos(q2-q3).*8.191520442889917e-1-sin(q2-q3).*sin(q4).*5.735764363510462e-1).*5.735764363510462e-1-sin(q2-q3).*cos(q4).*sin(q5).*5.735764363510462e-1))-imag(sqrt((cos(q2-q3).*3.289899283371657e-1+sin(q2-q3).*sin(q4).*4.698463103929542e-1-cos(q5).*(cos(q2-q3).*8.191520442889917e-1-sin(q2-q3).*sin(q4).*5.735764363510462e-1).*8.191520442889917e-1+sin(q2-q3).*cos(q4).*sin(q5).*8.191520442889917e-1).^2+(sin(q6).*(cos(q2-q3).*sin(q5).*8.191520442889917e-1+sin(q2-q3).*cos(q4).*cos(q5)-sin(q2-q3).*sin(q4).*sin(q5).*5.735764363510462e-1)-cos(q6).*(cos(q2-q3).*4.698463103929542e-1+sin(q2-q3).*sin(q4).*6.710100716628342e-1+cos(q5).*(cos(q2-q3).*8.191520442889917e-1-sin(q2-q3).*sin(q4).*5.735764363510462e-1).*5.735764363510462e-1-sin(q2-q3).*cos(q4).*sin(q5).*5.735764363510462e-1)).^2))+real(cos(q6).*(cos(q2-q3).*sin(q5).*8.191520442889917e-1+sin(q2-q3).*cos(q4).*cos(q5)-sin(q2-q3).*sin(q4).*sin(q5).*5.735764363510462e-1))).^2+(imag(sin(q6).*(cos(q2-q3).*4.698463103929542e-1+sin(q2-q3).*sin(q4).*6.710100716628342e-1+cos(q5).*(cos(q2-q3).*8.191520442889917e-1-sin(q2-q3).*sin(q4).*5.735764363510462e-1).*5.735764363510462e-1-sin(q2-q3).*cos(q4).*sin(q5).*5.735764363510462e-1))+real(sqrt((cos(q2-q3).*3.289899283371657e-1+sin(q2-q3).*sin(q4).*4.698463103929542e-1-cos(q5).*(cos(q2-q3).*8.191520442889917e-1-sin(q2-q3).*sin(q4).*5.735764363510462e-1).*8.191520442889917e-1+sin(q2-q3).*cos(q4).*sin(q5).*8.191520442889917e-1).^2+(sin(q6).*(cos(q2-q3).*sin(q5).*8.191520442889917e-1+sin(q2-q3).*cos(q4).*cos(q5)-sin(q2-q3).*sin(q4).*sin(q5).*5.735764363510462e-1)-cos(q6).*(cos(q2-q3).*4.698463103929542e-1+sin(q2-q3).*sin(q4).*6.710100716628342e-1+cos(q5).*(cos(q2-q3).*8.191520442889917e-1-sin(q2-q3).*sin(q4).*5.735764363510462e-1).*5.735764363510462e-1-sin(q2-q3).*cos(q4).*sin(q5).*5.735764363510462e-1)).^2))+imag(cos(q6).*(cos(q2-q3).*sin(q5).*8.191520442889917e-1+sin(q2-q3).*cos(q4).*cos(q5)-sin(q2-q3).*sin(q4).*sin(q5).*5.735764363510462e-1))).^2).^2.*((real(sin(q6).*(sin(q5).*(cos(q2-q3).*8.191520442889917e-1-sin(q2-q3).*sin(q4).*5.735764363510462e-1).*5.735764363510462e-1+sin(q2-q3).*cos(q4).*cos(q5).*5.735764363510462e-1))+imag(1.0./sqrt((cos(q2-q3).*3.289899283371657e-1+sin(q2-q3).*sin(q4).*4.698463103929542e-1-cos(q5).*(cos(q2-q3).*8.191520442889917e-1-sin(q2-q3).*sin(q4).*5.735764363510462e-1).*8.191520442889917e-1+sin(q2-q3).*cos(q4).*sin(q5).*8.191520442889917e-1).^2+(sin(q6).*(cos(q2-q3).*sin(q5).*8.191520442889917e-1+sin(q2-q3).*cos(q4).*cos(q5)-sin(q2-q3).*sin(q4).*sin(q5).*5.735764363510462e-1)-cos(q6).*(cos(q2-q3).*4.698463103929542e-1+sin(q2-q3).*sin(q4).*6.710100716628342e-1+cos(q5).*(cos(q2-q3).*8.191520442889917e-1-sin(q2-q3).*sin(q4).*5.735764363510462e-1).*5.735764363510462e-1-sin(q2-q3).*cos(q4).*sin(q5).*5.735764363510462e-1)).^2).*((sin(q6).*(cos(q2-q3).*sin(q5).*8.191520442889917e-1+sin(q2-q3).*cos(q4).*cos(q5)-sin(q2-q3).*sin(q4).*sin(q5).*5.735764363510462e-1)-cos(q6).*(cos(q2-q3).*4.698463103929542e-1+sin(q2-q3).*sin(q4).*6.710100716628342e-1+cos(q5).*(cos(q2-q3).*8.191520442889917e-1-sin(q2-q3).*sin(q4).*5.735764363510462e-1).*5.735764363510462e-1-sin(q2-q3).*cos(q4).*sin(q5).*5.735764363510462e-1)).*(cos(q6).*(sin(q5).*(cos(q2-q3).*8.191520442889917e-1-sin(q2-q3).*sin(q4).*5.735764363510462e-1).*5.735764363510462e-1+sin(q2-q3).*cos(q4).*cos(q5).*5.735764363510462e-1)-sin(q6).*(cos(q2-q3).*cos(q5).*(-8.191520442889917e-1)+sin(q2-q3).*cos(q4).*sin(q5)+sin(q2-q3).*cos(q5).*sin(q4).*5.735764363510462e-1)).*2.0+(sin(q5).*(cos(q2-q3).*8.191520442889917e-1-sin(q2-q3).*sin(q4).*5.735764363510462e-1).*8.191520442889917e-1+sin(q2-q3).*cos(q4).*cos(q5).*8.191520442889917e-1).*(cos(q2-q3).*3.289899283371657e-1+sin(q2-q3).*sin(q4).*4.698463103929542e-1-cos(q5).*(cos(q2-q3).*8.191520442889917e-1-sin(q2-q3).*sin(q4).*5.735764363510462e-1).*8.191520442889917e-1+sin(q2-q3).*cos(q4).*sin(q5).*8.191520442889917e-1).*2.0)).*(1.0./2.0)+real(cos(q6).*(cos(q2-q3).*cos(q5).*(-8.191520442889917e-1)+sin(q2-q3).*cos(q4).*sin(q5)+sin(q2-q3).*cos(q5).*sin(q4).*5.735764363510462e-1)))./(imag(sin(q6).*(cos(q2-q3).*4.698463103929542e-1+sin(q2-q3).*sin(q4).*6.710100716628342e-1+cos(q5).*(cos(q2-q3).*8.191520442889917e-1-sin(q2-q3).*sin(q4).*5.735764363510462e-1).*5.735764363510462e-1-sin(q2-q3).*cos(q4).*sin(q5).*5.735764363510462e-1))+real(sqrt((cos(q2-q3).*3.289899283371657e-1+sin(q2-q3).*sin(q4).*4.698463103929542e-1-cos(q5).*(cos(q2-q3).*8.191520442889917e-1-sin(q2-q3).*sin(q4).*5.735764363510462e-1).*8.191520442889917e-1+sin(q2-q3).*cos(q4).*sin(q5).*8.191520442889917e-1).^2+(sin(q6).*(cos(q2-q3).*sin(q5).*8.191520442889917e-1+sin(q2-q3).*cos(q4).*cos(q5)-sin(q2-q3).*sin(q4).*sin(q5).*5.735764363510462e-1)-cos(q6).*(cos(q2-q3).*4.698463103929542e-1+sin(q2-q3).*sin(q4).*6.710100716628342e-1+cos(q5).*(cos(q2-q3).*8.191520442889917e-1-sin(q2-q3).*sin(q4).*5.735764363510462e-1).*5.735764363510462e-1-sin(q2-q3).*cos(q4).*sin(q5).*5.735764363510462e-1)).^2))+imag(cos(q6).*(cos(q2-q3).*sin(q5).*8.191520442889917e-1+sin(q2-q3).*cos(q4).*cos(q5)-sin(q2-q3).*sin(q4).*sin(q5).*5.735764363510462e-1)))-1.0./(imag(sin(q6).*(cos(q2-q3).*4.698463103929542e-1+sin(q2-q3).*sin(q4).*6.710100716628342e-1+cos(q5).*(cos(q2-q3).*8.191520442889917e-1-sin(q2-q3).*sin(q4).*5.735764363510462e-1).*5.735764363510462e-1-sin(q2-q3).*cos(q4).*sin(q5).*5.735764363510462e-1))+real(sqrt((cos(q2-q3).*3.289899283371657e-1+sin(q2-q3).*sin(q4).*4.698463103929542e-1-cos(q5).*(cos(q2-q3).*8.191520442889917e-1-sin(q2-q3).*sin(q4).*5.735764363510462e-1).*8.191520442889917e-1+sin(q2-q3).*cos(q4).*sin(q5).*8.191520442889917e-1).^2+(sin(q6).*(cos(q2-q3).*sin(q5).*8.191520442889917e-1+sin(q2-q3).*cos(q4).*cos(q5)-sin(q2-q3).*sin(q4).*sin(q5).*5.735764363510462e-1)-cos(q6).*(cos(q2-q3).*4.698463103929542e-1+sin(q2-q3).*sin(q4).*6.710100716628342e-1+cos(q5).*(cos(q2-q3).*8.191520442889917e-1-sin(q2-q3).*sin(q4).*5.735764363510462e-1).*5.735764363510462e-1-sin(q2-q3).*cos(q4).*sin(q5).*5.735764363510462e-1)).^2))+imag(cos(q6).*(cos(q2-q3).*sin(q5).*8.191520442889917e-1+sin(q2-q3).*cos(q4).*cos(q5)-sin(q2-q3).*sin(q4).*sin(q5).*5.735764363510462e-1))).^2.*(imag(sin(q6).*(sin(q5).*(cos(q2-q3).*8.191520442889917e-1-sin(q2-q3).*sin(q4).*5.735764363510462e-1).*5.735764363510462e-1+sin(q2-q3).*cos(q4).*cos(q5).*5.735764363510462e-1))+imag(cos(q6).*(cos(q2-q3).*cos(q5).*(-8.191520442889917e-1)+sin(q2-q3).*cos(q4).*sin(q5)+sin(q2-q3).*cos(q5).*sin(q4).*5.735764363510462e-1))-real(1.0./sqrt((cos(q2-q3).*3.289899283371657e-1+sin(q2-q3).*sin(q4).*4.698463103929542e-1-cos(q5).*(cos(q2-q3).*8.191520442889917e-1-sin(q2-q3).*sin(q4).*5.735764363510462e-1).*8.191520442889917e-1+sin(q2-q3).*cos(q4).*sin(q5).*8.191520442889917e-1).^2+(sin(q6).*(cos(q2-q3).*sin(q5).*8.191520442889917e-1+sin(q2-q3).*cos(q4).*cos(q5)-sin(q2-q3).*sin(q4).*sin(q5).*5.735764363510462e-1)-cos(q6).*(cos(q2-q3).*4.698463103929542e-1+sin(q2-q3).*sin(q4).*6.710100716628342e-1+cos(q5).*(cos(q2-q3).*8.191520442889917e-1-sin(q2-q3).*sin(q4).*5.735764363510462e-1).*5.735764363510462e-1-sin(q2-q3).*cos(q4).*sin(q5).*5.735764363510462e-1)).^2).*((sin(q6).*(cos(q2-q3).*sin(q5).*8.191520442889917e-1+sin(q2-q3).*cos(q4).*cos(q5)-sin(q2-q3).*sin(q4).*sin(q5).*5.735764363510462e-1)-cos(q6).*(cos(q2-q3).*4.698463103929542e-1+sin(q2-q3).*sin(q4).*6.710100716628342e-1+cos(q5).*(cos(q2-q3).*8.191520442889917e-1-sin(q2-q3).*sin(q4).*5.735764363510462e-1).*5.735764363510462e-1-sin(q2-q3).*cos(q4).*sin(q5).*5.735764363510462e-1)).*(cos(q6).*(sin(q5).*(cos(q2-q3).*8.191520442889917e-1-sin(q2-q3).*sin(q4).*5.735764363510462e-1).*5.735764363510462e-1+sin(q2-q3).*cos(q4).*cos(q5).*5.735764363510462e-1)-sin(q6).*(cos(q2-q3).*cos(q5).*(-8.191520442889917e-1)+sin(q2-q3).*cos(q4).*sin(q5)+sin(q2-q3).*cos(q5).*sin(q4).*5.735764363510462e-1)).*2.0+(sin(q5).*(cos(q2-q3).*8.191520442889917e-1-sin(q2-q3).*sin(q4).*5.735764363510462e-1).*8.191520442889917e-1+sin(q2-q3).*cos(q4).*cos(q5).*8.191520442889917e-1).*(cos(q2-q3).*3.289899283371657e-1+sin(q2-q3).*sin(q4).*4.698463103929542e-1-cos(q5).*(cos(q2-q3).*8.191520442889917e-1-sin(q2-q3).*sin(q4).*5.735764363510462e-1).*8.191520442889917e-1+sin(q2-q3).*cos(q4).*sin(q5).*8.191520442889917e-1).*2.0)).*(1.0./2.0)).*(real(sin(q6).*(cos(q2-q3).*4.698463103929542e-1+sin(q2-q3).*sin(q4).*6.710100716628342e-1+cos(q5).*(cos(q2-q3).*8.191520442889917e-1-sin(q2-q3).*sin(q4).*5.735764363510462e-1).*5.735764363510462e-1-sin(q2-q3).*cos(q4).*sin(q5).*5.735764363510462e-1))-imag(sqrt((cos(q2-q3).*3.289899283371657e-1+sin(q2-q3).*sin(q4).*4.698463103929542e-1-cos(q5).*(cos(q2-q3).*8.191520442889917e-1-sin(q2-q3).*sin(q4).*5.735764363510462e-1).*8.191520442889917e-1+sin(q2-q3).*cos(q4).*sin(q5).*8.191520442889917e-1).^2+(sin(q6).*(cos(q2-q3).*sin(q5).*8.191520442889917e-1+sin(q2-q3).*cos(q4).*cos(q5)-sin(q2-q3).*sin(q4).*sin(q5).*5.735764363510462e-1)-cos(q6).*(cos(q2-q3).*4.698463103929542e-1+sin(q2-q3).*sin(q4).*6.710100716628342e-1+cos(q5).*(cos(q2-q3).*8.191520442889917e-1-sin(q2-q3).*sin(q4).*5.735764363510462e-1).*5.735764363510462e-1-sin(q2-q3).*cos(q4).*sin(q5).*5.735764363510462e-1)).^2))+real(cos(q6).*(cos(q2-q3).*sin(q5).*8.191520442889917e-1+sin(q2-q3).*cos(q4).*cos(q5)-sin(q2-q3).*sin(q4).*sin(q5).*5.735764363510462e-1)))).*(imag(sin(q6).*(cos(q2-q3).*4.698463103929542e-1+sin(q2-q3).*sin(q4).*6.710100716628342e-1+cos(q5).*(cos(q2-q3).*8.191520442889917e-1-sin(q2-q3).*sin(q4).*5.735764363510462e-1).*5.735764363510462e-1-sin(q2-q3).*cos(q4).*sin(q5).*5.735764363510462e-1))+real(sqrt((cos(q2-q3).*3.289899283371657e-1+sin(q2-q3).*sin(q4).*4.698463103929542e-1-cos(q5).*(cos(q2-q3).*8.191520442889917e-1-sin(q2-q3).*sin(q4).*5.735764363510462e-1).*8.191520442889917e-1+sin(q2-q3).*cos(q4).*sin(q5).*8.191520442889917e-1).^2+(sin(q6).*(cos(q2-q3).*sin(q5).*8.191520442889917e-1+sin(q2-q3).*cos(q4).*cos(q5)-sin(q2-q3).*sin(q4).*sin(q5).*5.735764363510462e-1)-cos(q6).*(cos(q2-q3).*4.698463103929542e-1+sin(q2-q3).*sin(q4).*6.710100716628342e-1+cos(q5).*(cos(q2-q3).*8.191520442889917e-1-sin(q2-q3).*sin(q4).*5.735764363510462e-1).*5.735764363510462e-1-sin(q2-q3).*cos(q4).*sin(q5).*5.735764363510462e-1)).^2))+imag(cos(q6).*(cos(q2-q3).*sin(q5).*8.191520442889917e-1+sin(q2-q3).*cos(q4).*cos(q5)-sin(q2-q3).*sin(q4).*sin(q5).*5.735764363510462e-1))).^2-(((real(sin(q6).*(sin(q5).*(cos(q2-q3).*8.191520442889917e-1-sin(q2-q3).*sin(q4).*5.735764363510462e-1).*5.735764363510462e-1+sin(q2-q3).*cos(q4).*cos(q5).*5.735764363510462e-1))+imag(1.0./sqrt((cos(q2-q3).*3.289899283371657e-1+sin(q2-q3).*sin(q4).*4.698463103929542e-1-cos(q5).*(cos(q2-q3).*8.191520442889917e-1-sin(q2-q3).*sin(q4).*5.735764363510462e-1).*8.191520442889917e-1+sin(q2-q3).*cos(q4).*sin(q5).*8.191520442889917e-1).^2+(sin(q6).*(cos(q2-q3).*sin(q5).*8.191520442889917e-1+sin(q2-q3).*cos(q4).*cos(q5)-sin(q2-q3).*sin(q4).*sin(q5).*5.735764363510462e-1)-cos(q6).*(cos(q2-q3).*4.698463103929542e-1+sin(q2-q3).*sin(q4).*6.710100716628342e-1+cos(q5).*(cos(q2-q3).*8.191520442889917e-1-sin(q2-q3).*sin(q4).*5.735764363510462e-1).*5.735764363510462e-1-sin(q2-q3).*cos(q4).*sin(q5).*5.735764363510462e-1)).^2).*((sin(q6).*(cos(q2-q3).*sin(q5).*8.191520442889917e-1+sin(q2-q3).*cos(q4).*cos(q5)-sin(q2-q3).*sin(q4).*sin(q5).*5.735764363510462e-1)-cos(q6).*(cos(q2-q3).*4.698463103929542e-1+sin(q2-q3).*sin(q4).*6.710100716628342e-1+cos(q5).*(cos(q2-q3).*8.191520442889917e-1-sin(q2-q3).*sin(q4).*5.735764363510462e-1).*5.735764363510462e-1-sin(q2-q3).*cos(q4).*sin(q5).*5.735764363510462e-1)).*(cos(q6).*(sin(q5).*(cos(q2-q3).*8.191520442889917e-1-sin(q2-q3).*sin(q4).*5.735764363510462e-1).*5.735764363510462e-1+sin(q2-q3).*cos(q4).*cos(q5).*5.735764363510462e-1)-sin(q6).*(cos(q2-q3).*cos(q5).*(-8.191520442889917e-1)+sin(q2-q3).*cos(q4).*sin(q5)+sin(q2-q3).*cos(q5).*sin(q4).*5.735764363510462e-1)).*2.0+(sin(q5).*(cos(q2-q3).*8.191520442889917e-1-sin(q2-q3).*sin(q4).*5.735764363510462e-1).*8.191520442889917e-1+sin(q2-q3).*cos(q4).*cos(q5).*8.191520442889917e-1).*(cos(q2-q3).*3.289899283371657e-1+sin(q2-q3).*sin(q4).*4.698463103929542e-1-cos(q5).*(cos(q2-q3).*8.191520442889917e-1-sin(q2-q3).*sin(q4).*5.735764363510462e-1).*8.191520442889917e-1+sin(q2-q3).*cos(q4).*sin(q5).*8.191520442889917e-1).*2.0)).*(1.0./2.0)+real(cos(q6).*(cos(q2-q3).*cos(q5).*(-8.191520442889917e-1)+sin(q2-q3).*cos(q4).*sin(q5)+sin(q2-q3).*cos(q5).*sin(q4).*5.735764363510462e-1)))./(imag(sin(q6).*(cos(q2-q3).*4.698463103929542e-1+sin(q2-q3).*sin(q4).*6.710100716628342e-1+cos(q5).*(cos(q2-q3).*8.191520442889917e-1-sin(q2-q3).*sin(q4).*5.735764363510462e-1).*5.735764363510462e-1-sin(q2-q3).*cos(q4).*sin(q5).*5.735764363510462e-1))+real(sqrt((cos(q2-q3).*3.289899283371657e-1+sin(q2-q3).*sin(q4).*4.698463103929542e-1-cos(q5).*(cos(q2-q3).*8.191520442889917e-1-sin(q2-q3).*sin(q4).*5.735764363510462e-1).*8.191520442889917e-1+sin(q2-q3).*cos(q4).*sin(q5).*8.191520442889917e-1).^2+(sin(q6).*(cos(q2-q3).*sin(q5).*8.191520442889917e-1+sin(q2-q3).*cos(q4).*cos(q5)-sin(q2-q3).*sin(q4).*sin(q5).*5.735764363510462e-1)-cos(q6).*(cos(q2-q3).*4.698463103929542e-1+sin(q2-q3).*sin(q4).*6.710100716628342e-1+cos(q5).*(cos(q2-q3).*8.191520442889917e-1-sin(q2-q3).*sin(q4).*5.735764363510462e-1).*5.735764363510462e-1-sin(q2-q3).*cos(q4).*sin(q5).*5.735764363510462e-1)).^2))+imag(cos(q6).*(cos(q2-q3).*sin(q5).*8.191520442889917e-1+sin(q2-q3).*cos(q4).*cos(q5)-sin(q2-q3).*sin(q4).*sin(q5).*5.735764363510462e-1)))-1.0./(imag(sin(q6).*(cos(q2-q3).*4.698463103929542e-1+sin(q2-q3).*sin(q4).*6.710100716628342e-1+cos(q5).*(cos(q2-q3).*8.191520442889917e-1-sin(q2-q3).*sin(q4).*5.735764363510462e-1).*5.735764363510462e-1-sin(q2-q3).*cos(q4).*sin(q5).*5.735764363510462e-1))+real(sqrt((cos(q2-q3).*3.289899283371657e-1+sin(q2-q3).*sin(q4).*4.698463103929542e-1-cos(q5).*(cos(q2-q3).*8.191520442889917e-1-sin(q2-q3).*sin(q4).*5.735764363510462e-1).*8.191520442889917e-1+sin(q2-q3).*cos(q4).*sin(q5).*8.191520442889917e-1).^2+(sin(q6).*(cos(q2-q3).*sin(q5).*8.191520442889917e-1+sin(q2-q3).*cos(q4).*cos(q5)-sin(q2-q3).*sin(q4).*sin(q5).*5.735764363510462e-1)-cos(q6).*(cos(q2-q3).*4.698463103929542e-1+sin(q2-q3).*sin(q4).*6.710100716628342e-1+cos(q5).*(cos(q2-q3).*8.191520442889917e-1-sin(q2-q3).*sin(q4).*5.735764363510462e-1).*5.735764363510462e-1-sin(q2-q3).*cos(q4).*sin(q5).*5.735764363510462e-1)).^2))+imag(cos(q6).*(cos(q2-q3).*sin(q5).*8.191520442889917e-1+sin(q2-q3).*cos(q4).*cos(q5)-sin(q2-q3).*sin(q4).*sin(q5).*5.735764363510462e-1))).^2.*(imag(sin(q6).*(sin(q5).*(cos(q2-q3).*8.191520442889917e-1-sin(q2-q3).*sin(q4).*5.735764363510462e-1).*5.735764363510462e-1+sin(q2-q3).*cos(q4).*cos(q5).*5.735764363510462e-1))+imag(cos(q6).*(cos(q2-q3).*cos(q5).*(-8.191520442889917e-1)+sin(q2-q3).*cos(q4).*sin(q5)+sin(q2-q3).*cos(q5).*sin(q4).*5.735764363510462e-1))-real(1.0./sqrt((cos(q2-q3).*3.289899283371657e-1+sin(q2-q3).*sin(q4).*4.698463103929542e-1-cos(q5).*(cos(q2-q3).*8.191520442889917e-1-sin(q2-q3).*sin(q4).*5.735764363510462e-1).*8.191520442889917e-1+sin(q2-q3).*cos(q4).*sin(q5).*8.191520442889917e-1).^2+(sin(q6).*(cos(q2-q3).*sin(q5).*8.191520442889917e-1+sin(q2-q3).*cos(q4).*cos(q5)-sin(q2-q3).*sin(q4).*sin(q5).*5.735764363510462e-1)-cos(q6).*(cos(q2-q3).*4.698463103929542e-1+sin(q2-q3).*sin(q4).*6.710100716628342e-1+cos(q5).*(cos(q2-q3).*8.191520442889917e-1-sin(q2-q3).*sin(q4).*5.735764363510462e-1).*5.735764363510462e-1-sin(q2-q3).*cos(q4).*sin(q5).*5.735764363510462e-1)).^2).*((sin(q6).*(cos(q2-q3).*sin(q5).*8.191520442889917e-1+sin(q2-q3).*cos(q4).*cos(q5)-sin(q2-q3).*sin(q4).*sin(q5).*5.735764363510462e-1)-cos(q6).*(cos(q2-q3).*4.698463103929542e-1+sin(q2-q3).*sin(q4).*6.710100716628342e-1+cos(q5).*(cos(q2-q3).*8.191520442889917e-1-sin(q2-q3).*sin(q4).*5.735764363510462e-1).*5.735764363510462e-1-sin(q2-q3).*cos(q4).*sin(q5).*5.735764363510462e-1)).*(cos(q6).*(sin(q5).*(cos(q2-q3).*8.191520442889917e-1-sin(q2-q3).*sin(q4).*5.735764363510462e-1).*5.735764363510462e-1+sin(q2-q3).*cos(q4).*cos(q5).*5.735764363510462e-1)-sin(q6).*(cos(q2-q3).*cos(q5).*(-8.191520442889917e-1)+sin(q2-q3).*cos(q4).*sin(q5)+sin(q2-q3).*cos(q5).*sin(q4).*5.735764363510462e-1)).*2.0+(sin(q5).*(cos(q2-q3).*8.191520442889917e-1-sin(q2-q3).*sin(q4).*5.735764363510462e-1).*8.191520442889917e-1+sin(q2-q3).*cos(q4).*cos(q5).*8.191520442889917e-1).*(cos(q2-q3).*3.289899283371657e-1+sin(q2-q3).*sin(q4).*4.698463103929542e-1-cos(q5).*(cos(q2-q3).*8.191520442889917e-1-sin(q2-q3).*sin(q4).*5.735764363510462e-1).*8.191520442889917e-1+sin(q2-q3).*cos(q4).*sin(q5).*8.191520442889917e-1).*2.0)).*(1.0./2.0)).*(real(sin(q6).*(cos(q2-q3).*4.698463103929542e-1+sin(q2-q3).*sin(q4).*6.710100716628342e-1+cos(q5).*(cos(q2-q3).*8.191520442889917e-1-sin(q2-q3).*sin(q4).*5.735764363510462e-1).*5.735764363510462e-1-sin(q2-q3).*cos(q4).*sin(q5).*5.735764363510462e-1))-imag(sqrt((cos(q2-q3).*3.289899283371657e-1+sin(q2-q3).*sin(q4).*4.698463103929542e-1-cos(q5).*(cos(q2-q3).*8.191520442889917e-1-sin(q2-q3).*sin(q4).*5.735764363510462e-1).*8.191520442889917e-1+sin(q2-q3).*cos(q4).*sin(q5).*8.191520442889917e-1).^2+(sin(q6).*(cos(q2-q3).*sin(q5).*8.191520442889917e-1+sin(q2-q3).*cos(q4).*cos(q5)-sin(q2-q3).*sin(q4).*sin(q5).*5.735764363510462e-1)-cos(q6).*(cos(q2-q3).*4.698463103929542e-1+sin(q2-q3).*sin(q4).*6.710100716628342e-1+cos(q5).*(cos(q2-q3).*8.191520442889917e-1-sin(q2-q3).*sin(q4).*5.735764363510462e-1).*5.735764363510462e-1-sin(q2-q3).*cos(q4).*sin(q5).*5.735764363510462e-1)).^2))+real(cos(q6).*(cos(q2-q3).*sin(q5).*8.191520442889917e-1+sin(q2-q3).*cos(q4).*cos(q5)-sin(q2-q3).*sin(q4).*sin(q5).*5.735764363510462e-1)))).*(imag(sin(q6).*(cos(q2-q3).*4.698463103929542e-1+sin(q2-q3).*sin(q4).*6.710100716628342e-1+cos(q5).*(cos(q2-q3).*8.191520442889917e-1-sin(q2-q3).*sin(q4).*5.735764363510462e-1).*5.735764363510462e-1-sin(q2-q3).*cos(q4).*sin(q5).*5.735764363510462e-1))+real(sqrt((cos(q2-q3).*3.289899283371657e-1+sin(q2-q3).*sin(q4).*4.698463103929542e-1-cos(q5).*(cos(q2-q3).*8.191520442889917e-1-sin(q2-q3).*sin(q4).*5.735764363510462e-1).*8.191520442889917e-1+sin(q2-q3).*cos(q4).*sin(q5).*8.191520442889917e-1).^2+(sin(q6).*(cos(q2-q3).*sin(q5).*8.191520442889917e-1+sin(q2-q3).*cos(q4).*cos(q5)-sin(q2-q3).*sin(q4).*sin(q5).*5.735764363510462e-1)-cos(q6).*(cos(q2-q3).*4.698463103929542e-1+sin(q2-q3).*sin(q4).*6.710100716628342e-1+cos(q5).*(cos(q2-q3).*8.191520442889917e-1-sin(q2-q3).*sin(q4).*5.735764363510462e-1).*5.735764363510462e-1-sin(q2-q3).*cos(q4).*sin(q5).*5.735764363510462e-1)).^2))+imag(cos(q6).*(cos(q2-q3).*sin(q5).*8.191520442889917e-1+sin(q2-q3).*cos(q4).*cos(q5)-sin(q2-q3).*sin(q4).*sin(q5).*5.735764363510462e-1))).*(imag(dq6.*sin(q6).*(cos(q2-q3).*sin(q5).*8.191520442889917e-1+sin(q2-q3).*cos(q4).*cos(q5)-sin(q2-q3).*sin(q4).*sin(q5).*5.735764363510462e-1))+imag(cos(q6).*(dq5.*cos(q2-q3).*cos(q5).*(-8.191520442889917e-1)+sin(q2-q3).*sin(q5).*(dq2-dq3).*8.191520442889917e-1+dq4.*sin(q2-q3).*cos(q4).*sin(q5).*5.735764363510462e-1+dq4.*sin(q2-q3).*cos(q5).*sin(q4)+dq5.*sin(q2-q3).*cos(q4).*sin(q5)+dq5.*sin(q2-q3).*cos(q5).*sin(q4).*5.735764363510462e-1-cos(q2-q3).*cos(q4).*cos(q5).*(dq2-dq3)+cos(q2-q3).*sin(q4).*sin(q5).*(dq2-dq3).*5.735764363510462e-1))-imag(dq6.*cos(q6).*(cos(q2-q3).*4.698463103929542e-1+sin(q2-q3).*sin(q4).*6.710100716628342e-1+cos(q5).*(cos(q2-q3).*8.191520442889917e-1-sin(q2-q3).*sin(q4).*5.735764363510462e-1).*5.735764363510462e-1-sin(q2-q3).*cos(q4).*sin(q5).*5.735764363510462e-1))+imag(sin(q6).*(cos(q5).*(sin(q2-q3).*(dq2-dq3).*8.191520442889917e-1+dq4.*sin(q2-q3).*cos(q4).*5.735764363510462e-1+cos(q2-q3).*sin(q4).*(dq2-dq3).*5.735764363510462e-1).*5.735764363510462e-1+sin(q2-q3).*(dq2-dq3).*4.698463103929542e-1-dq4.*sin(q2-q3).*cos(q4).*6.710100716628342e-1-cos(q2-q3).*sin(q4).*(dq2-dq3).*6.710100716628342e-1+dq5.*sin(q5).*(cos(q2-q3).*8.191520442889917e-1-sin(q2-q3).*sin(q4).*5.735764363510462e-1).*5.735764363510462e-1+dq5.*sin(q2-q3).*cos(q4).*cos(q5).*5.735764363510462e-1-dq4.*sin(q2-q3).*sin(q4).*sin(q5).*5.735764363510462e-1+cos(q2-q3).*cos(q4).*sin(q5).*(dq2-dq3).*5.735764363510462e-1))-real(1.0./sqrt((cos(q2-q3).*3.289899283371657e-1+sin(q2-q3).*sin(q4).*4.698463103929542e-1-cos(q5).*(cos(q2-q3).*8.191520442889917e-1-sin(q2-q3).*sin(q4).*5.735764363510462e-1).*8.191520442889917e-1+sin(q2-q3).*cos(q4).*sin(q5).*8.191520442889917e-1).^2+(sin(q6).*(cos(q2-q3).*sin(q5).*8.191520442889917e-1+sin(q2-q3).*cos(q4).*cos(q5)-sin(q2-q3).*sin(q4).*sin(q5).*5.735764363510462e-1)-cos(q6).*(cos(q2-q3).*4.698463103929542e-1+sin(q2-q3).*sin(q4).*6.710100716628342e-1+cos(q5).*(cos(q2-q3).*8.191520442889917e-1-sin(q2-q3).*sin(q4).*5.735764363510462e-1).*5.735764363510462e-1-sin(q2-q3).*cos(q4).*sin(q5).*5.735764363510462e-1)).^2).*((sin(q6).*(cos(q2-q3).*sin(q5).*8.191520442889917e-1+sin(q2-q3).*cos(q4).*cos(q5)-sin(q2-q3).*sin(q4).*sin(q5).*5.735764363510462e-1)-cos(q6).*(cos(q2-q3).*4.698463103929542e-1+sin(q2-q3).*sin(q4).*6.710100716628342e-1+cos(q5).*(cos(q2-q3).*8.191520442889917e-1-sin(q2-q3).*sin(q4).*5.735764363510462e-1).*5.735764363510462e-1-sin(q2-q3).*cos(q4).*sin(q5).*5.735764363510462e-1)).*(cos(q6).*(cos(q5).*(sin(q2-q3).*(dq2-dq3).*8.191520442889917e-1+dq4.*sin(q2-q3).*cos(q4).*5.735764363510462e-1+cos(q2-q3).*sin(q4).*(dq2-dq3).*5.735764363510462e-1).*5.735764363510462e-1+sin(q2-q3).*(dq2-dq3).*4.698463103929542e-1-dq4.*sin(q2-q3).*cos(q4).*6.710100716628342e-1-cos(q2-q3).*sin(q4).*(dq2-dq3).*6.710100716628342e-1+dq5.*sin(q5).*(cos(q2-q3).*8.191520442889917e-1-sin(q2-q3).*sin(q4).*5.735764363510462e-1).*5.735764363510462e-1+dq5.*sin(q2-q3).*cos(q4).*cos(q5).*5.735764363510462e-1-dq4.*sin(q2-q3).*sin(q4).*sin(q5).*5.735764363510462e-1+cos(q2-q3).*cos(q4).*sin(q5).*(dq2-dq3).*5.735764363510462e-1)-sin(q6).*(dq5.*cos(q2-q3).*cos(q5).*(-8.191520442889917e-1)+sin(q2-q3).*sin(q5).*(dq2-dq3).*8.191520442889917e-1+dq4.*sin(q2-q3).*cos(q4).*sin(q5).*5.735764363510462e-1+dq4.*sin(q2-q3).*cos(q5).*sin(q4)+dq5.*sin(q2-q3).*cos(q4).*sin(q5)+dq5.*sin(q2-q3).*cos(q5).*sin(q4).*5.735764363510462e-1-cos(q2-q3).*cos(q4).*cos(q5).*(dq2-dq3)+cos(q2-q3).*sin(q4).*sin(q5).*(dq2-dq3).*5.735764363510462e-1)+dq6.*sin(q6).*(cos(q2-q3).*4.698463103929542e-1+sin(q2-q3).*sin(q4).*6.710100716628342e-1+cos(q5).*(cos(q2-q3).*8.191520442889917e-1-sin(q2-q3).*sin(q4).*5.735764363510462e-1).*5.735764363510462e-1-sin(q2-q3).*cos(q4).*sin(q5).*5.735764363510462e-1)+dq6.*cos(q6).*(cos(q2-q3).*sin(q5).*8.191520442889917e-1+sin(q2-q3).*cos(q4).*cos(q5)-sin(q2-q3).*sin(q4).*sin(q5).*5.735764363510462e-1)).*2.0+(cos(q2-q3).*3.289899283371657e-1+sin(q2-q3).*sin(q4).*4.698463103929542e-1-cos(q5).*(cos(q2-q3).*8.191520442889917e-1-sin(q2-q3).*sin(q4).*5.735764363510462e-1).*8.191520442889917e-1+sin(q2-q3).*cos(q4).*sin(q5).*8.191520442889917e-1).*(cos(q5).*(sin(q2-q3).*(dq2-dq3).*8.191520442889917e-1+dq4.*sin(q2-q3).*cos(q4).*5.735764363510462e-1+cos(q2-q3).*sin(q4).*(dq2-dq3).*5.735764363510462e-1).*8.191520442889917e-1-sin(q2-q3).*(dq2-dq3).*3.289899283371657e-1+dq4.*sin(q2-q3).*cos(q4).*4.698463103929542e-1+cos(q2-q3).*sin(q4).*(dq2-dq3).*4.698463103929542e-1+dq5.*sin(q5).*(cos(q2-q3).*8.191520442889917e-1-sin(q2-q3).*sin(q4).*5.735764363510462e-1).*8.191520442889917e-1+dq5.*sin(q2-q3).*cos(q4).*cos(q5).*8.191520442889917e-1-dq4.*sin(q2-q3).*sin(q4).*sin(q5).*8.191520442889917e-1+cos(q2-q3).*cos(q4).*sin(q5).*(dq2-dq3).*8.191520442889917e-1).*2.0)).*(1.0./2.0)).*2.0)./((real(sin(q6).*(cos(q2-q3).*4.698463103929542e-1+sin(q2-q3).*sin(q4).*6.710100716628342e-1+cos(q5).*(cos(q2-q3).*8.191520442889917e-1-sin(q2-q3).*sin(q4).*5.735764363510462e-1).*5.735764363510462e-1-sin(q2-q3).*cos(q4).*sin(q5).*5.735764363510462e-1))-imag(sqrt((cos(q2-q3).*3.289899283371657e-1+sin(q2-q3).*sin(q4).*4.698463103929542e-1-cos(q5).*(cos(q2-q3).*8.191520442889917e-1-sin(q2-q3).*sin(q4).*5.735764363510462e-1).*8.191520442889917e-1+sin(q2-q3).*cos(q4).*sin(q5).*8.191520442889917e-1).^2+(sin(q6).*(cos(q2-q3).*sin(q5).*8.191520442889917e-1+sin(q2-q3).*cos(q4).*cos(q5)-sin(q2-q3).*sin(q4).*sin(q5).*5.735764363510462e-1)-cos(q6).*(cos(q2-q3).*4.698463103929542e-1+sin(q2-q3).*sin(q4).*6.710100716628342e-1+cos(q5).*(cos(q2-q3).*8.191520442889917e-1-sin(q2-q3).*sin(q4).*5.735764363510462e-1).*5.735764363510462e-1-sin(q2-q3).*cos(q4).*sin(q5).*5.735764363510462e-1)).^2))+real(cos(q6).*(cos(q2-q3).*sin(q5).*8.191520442889917e-1+sin(q2-q3).*cos(q4).*cos(q5)-sin(q2-q3).*sin(q4).*sin(q5).*5.735764363510462e-1))).^2+(imag(sin(q6).*(cos(q2-q3).*4.698463103929542e-1+sin(q2-q3).*sin(q4).*6.710100716628342e-1+cos(q5).*(cos(q2-q3).*8.191520442889917e-1-sin(q2-q3).*sin(q4).*5.735764363510462e-1).*5.735764363510462e-1-sin(q2-q3).*cos(q4).*sin(q5).*5.735764363510462e-1))+real(sqrt((cos(q2-q3).*3.289899283371657e-1+sin(q2-q3).*sin(q4).*4.698463103929542e-1-cos(q5).*(cos(q2-q3).*8.191520442889917e-1-sin(q2-q3).*sin(q4).*5.735764363510462e-1).*8.191520442889917e-1+sin(q2-q3).*cos(q4).*sin(q5).*8.191520442889917e-1).^2+(sin(q6).*(cos(q2-q3).*sin(q5).*8.191520442889917e-1+sin(q2-q3).*cos(q4).*cos(q5)-sin(q2-q3).*sin(q4).*sin(q5).*5.735764363510462e-1)-cos(q6).*(cos(q2-q3).*4.698463103929542e-1+sin(q2-q3).*sin(q4).*6.710100716628342e-1+cos(q5).*(cos(q2-q3).*8.191520442889917e-1-sin(q2-q3).*sin(q4).*5.735764363510462e-1).*5.735764363510462e-1-sin(q2-q3).*cos(q4).*sin(q5).*5.735764363510462e-1)).^2))+imag(cos(q6).*(cos(q2-q3).*sin(q5).*8.191520442889917e-1+sin(q2-q3).*cos(q4).*cos(q5)-sin(q2-q3).*sin(q4).*sin(q5).*5.735764363510462e-1))).^2),(((real(dq6.*cos(q6).*(cos(q2-q3).*cos(q5).*(-8.191520442889917e-1)+sin(q2-q3).*cos(q4).*sin(q5)+sin(q2-q3).*cos(q5).*sin(q4).*5.735764363510462e-1))+imag(dq5.*cos(q5).*(cos(q2-q3).*8.191520442889917e-1-sin(q2-q3).*sin(q4).*5.735764363510462e-1)).*8.191520442889917e-1+real(sin(q6).*(dq5.*cos(q2-q3).*sin(q5).*8.191520442889917e-1+sin(q2-q3).*cos(q5).*(dq2-dq3).*8.191520442889917e-1+dq4.*sin(q2-q3).*cos(q4).*cos(q5).*5.735764363510462e-1+dq5.*sin(q2-q3).*cos(q4).*cos(q5)-dq4.*sin(q2-q3).*sin(q4).*sin(q5)-dq5.*sin(q2-q3).*sin(q4).*sin(q5).*5.735764363510462e-1+cos(q2-q3).*cos(q4).*sin(q5).*(dq2-dq3)+cos(q2-q3).*cos(q5).*sin(q4).*(dq2-dq3).*5.735764363510462e-1))-imag(sin(q5).*(sin(q2-q3).*(dq2-dq3).*8.191520442889917e-1+dq4.*sin(q2-q3).*cos(q4).*5.735764363510462e-1+cos(q2-q3).*sin(q4).*(dq2-dq3).*5.735764363510462e-1)).*8.191520442889917e-1+real(cos(q6).*(sin(q5).*(sin(q2-q3).*(dq2-dq3).*8.191520442889917e-1+dq4.*sin(q2-q3).*cos(q4).*5.735764363510462e-1+cos(q2-q3).*sin(q4).*(dq2-dq3).*5.735764363510462e-1).*5.735764363510462e-1-dq5.*cos(q5).*(cos(q2-q3).*8.191520442889917e-1-sin(q2-q3).*sin(q4).*5.735764363510462e-1).*5.735764363510462e-1+dq4.*sin(q2-q3).*cos(q5).*sin(q4).*5.735764363510462e-1+dq5.*sin(q2-q3).*cos(q4).*sin(q5).*5.735764363510462e-1-cos(q2-q3).*cos(q4).*cos(q5).*(dq2-dq3).*5.735764363510462e-1))-imag(dq4.*sin(q2-q3).*cos(q5).*sin(q4)).*8.191520442889917e-1-imag(dq5.*sin(q2-q3).*cos(q4).*sin(q5)).*8.191520442889917e-1+imag(cos(q2-q3).*cos(q4).*cos(q5).*(dq2-dq3)).*8.191520442889917e-1+real(dq6.*sin(q6).*(sin(q5).*(cos(q2-q3).*8.191520442889917e-1-sin(q2-q3).*sin(q4).*5.735764363510462e-1).*5.735764363510462e-1+sin(q2-q3).*cos(q4).*cos(q5).*5.735764363510462e-1)))./(real(cos(q2-q3)).*3.289899283371657e-1+real(sin(q2-q3).*cos(q4).*sin(q5)).*8.191520442889917e-1+real(sin(q2-q3).*sin(q4)).*4.698463103929542e-1+imag(sin(q6).*(cos(q2-q3).*sin(q5).*8.191520442889917e-1+sin(q2-q3).*cos(q4).*cos(q5)-sin(q2-q3).*sin(q4).*sin(q5).*5.735764363510462e-1))-real(cos(q5).*(cos(q2-q3).*8.191520442889917e-1-sin(q2-q3).*sin(q4).*5.735764363510462e-1)).*8.191520442889917e-1-imag(cos(q6).*(cos(q2-q3).*4.698463103929542e-1+sin(q2-q3).*sin(q4).*6.710100716628342e-1+cos(q5).*(cos(q2-q3).*8.191520442889917e-1-sin(q2-q3).*sin(q4).*5.735764363510462e-1).*5.735764363510462e-1-sin(q2-q3).*cos(q4).*sin(q5).*5.735764363510462e-1)))-(imag(sin(q2-q3).*cos(q4).*cos(q5)).*8.191520442889917e-1-real(cos(q6).*(sin(q5).*(cos(q2-q3).*8.191520442889917e-1-sin(q2-q3).*sin(q4).*5.735764363510462e-1).*5.735764363510462e-1+sin(q2-q3).*cos(q4).*cos(q5).*5.735764363510462e-1))+real(sin(q6).*(cos(q2-q3).*cos(q5).*(-8.191520442889917e-1)+sin(q2-q3).*cos(q4).*sin(q5)+sin(q2-q3).*cos(q5).*sin(q4).*5.735764363510462e-1))+imag(sin(q5).*(cos(q2-q3).*8.191520442889917e-1-sin(q2-q3).*sin(q4).*5.735764363510462e-1)).*8.191520442889917e-1).*1.0./(real(cos(q2-q3)).*3.289899283371657e-1+real(sin(q2-q3).*cos(q4).*sin(q5)).*8.191520442889917e-1+real(sin(q2-q3).*sin(q4)).*4.698463103929542e-1+imag(sin(q6).*(cos(q2-q3).*sin(q5).*8.191520442889917e-1+sin(q2-q3).*cos(q4).*cos(q5)-sin(q2-q3).*sin(q4).*sin(q5).*5.735764363510462e-1))-real(cos(q5).*(cos(q2-q3).*8.191520442889917e-1-sin(q2-q3).*sin(q4).*5.735764363510462e-1)).*8.191520442889917e-1-imag(cos(q6).*(cos(q2-q3).*4.698463103929542e-1+sin(q2-q3).*sin(q4).*6.710100716628342e-1+cos(q5).*(cos(q2-q3).*8.191520442889917e-1-sin(q2-q3).*sin(q4).*5.735764363510462e-1).*5.735764363510462e-1-sin(q2-q3).*cos(q4).*sin(q5).*5.735764363510462e-1))).^2.*(imag(dq6.*cos(q6).*(cos(q2-q3).*sin(q5).*8.191520442889917e-1+sin(q2-q3).*cos(q4).*cos(q5)-sin(q2-q3).*sin(q4).*sin(q5).*5.735764363510462e-1))+real(cos(q2-q3).*sin(q4).*(dq2-dq3)).*4.698463103929542e-1-imag(sin(q6).*(dq5.*cos(q2-q3).*cos(q5).*(-8.191520442889917e-1)+sin(q2-q3).*sin(q5).*(dq2-dq3).*8.191520442889917e-1+dq4.*sin(q2-q3).*cos(q4).*sin(q5).*5.735764363510462e-1+dq4.*sin(q2-q3).*cos(q5).*sin(q4)+dq5.*sin(q2-q3).*cos(q4).*sin(q5)+dq5.*sin(q2-q3).*cos(q5).*sin(q4).*5.735764363510462e-1-cos(q2-q3).*cos(q4).*cos(q5).*(dq2-dq3)+cos(q2-q3).*sin(q4).*sin(q5).*(dq2-dq3).*5.735764363510462e-1))+real(dq5.*sin(q5).*(cos(q2-q3).*8.191520442889917e-1-sin(q2-q3).*sin(q4).*5.735764363510462e-1)).*8.191520442889917e-1-real(sin(q2-q3).*(dq2-dq3)).*3.289899283371657e-1+imag(cos(q6).*(cos(q5).*(sin(q2-q3).*(dq2-dq3).*8.191520442889917e-1+dq4.*sin(q2-q3).*cos(q4).*5.735764363510462e-1+cos(q2-q3).*sin(q4).*(dq2-dq3).*5.735764363510462e-1).*5.735764363510462e-1+sin(q2-q3).*(dq2-dq3).*4.698463103929542e-1-dq4.*sin(q2-q3).*cos(q4).*6.710100716628342e-1-cos(q2-q3).*sin(q4).*(dq2-dq3).*6.710100716628342e-1+dq5.*sin(q5).*(cos(q2-q3).*8.191520442889917e-1-sin(q2-q3).*sin(q4).*5.735764363510462e-1).*5.735764363510462e-1+dq5.*sin(q2-q3).*cos(q4).*cos(q5).*5.735764363510462e-1-dq4.*sin(q2-q3).*sin(q4).*sin(q5).*5.735764363510462e-1+cos(q2-q3).*cos(q4).*sin(q5).*(dq2-dq3).*5.735764363510462e-1))+imag(dq6.*sin(q6).*(cos(q2-q3).*4.698463103929542e-1+sin(q2-q3).*sin(q4).*6.710100716628342e-1+cos(q5).*(cos(q2-q3).*8.191520442889917e-1-sin(q2-q3).*sin(q4).*5.735764363510462e-1).*5.735764363510462e-1-sin(q2-q3).*cos(q4).*sin(q5).*5.735764363510462e-1))+real(cos(q5).*(sin(q2-q3).*(dq2-dq3).*8.191520442889917e-1+dq4.*sin(q2-q3).*cos(q4).*5.735764363510462e-1+cos(q2-q3).*sin(q4).*(dq2-dq3).*5.735764363510462e-1)).*8.191520442889917e-1+real(dq5.*sin(q2-q3).*cos(q4).*cos(q5)).*8.191520442889917e-1-real(dq4.*sin(q2-q3).*sin(q4).*sin(q5)).*8.191520442889917e-1+real(cos(q2-q3).*cos(q4).*sin(q5).*(dq2-dq3)).*8.191520442889917e-1+real(dq4.*sin(q2-q3).*cos(q4)).*4.698463103929542e-1)+(real(cos(q6).*(cos(q2-q3).*4.698463103929542e-1+sin(q2-q3).*sin(q4).*6.710100716628342e-1+cos(q5).*(cos(q2-q3).*8.191520442889917e-1-sin(q2-q3).*sin(q4).*5.735764363510462e-1).*5.735764363510462e-1-sin(q2-q3).*cos(q4).*sin(q5).*5.735764363510462e-1))+imag(cos(q2-q3)).*3.289899283371657e-1+imag(sin(q2-q3).*cos(q4).*sin(q5)).*8.191520442889917e-1+imag(sin(q2-q3).*sin(q4)).*4.698463103929542e-1-real(sin(q6).*(cos(q2-q3).*sin(q5).*8.191520442889917e-1+sin(q2-q3).*cos(q4).*cos(q5)-sin(q2-q3).*sin(q4).*sin(q5).*5.735764363510462e-1))-imag(cos(q5).*(cos(q2-q3).*8.191520442889917e-1-sin(q2-q3).*sin(q4).*5.735764363510462e-1)).*8.191520442889917e-1).*1.0./(real(cos(q2-q3)).*3.289899283371657e-1+real(sin(q2-q3).*cos(q4).*sin(q5)).*8.191520442889917e-1+real(sin(q2-q3).*sin(q4)).*4.698463103929542e-1+imag(sin(q6).*(cos(q2-q3).*sin(q5).*8.191520442889917e-1+sin(q2-q3).*cos(q4).*cos(q5)-sin(q2-q3).*sin(q4).*sin(q5).*5.735764363510462e-1))-real(cos(q5).*(cos(q2-q3).*8.191520442889917e-1-sin(q2-q3).*sin(q4).*5.735764363510462e-1)).*8.191520442889917e-1-imag(cos(q6).*(cos(q2-q3).*4.698463103929542e-1+sin(q2-q3).*sin(q4).*6.710100716628342e-1+cos(q5).*(cos(q2-q3).*8.191520442889917e-1-sin(q2-q3).*sin(q4).*5.735764363510462e-1).*5.735764363510462e-1-sin(q2-q3).*cos(q4).*sin(q5).*5.735764363510462e-1))).^2.*(real(dq5.*cos(q5).*(cos(q2-q3).*8.191520442889917e-1-sin(q2-q3).*sin(q4).*5.735764363510462e-1)).*(-8.191520442889917e-1)+imag(sin(q6).*(dq5.*cos(q2-q3).*sin(q5).*8.191520442889917e-1+sin(q2-q3).*cos(q5).*(dq2-dq3).*8.191520442889917e-1+dq4.*sin(q2-q3).*cos(q4).*cos(q5).*5.735764363510462e-1+dq5.*sin(q2-q3).*cos(q4).*cos(q5)-dq4.*sin(q2-q3).*sin(q4).*sin(q5)-dq5.*sin(q2-q3).*sin(q4).*sin(q5).*5.735764363510462e-1+cos(q2-q3).*cos(q4).*sin(q5).*(dq2-dq3)+cos(q2-q3).*cos(q5).*sin(q4).*(dq2-dq3).*5.735764363510462e-1))+imag(cos(q6).*(sin(q5).*(sin(q2-q3).*(dq2-dq3).*8.191520442889917e-1+dq4.*sin(q2-q3).*cos(q4).*5.735764363510462e-1+cos(q2-q3).*sin(q4).*(dq2-dq3).*5.735764363510462e-1).*5.735764363510462e-1-dq5.*cos(q5).*(cos(q2-q3).*8.191520442889917e-1-sin(q2-q3).*sin(q4).*5.735764363510462e-1).*5.735764363510462e-1+dq4.*sin(q2-q3).*cos(q5).*sin(q4).*5.735764363510462e-1+dq5.*sin(q2-q3).*cos(q4).*sin(q5).*5.735764363510462e-1-cos(q2-q3).*cos(q4).*cos(q5).*(dq2-dq3).*5.735764363510462e-1))+real(sin(q5).*(sin(q2-q3).*(dq2-dq3).*8.191520442889917e-1+dq4.*sin(q2-q3).*cos(q4).*5.735764363510462e-1+cos(q2-q3).*sin(q4).*(dq2-dq3).*5.735764363510462e-1)).*8.191520442889917e-1+imag(dq6.*sin(q6).*(sin(q5).*(cos(q2-q3).*8.191520442889917e-1-sin(q2-q3).*sin(q4).*5.735764363510462e-1).*5.735764363510462e-1+sin(q2-q3).*cos(q4).*cos(q5).*5.735764363510462e-1))+real(dq4.*sin(q2-q3).*cos(q5).*sin(q4)).*8.191520442889917e-1+real(dq5.*sin(q2-q3).*cos(q4).*sin(q5)).*8.191520442889917e-1-real(cos(q2-q3).*cos(q4).*cos(q5).*(dq2-dq3)).*8.191520442889917e-1+imag(dq6.*cos(q6).*(cos(q2-q3).*cos(q5).*(-8.191520442889917e-1)+sin(q2-q3).*cos(q4).*sin(q5)+sin(q2-q3).*cos(q5).*sin(q4).*5.735764363510462e-1)))-(imag(cos(q6).*(sin(q5).*(cos(q2-q3).*8.191520442889917e-1-sin(q2-q3).*sin(q4).*5.735764363510462e-1).*5.735764363510462e-1+sin(q2-q3).*cos(q4).*cos(q5).*5.735764363510462e-1))+real(sin(q2-q3).*cos(q4).*cos(q5)).*8.191520442889917e-1-imag(sin(q6).*(cos(q2-q3).*cos(q5).*(-8.191520442889917e-1)+sin(q2-q3).*cos(q4).*sin(q5)+sin(q2-q3).*cos(q5).*sin(q4).*5.735764363510462e-1))+real(sin(q5).*(cos(q2-q3).*8.191520442889917e-1-sin(q2-q3).*sin(q4).*5.735764363510462e-1)).*8.191520442889917e-1).*1.0./(real(cos(q2-q3)).*3.289899283371657e-1+real(sin(q2-q3).*cos(q4).*sin(q5)).*8.191520442889917e-1+real(sin(q2-q3).*sin(q4)).*4.698463103929542e-1+imag(sin(q6).*(cos(q2-q3).*sin(q5).*8.191520442889917e-1+sin(q2-q3).*cos(q4).*cos(q5)-sin(q2-q3).*sin(q4).*sin(q5).*5.735764363510462e-1))-real(cos(q5).*(cos(q2-q3).*8.191520442889917e-1-sin(q2-q3).*sin(q4).*5.735764363510462e-1)).*8.191520442889917e-1-imag(cos(q6).*(cos(q2-q3).*4.698463103929542e-1+sin(q2-q3).*sin(q4).*6.710100716628342e-1+cos(q5).*(cos(q2-q3).*8.191520442889917e-1-sin(q2-q3).*sin(q4).*5.735764363510462e-1).*5.735764363510462e-1-sin(q2-q3).*cos(q4).*sin(q5).*5.735764363510462e-1))).^2.*(-real(dq6.*cos(q6).*(cos(q2-q3).*sin(q5).*8.191520442889917e-1+sin(q2-q3).*cos(q4).*cos(q5)-sin(q2-q3).*sin(q4).*sin(q5).*5.735764363510462e-1))+imag(cos(q2-q3).*sin(q4).*(dq2-dq3)).*4.698463103929542e-1+imag(dq5.*sin(q5).*(cos(q2-q3).*8.191520442889917e-1-sin(q2-q3).*sin(q4).*5.735764363510462e-1)).*8.191520442889917e-1+real(sin(q6).*(dq5.*cos(q2-q3).*cos(q5).*(-8.191520442889917e-1)+sin(q2-q3).*sin(q5).*(dq2-dq3).*8.191520442889917e-1+dq4.*sin(q2-q3).*cos(q4).*sin(q5).*5.735764363510462e-1+dq4.*sin(q2-q3).*cos(q5).*sin(q4)+dq5.*sin(q2-q3).*cos(q4).*sin(q5)+dq5.*sin(q2-q3).*cos(q5).*sin(q4).*5.735764363510462e-1-cos(q2-q3).*cos(q4).*cos(q5).*(dq2-dq3)+cos(q2-q3).*sin(q4).*sin(q5).*(dq2-dq3).*5.735764363510462e-1))-imag(sin(q2-q3).*(dq2-dq3)).*3.289899283371657e-1-real(cos(q6).*(cos(q5).*(sin(q2-q3).*(dq2-dq3).*8.191520442889917e-1+dq4.*sin(q2-q3).*cos(q4).*5.735764363510462e-1+cos(q2-q3).*sin(q4).*(dq2-dq3).*5.735764363510462e-1).*5.735764363510462e-1+sin(q2-q3).*(dq2-dq3).*4.698463103929542e-1-dq4.*sin(q2-q3).*cos(q4).*6.710100716628342e-1-cos(q2-q3).*sin(q4).*(dq2-dq3).*6.710100716628342e-1+dq5.*sin(q5).*(cos(q2-q3).*8.191520442889917e-1-sin(q2-q3).*sin(q4).*5.735764363510462e-1).*5.735764363510462e-1+dq5.*sin(q2-q3).*cos(q4).*cos(q5).*5.735764363510462e-1-dq4.*sin(q2-q3).*sin(q4).*sin(q5).*5.735764363510462e-1+cos(q2-q3).*cos(q4).*sin(q5).*(dq2-dq3).*5.735764363510462e-1))+imag(cos(q5).*(sin(q2-q3).*(dq2-dq3).*8.191520442889917e-1+dq4.*sin(q2-q3).*cos(q4).*5.735764363510462e-1+cos(q2-q3).*sin(q4).*(dq2-dq3).*5.735764363510462e-1)).*8.191520442889917e-1-real(dq6.*sin(q6).*(cos(q2-q3).*4.698463103929542e-1+sin(q2-q3).*sin(q4).*6.710100716628342e-1+cos(q5).*(cos(q2-q3).*8.191520442889917e-1-sin(q2-q3).*sin(q4).*5.735764363510462e-1).*5.735764363510462e-1-sin(q2-q3).*cos(q4).*sin(q5).*5.735764363510462e-1))+imag(dq5.*sin(q2-q3).*cos(q4).*cos(q5)).*8.191520442889917e-1-imag(dq4.*sin(q2-q3).*sin(q4).*sin(q5)).*8.191520442889917e-1+imag(cos(q2-q3).*cos(q4).*sin(q5).*(dq2-dq3)).*8.191520442889917e-1+imag(dq4.*sin(q2-q3).*cos(q4)).*4.698463103929542e-1)+(imag(cos(q6).*(sin(q5).*(cos(q2-q3).*8.191520442889917e-1-sin(q2-q3).*sin(q4).*5.735764363510462e-1).*5.735764363510462e-1+sin(q2-q3).*cos(q4).*cos(q5).*5.735764363510462e-1))+real(sin(q2-q3).*cos(q4).*cos(q5)).*8.191520442889917e-1-imag(sin(q6).*(cos(q2-q3).*cos(q5).*(-8.191520442889917e-1)+sin(q2-q3).*cos(q4).*sin(q5)+sin(q2-q3).*cos(q5).*sin(q4).*5.735764363510462e-1))+real(sin(q5).*(cos(q2-q3).*8.191520442889917e-1-sin(q2-q3).*sin(q4).*5.735764363510462e-1)).*8.191520442889917e-1).*(real(cos(q6).*(cos(q2-q3).*4.698463103929542e-1+sin(q2-q3).*sin(q4).*6.710100716628342e-1+cos(q5).*(cos(q2-q3).*8.191520442889917e-1-sin(q2-q3).*sin(q4).*5.735764363510462e-1).*5.735764363510462e-1-sin(q2-q3).*cos(q4).*sin(q5).*5.735764363510462e-1))+imag(cos(q2-q3)).*3.289899283371657e-1+imag(sin(q2-q3).*cos(q4).*sin(q5)).*8.191520442889917e-1+imag(sin(q2-q3).*sin(q4)).*4.698463103929542e-1-real(sin(q6).*(cos(q2-q3).*sin(q5).*8.191520442889917e-1+sin(q2-q3).*cos(q4).*cos(q5)-sin(q2-q3).*sin(q4).*sin(q5).*5.735764363510462e-1))-imag(cos(q5).*(cos(q2-q3).*8.191520442889917e-1-sin(q2-q3).*sin(q4).*5.735764363510462e-1)).*8.191520442889917e-1).*1.0./(real(cos(q2-q3)).*3.289899283371657e-1+real(sin(q2-q3).*cos(q4).*sin(q5)).*8.191520442889917e-1+real(sin(q2-q3).*sin(q4)).*4.698463103929542e-1+imag(sin(q6).*(cos(q2-q3).*sin(q5).*8.191520442889917e-1+sin(q2-q3).*cos(q4).*cos(q5)-sin(q2-q3).*sin(q4).*sin(q5).*5.735764363510462e-1))-real(cos(q5).*(cos(q2-q3).*8.191520442889917e-1-sin(q2-q3).*sin(q4).*5.735764363510462e-1)).*8.191520442889917e-1-imag(cos(q6).*(cos(q2-q3).*4.698463103929542e-1+sin(q2-q3).*sin(q4).*6.710100716628342e-1+cos(q5).*(cos(q2-q3).*8.191520442889917e-1-sin(q2-q3).*sin(q4).*5.735764363510462e-1).*5.735764363510462e-1-sin(q2-q3).*cos(q4).*sin(q5).*5.735764363510462e-1))).^3.*(imag(dq6.*cos(q6).*(cos(q2-q3).*sin(q5).*8.191520442889917e-1+sin(q2-q3).*cos(q4).*cos(q5)-sin(q2-q3).*sin(q4).*sin(q5).*5.735764363510462e-1))+real(cos(q2-q3).*sin(q4).*(dq2-dq3)).*4.698463103929542e-1-imag(sin(q6).*(dq5.*cos(q2-q3).*cos(q5).*(-8.191520442889917e-1)+sin(q2-q3).*sin(q5).*(dq2-dq3).*8.191520442889917e-1+dq4.*sin(q2-q3).*cos(q4).*sin(q5).*5.735764363510462e-1+dq4.*sin(q2-q3).*cos(q5).*sin(q4)+dq5.*sin(q2-q3).*cos(q4).*sin(q5)+dq5.*sin(q2-q3).*cos(q5).*sin(q4).*5.735764363510462e-1-cos(q2-q3).*cos(q4).*cos(q5).*(dq2-dq3)+cos(q2-q3).*sin(q4).*sin(q5).*(dq2-dq3).*5.735764363510462e-1))+real(dq5.*sin(q5).*(cos(q2-q3).*8.191520442889917e-1-sin(q2-q3).*sin(q4).*5.735764363510462e-1)).*8.191520442889917e-1-real(sin(q2-q3).*(dq2-dq3)).*3.289899283371657e-1+imag(cos(q6).*(cos(q5).*(sin(q2-q3).*(dq2-dq3).*8.191520442889917e-1+dq4.*sin(q2-q3).*cos(q4).*5.735764363510462e-1+cos(q2-q3).*sin(q4).*(dq2-dq3).*5.735764363510462e-1).*5.735764363510462e-1+sin(q2-q3).*(dq2-dq3).*4.698463103929542e-1-dq4.*sin(q2-q3).*cos(q4).*6.710100716628342e-1-cos(q2-q3).*sin(q4).*(dq2-dq3).*6.710100716628342e-1+dq5.*sin(q5).*(cos(q2-q3).*8.191520442889917e-1-sin(q2-q3).*sin(q4).*5.735764363510462e-1).*5.735764363510462e-1+dq5.*sin(q2-q3).*cos(q4).*cos(q5).*5.735764363510462e-1-dq4.*sin(q2-q3).*sin(q4).*sin(q5).*5.735764363510462e-1+cos(q2-q3).*cos(q4).*sin(q5).*(dq2-dq3).*5.735764363510462e-1))+imag(dq6.*sin(q6).*(cos(q2-q3).*4.698463103929542e-1+sin(q2-q3).*sin(q4).*6.710100716628342e-1+cos(q5).*(cos(q2-q3).*8.191520442889917e-1-sin(q2-q3).*sin(q4).*5.735764363510462e-1).*5.735764363510462e-1-sin(q2-q3).*cos(q4).*sin(q5).*5.735764363510462e-1))+real(cos(q5).*(sin(q2-q3).*(dq2-dq3).*8.191520442889917e-1+dq4.*sin(q2-q3).*cos(q4).*5.735764363510462e-1+cos(q2-q3).*sin(q4).*(dq2-dq3).*5.735764363510462e-1)).*8.191520442889917e-1+real(dq5.*sin(q2-q3).*cos(q4).*cos(q5)).*8.191520442889917e-1-real(dq4.*sin(q2-q3).*sin(q4).*sin(q5)).*8.191520442889917e-1+real(cos(q2-q3).*cos(q4).*sin(q5).*(dq2-dq3)).*8.191520442889917e-1+real(dq4.*sin(q2-q3).*cos(q4)).*4.698463103929542e-1).*2.0).*(real(cos(q2-q3)).*3.289899283371657e-1+real(sin(q2-q3).*cos(q4).*sin(q5)).*8.191520442889917e-1+real(sin(q2-q3).*sin(q4)).*4.698463103929542e-1+imag(sin(q6).*(cos(q2-q3).*sin(q5).*8.191520442889917e-1+sin(q2-q3).*cos(q4).*cos(q5)-sin(q2-q3).*sin(q4).*sin(q5).*5.735764363510462e-1))-real(cos(q5).*(cos(q2-q3).*8.191520442889917e-1-sin(q2-q3).*sin(q4).*5.735764363510462e-1)).*8.191520442889917e-1-imag(cos(q6).*(cos(q2-q3).*4.698463103929542e-1+sin(q2-q3).*sin(q4).*6.710100716628342e-1+cos(q5).*(cos(q2-q3).*8.191520442889917e-1-sin(q2-q3).*sin(q4).*5.735764363510462e-1).*5.735764363510462e-1-sin(q2-q3).*cos(q4).*sin(q5).*5.735764363510462e-1))).^2)./((real(cos(q6).*(cos(q2-q3).*4.698463103929542e-1+sin(q2-q3).*sin(q4).*6.710100716628342e-1+cos(q5).*(cos(q2-q3).*8.191520442889917e-1-sin(q2-q3).*sin(q4).*5.735764363510462e-1).*5.735764363510462e-1-sin(q2-q3).*cos(q4).*sin(q5).*5.735764363510462e-1))+imag(cos(q2-q3)).*3.289899283371657e-1+imag(sin(q2-q3).*cos(q4).*sin(q5)).*8.191520442889917e-1+imag(sin(q2-q3).*sin(q4)).*4.698463103929542e-1-real(sin(q6).*(cos(q2-q3).*sin(q5).*8.191520442889917e-1+sin(q2-q3).*cos(q4).*cos(q5)-sin(q2-q3).*sin(q4).*sin(q5).*5.735764363510462e-1))-imag(cos(q5).*(cos(q2-q3).*8.191520442889917e-1-sin(q2-q3).*sin(q4).*5.735764363510462e-1)).*8.191520442889917e-1).^2+(real(cos(q2-q3)).*3.289899283371657e-1+real(sin(q2-q3).*cos(q4).*sin(q5)).*8.191520442889917e-1+real(sin(q2-q3).*sin(q4)).*4.698463103929542e-1+imag(sin(q6).*(cos(q2-q3).*sin(q5).*8.191520442889917e-1+sin(q2-q3).*cos(q4).*cos(q5)-sin(q2-q3).*sin(q4).*sin(q5).*5.735764363510462e-1))-real(cos(q5).*(cos(q2-q3).*8.191520442889917e-1-sin(q2-q3).*sin(q4).*5.735764363510462e-1)).*8.191520442889917e-1-imag(cos(q6).*(cos(q2-q3).*4.698463103929542e-1+sin(q2-q3).*sin(q4).*6.710100716628342e-1+cos(q5).*(cos(q2-q3).*8.191520442889917e-1-sin(q2-q3).*sin(q4).*5.735764363510462e-1).*5.735764363510462e-1-sin(q2-q3).*cos(q4).*sin(q5).*5.735764363510462e-1))).^2)+(((imag(sin(q2-q3).*cos(q4).*cos(q5)).*8.191520442889917e-1-real(cos(q6).*(sin(q5).*(cos(q2-q3).*8.191520442889917e-1-sin(q2-q3).*sin(q4).*5.735764363510462e-1).*5.735764363510462e-1+sin(q2-q3).*cos(q4).*cos(q5).*5.735764363510462e-1))+real(sin(q6).*(cos(q2-q3).*cos(q5).*(-8.191520442889917e-1)+sin(q2-q3).*cos(q4).*sin(q5)+sin(q2-q3).*cos(q5).*sin(q4).*5.735764363510462e-1))+imag(sin(q5).*(cos(q2-q3).*8.191520442889917e-1-sin(q2-q3).*sin(q4).*5.735764363510462e-1)).*8.191520442889917e-1)./(real(cos(q2-q3)).*3.289899283371657e-1+real(sin(q2-q3).*cos(q4).*sin(q5)).*8.191520442889917e-1+real(sin(q2-q3).*sin(q4)).*4.698463103929542e-1+imag(sin(q6).*(cos(q2-q3).*sin(q5).*8.191520442889917e-1+sin(q2-q3).*cos(q4).*cos(q5)-sin(q2-q3).*sin(q4).*sin(q5).*5.735764363510462e-1))-real(cos(q5).*(cos(q2-q3).*8.191520442889917e-1-sin(q2-q3).*sin(q4).*5.735764363510462e-1)).*8.191520442889917e-1-imag(cos(q6).*(cos(q2-q3).*4.698463103929542e-1+sin(q2-q3).*sin(q4).*6.710100716628342e-1+cos(q5).*(cos(q2-q3).*8.191520442889917e-1-sin(q2-q3).*sin(q4).*5.735764363510462e-1).*5.735764363510462e-1-sin(q2-q3).*cos(q4).*sin(q5).*5.735764363510462e-1)))-(imag(cos(q6).*(sin(q5).*(cos(q2-q3).*8.191520442889917e-1-sin(q2-q3).*sin(q4).*5.735764363510462e-1).*5.735764363510462e-1+sin(q2-q3).*cos(q4).*cos(q5).*5.735764363510462e-1))+real(sin(q2-q3).*cos(q4).*cos(q5)).*8.191520442889917e-1-imag(sin(q6).*(cos(q2-q3).*cos(q5).*(-8.191520442889917e-1)+sin(q2-q3).*cos(q4).*sin(q5)+sin(q2-q3).*cos(q5).*sin(q4).*5.735764363510462e-1))+real(sin(q5).*(cos(q2-q3).*8.191520442889917e-1-sin(q2-q3).*sin(q4).*5.735764363510462e-1)).*8.191520442889917e-1).*(real(cos(q6).*(cos(q2-q3).*4.698463103929542e-1+sin(q2-q3).*sin(q4).*6.710100716628342e-1+cos(q5).*(cos(q2-q3).*8.191520442889917e-1-sin(q2-q3).*sin(q4).*5.735764363510462e-1).*5.735764363510462e-1-sin(q2-q3).*cos(q4).*sin(q5).*5.735764363510462e-1))+imag(cos(q2-q3)).*3.289899283371657e-1+imag(sin(q2-q3).*cos(q4).*sin(q5)).*8.191520442889917e-1+imag(sin(q2-q3).*sin(q4)).*4.698463103929542e-1-real(sin(q6).*(cos(q2-q3).*sin(q5).*8.191520442889917e-1+sin(q2-q3).*cos(q4).*cos(q5)-sin(q2-q3).*sin(q4).*sin(q5).*5.735764363510462e-1))-imag(cos(q5).*(cos(q2-q3).*8.191520442889917e-1-sin(q2-q3).*sin(q4).*5.735764363510462e-1)).*8.191520442889917e-1).*1.0./(real(cos(q2-q3)).*3.289899283371657e-1+real(sin(q2-q3).*cos(q4).*sin(q5)).*8.191520442889917e-1+real(sin(q2-q3).*sin(q4)).*4.698463103929542e-1+imag(sin(q6).*(cos(q2-q3).*sin(q5).*8.191520442889917e-1+sin(q2-q3).*cos(q4).*cos(q5)-sin(q2-q3).*sin(q4).*sin(q5).*5.735764363510462e-1))-real(cos(q5).*(cos(q2-q3).*8.191520442889917e-1-sin(q2-q3).*sin(q4).*5.735764363510462e-1)).*8.191520442889917e-1-imag(cos(q6).*(cos(q2-q3).*4.698463103929542e-1+sin(q2-q3).*sin(q4).*6.710100716628342e-1+cos(q5).*(cos(q2-q3).*8.191520442889917e-1-sin(q2-q3).*sin(q4).*5.735764363510462e-1).*5.735764363510462e-1-sin(q2-q3).*cos(q4).*sin(q5).*5.735764363510462e-1))).^2).*(real(cos(q2-q3)).*3.289899283371657e-1+real(sin(q2-q3).*cos(q4).*sin(q5)).*8.191520442889917e-1+real(sin(q2-q3).*sin(q4)).*4.698463103929542e-1+imag(sin(q6).*(cos(q2-q3).*sin(q5).*8.191520442889917e-1+sin(q2-q3).*cos(q4).*cos(q5)-sin(q2-q3).*sin(q4).*sin(q5).*5.735764363510462e-1))-real(cos(q5).*(cos(q2-q3).*8.191520442889917e-1-sin(q2-q3).*sin(q4).*5.735764363510462e-1)).*8.191520442889917e-1-imag(cos(q6).*(cos(q2-q3).*4.698463103929542e-1+sin(q2-q3).*sin(q4).*6.710100716628342e-1+cos(q5).*(cos(q2-q3).*8.191520442889917e-1-sin(q2-q3).*sin(q4).*5.735764363510462e-1).*5.735764363510462e-1-sin(q2-q3).*cos(q4).*sin(q5).*5.735764363510462e-1))).*(imag(dq6.*cos(q6).*(cos(q2-q3).*sin(q5).*8.191520442889917e-1+sin(q2-q3).*cos(q4).*cos(q5)-sin(q2-q3).*sin(q4).*sin(q5).*5.735764363510462e-1))+real(cos(q2-q3).*sin(q4).*(dq2-dq3)).*4.698463103929542e-1-imag(sin(q6).*(dq5.*cos(q2-q3).*cos(q5).*(-8.191520442889917e-1)+sin(q2-q3).*sin(q5).*(dq2-dq3).*8.191520442889917e-1+dq4.*sin(q2-q3).*cos(q4).*sin(q5).*5.735764363510462e-1+dq4.*sin(q2-q3).*cos(q5).*sin(q4)+dq5.*sin(q2-q3).*cos(q4).*sin(q5)+dq5.*sin(q2-q3).*cos(q5).*sin(q4).*5.735764363510462e-1-cos(q2-q3).*cos(q4).*cos(q5).*(dq2-dq3)+cos(q2-q3).*sin(q4).*sin(q5).*(dq2-dq3).*5.735764363510462e-1))+real(dq5.*sin(q5).*(cos(q2-q3).*8.191520442889917e-1-sin(q2-q3).*sin(q4).*5.735764363510462e-1)).*8.191520442889917e-1-real(sin(q2-q3).*(dq2-dq3)).*3.289899283371657e-1+imag(cos(q6).*(cos(q5).*(sin(q2-q3).*(dq2-dq3).*8.191520442889917e-1+dq4.*sin(q2-q3).*cos(q4).*5.735764363510462e-1+cos(q2-q3).*sin(q4).*(dq2-dq3).*5.735764363510462e-1).*5.735764363510462e-1+sin(q2-q3).*(dq2-dq3).*4.698463103929542e-1-dq4.*sin(q2-q3).*cos(q4).*6.710100716628342e-1-cos(q2-q3).*sin(q4).*(dq2-dq3).*6.710100716628342e-1+dq5.*sin(q5).*(cos(q2-q3).*8.191520442889917e-1-sin(q2-q3).*sin(q4).*5.735764363510462e-1).*5.735764363510462e-1+dq5.*sin(q2-q3).*cos(q4).*cos(q5).*5.735764363510462e-1-dq4.*sin(q2-q3).*sin(q4).*sin(q5).*5.735764363510462e-1+cos(q2-q3).*cos(q4).*sin(q5).*(dq2-dq3).*5.735764363510462e-1))+imag(dq6.*sin(q6).*(cos(q2-q3).*4.698463103929542e-1+sin(q2-q3).*sin(q4).*6.710100716628342e-1+cos(q5).*(cos(q2-q3).*8.191520442889917e-1-sin(q2-q3).*sin(q4).*5.735764363510462e-1).*5.735764363510462e-1-sin(q2-q3).*cos(q4).*sin(q5).*5.735764363510462e-1))+real(cos(q5).*(sin(q2-q3).*(dq2-dq3).*8.191520442889917e-1+dq4.*sin(q2-q3).*cos(q4).*5.735764363510462e-1+cos(q2-q3).*sin(q4).*(dq2-dq3).*5.735764363510462e-1)).*8.191520442889917e-1+real(dq5.*sin(q2-q3).*cos(q4).*cos(q5)).*8.191520442889917e-1-real(dq4.*sin(q2-q3).*sin(q4).*sin(q5)).*8.191520442889917e-1+real(cos(q2-q3).*cos(q4).*sin(q5).*(dq2-dq3)).*8.191520442889917e-1+real(dq4.*sin(q2-q3).*cos(q4)).*4.698463103929542e-1).*2.0)./((real(cos(q6).*(cos(q2-q3).*4.698463103929542e-1+sin(q2-q3).*sin(q4).*6.710100716628342e-1+cos(q5).*(cos(q2-q3).*8.191520442889917e-1-sin(q2-q3).*sin(q4).*5.735764363510462e-1).*5.735764363510462e-1-sin(q2-q3).*cos(q4).*sin(q5).*5.735764363510462e-1))+imag(cos(q2-q3)).*3.289899283371657e-1+imag(sin(q2-q3).*cos(q4).*sin(q5)).*8.191520442889917e-1+imag(sin(q2-q3).*sin(q4)).*4.698463103929542e-1-real(sin(q6).*(cos(q2-q3).*sin(q5).*8.191520442889917e-1+sin(q2-q3).*cos(q4).*cos(q5)-sin(q2-q3).*sin(q4).*sin(q5).*5.735764363510462e-1))-imag(cos(q5).*(cos(q2-q3).*8.191520442889917e-1-sin(q2-q3).*sin(q4).*5.735764363510462e-1)).*8.191520442889917e-1).^2+(real(cos(q2-q3)).*3.289899283371657e-1+real(sin(q2-q3).*cos(q4).*sin(q5)).*8.191520442889917e-1+real(sin(q2-q3).*sin(q4)).*4.698463103929542e-1+imag(sin(q6).*(cos(q2-q3).*sin(q5).*8.191520442889917e-1+sin(q2-q3).*cos(q4).*cos(q5)-sin(q2-q3).*sin(q4).*sin(q5).*5.735764363510462e-1))-real(cos(q5).*(cos(q2-q3).*8.191520442889917e-1-sin(q2-q3).*sin(q4).*5.735764363510462e-1)).*8.191520442889917e-1-imag(cos(q6).*(cos(q2-q3).*4.698463103929542e-1+sin(q2-q3).*sin(q4).*6.710100716628342e-1+cos(q5).*(cos(q2-q3).*8.191520442889917e-1-sin(q2-q3).*sin(q4).*5.735764363510462e-1).*5.735764363510462e-1-sin(q2-q3).*cos(q4).*sin(q5).*5.735764363510462e-1))).^2)-1.0./((real(cos(q6).*(cos(q2-q3).*4.698463103929542e-1+sin(q2-q3).*sin(q4).*6.710100716628342e-1+cos(q5).*(cos(q2-q3).*8.191520442889917e-1-sin(q2-q3).*sin(q4).*5.735764363510462e-1).*5.735764363510462e-1-sin(q2-q3).*cos(q4).*sin(q5).*5.735764363510462e-1))+imag(cos(q2-q3)).*3.289899283371657e-1+imag(sin(q2-q3).*cos(q4).*sin(q5)).*8.191520442889917e-1+imag(sin(q2-q3).*sin(q4)).*4.698463103929542e-1-real(sin(q6).*(cos(q2-q3).*sin(q5).*8.191520442889917e-1+sin(q2-q3).*cos(q4).*cos(q5)-sin(q2-q3).*sin(q4).*sin(q5).*5.735764363510462e-1))-imag(cos(q5).*(cos(q2-q3).*8.191520442889917e-1-sin(q2-q3).*sin(q4).*5.735764363510462e-1)).*8.191520442889917e-1).^2+(real(cos(q2-q3)).*3.289899283371657e-1+real(sin(q2-q3).*cos(q4).*sin(q5)).*8.191520442889917e-1+real(sin(q2-q3).*sin(q4)).*4.698463103929542e-1+imag(sin(q6).*(cos(q2-q3).*sin(q5).*8.191520442889917e-1+sin(q2-q3).*cos(q4).*cos(q5)-sin(q2-q3).*sin(q4).*sin(q5).*5.735764363510462e-1))-real(cos(q5).*(cos(q2-q3).*8.191520442889917e-1-sin(q2-q3).*sin(q4).*5.735764363510462e-1)).*8.191520442889917e-1-imag(cos(q6).*(cos(q2-q3).*4.698463103929542e-1+sin(q2-q3).*sin(q4).*6.710100716628342e-1+cos(q5).*(cos(q2-q3).*8.191520442889917e-1-sin(q2-q3).*sin(q4).*5.735764363510462e-1).*5.735764363510462e-1-sin(q2-q3).*cos(q4).*sin(q5).*5.735764363510462e-1))).^2).^2.*((real(cos(q6).*(cos(q2-q3).*4.698463103929542e-1+sin(q2-q3).*sin(q4).*6.710100716628342e-1+cos(q5).*(cos(q2-q3).*8.191520442889917e-1-sin(q2-q3).*sin(q4).*5.735764363510462e-1).*5.735764363510462e-1-sin(q2-q3).*cos(q4).*sin(q5).*5.735764363510462e-1))+imag(cos(q2-q3)).*3.289899283371657e-1+imag(sin(q2-q3).*cos(q4).*sin(q5)).*8.191520442889917e-1+imag(sin(q2-q3).*sin(q4)).*4.698463103929542e-1-real(sin(q6).*(cos(q2-q3).*sin(q5).*8.191520442889917e-1+sin(q2-q3).*cos(q4).*cos(q5)-sin(q2-q3).*sin(q4).*sin(q5).*5.735764363510462e-1))-imag(cos(q5).*(cos(q2-q3).*8.191520442889917e-1-sin(q2-q3).*sin(q4).*5.735764363510462e-1)).*8.191520442889917e-1).*(-real(dq6.*cos(q6).*(cos(q2-q3).*sin(q5).*8.191520442889917e-1+sin(q2-q3).*cos(q4).*cos(q5)-sin(q2-q3).*sin(q4).*sin(q5).*5.735764363510462e-1))+imag(cos(q2-q3).*sin(q4).*(dq2-dq3)).*4.698463103929542e-1+imag(dq5.*sin(q5).*(cos(q2-q3).*8.191520442889917e-1-sin(q2-q3).*sin(q4).*5.735764363510462e-1)).*8.191520442889917e-1+real(sin(q6).*(dq5.*cos(q2-q3).*cos(q5).*(-8.191520442889917e-1)+sin(q2-q3).*sin(q5).*(dq2-dq3).*8.191520442889917e-1+dq4.*sin(q2-q3).*cos(q4).*sin(q5).*5.735764363510462e-1+dq4.*sin(q2-q3).*cos(q5).*sin(q4)+dq5.*sin(q2-q3).*cos(q4).*sin(q5)+dq5.*sin(q2-q3).*cos(q5).*sin(q4).*5.735764363510462e-1-cos(q2-q3).*cos(q4).*cos(q5).*(dq2-dq3)+cos(q2-q3).*sin(q4).*sin(q5).*(dq2-dq3).*5.735764363510462e-1))-imag(sin(q2-q3).*(dq2-dq3)).*3.289899283371657e-1-real(cos(q6).*(cos(q5).*(sin(q2-q3).*(dq2-dq3).*8.191520442889917e-1+dq4.*sin(q2-q3).*cos(q4).*5.735764363510462e-1+cos(q2-q3).*sin(q4).*(dq2-dq3).*5.735764363510462e-1).*5.735764363510462e-1+sin(q2-q3).*(dq2-dq3).*4.698463103929542e-1-dq4.*sin(q2-q3).*cos(q4).*6.710100716628342e-1-cos(q2-q3).*sin(q4).*(dq2-dq3).*6.710100716628342e-1+dq5.*sin(q5).*(cos(q2-q3).*8.191520442889917e-1-sin(q2-q3).*sin(q4).*5.735764363510462e-1).*5.735764363510462e-1+dq5.*sin(q2-q3).*cos(q4).*cos(q5).*5.735764363510462e-1-dq4.*sin(q2-q3).*sin(q4).*sin(q5).*5.735764363510462e-1+cos(q2-q3).*cos(q4).*sin(q5).*(dq2-dq3).*5.735764363510462e-1))+imag(cos(q5).*(sin(q2-q3).*(dq2-dq3).*8.191520442889917e-1+dq4.*sin(q2-q3).*cos(q4).*5.735764363510462e-1+cos(q2-q3).*sin(q4).*(dq2-dq3).*5.735764363510462e-1)).*8.191520442889917e-1-real(dq6.*sin(q6).*(cos(q2-q3).*4.698463103929542e-1+sin(q2-q3).*sin(q4).*6.710100716628342e-1+cos(q5).*(cos(q2-q3).*8.191520442889917e-1-sin(q2-q3).*sin(q4).*5.735764363510462e-1).*5.735764363510462e-1-sin(q2-q3).*cos(q4).*sin(q5).*5.735764363510462e-1))+imag(dq5.*sin(q2-q3).*cos(q4).*cos(q5)).*8.191520442889917e-1-imag(dq4.*sin(q2-q3).*sin(q4).*sin(q5)).*8.191520442889917e-1+imag(cos(q2-q3).*cos(q4).*sin(q5).*(dq2-dq3)).*8.191520442889917e-1+imag(dq4.*sin(q2-q3).*cos(q4)).*4.698463103929542e-1).*2.0+(real(cos(q2-q3)).*3.289899283371657e-1+real(sin(q2-q3).*cos(q4).*sin(q5)).*8.191520442889917e-1+real(sin(q2-q3).*sin(q4)).*4.698463103929542e-1+imag(sin(q6).*(cos(q2-q3).*sin(q5).*8.191520442889917e-1+sin(q2-q3).*cos(q4).*cos(q5)-sin(q2-q3).*sin(q4).*sin(q5).*5.735764363510462e-1))-real(cos(q5).*(cos(q2-q3).*8.191520442889917e-1-sin(q2-q3).*sin(q4).*5.735764363510462e-1)).*8.191520442889917e-1-imag(cos(q6).*(cos(q2-q3).*4.698463103929542e-1+sin(q2-q3).*sin(q4).*6.710100716628342e-1+cos(q5).*(cos(q2-q3).*8.191520442889917e-1-sin(q2-q3).*sin(q4).*5.735764363510462e-1).*5.735764363510462e-1-sin(q2-q3).*cos(q4).*sin(q5).*5.735764363510462e-1))).*(imag(dq6.*cos(q6).*(cos(q2-q3).*sin(q5).*8.191520442889917e-1+sin(q2-q3).*cos(q4).*cos(q5)-sin(q2-q3).*sin(q4).*sin(q5).*5.735764363510462e-1))+real(cos(q2-q3).*sin(q4).*(dq2-dq3)).*4.698463103929542e-1-imag(sin(q6).*(dq5.*cos(q2-q3).*cos(q5).*(-8.191520442889917e-1)+sin(q2-q3).*sin(q5).*(dq2-dq3).*8.191520442889917e-1+dq4.*sin(q2-q3).*cos(q4).*sin(q5).*5.735764363510462e-1+dq4.*sin(q2-q3).*cos(q5).*sin(q4)+dq5.*sin(q2-q3).*cos(q4).*sin(q5)+dq5.*sin(q2-q3).*cos(q5).*sin(q4).*5.735764363510462e-1-cos(q2-q3).*cos(q4).*cos(q5).*(dq2-dq3)+cos(q2-q3).*sin(q4).*sin(q5).*(dq2-dq3).*5.735764363510462e-1))+real(dq5.*sin(q5).*(cos(q2-q3).*8.191520442889917e-1-sin(q2-q3).*sin(q4).*5.735764363510462e-1)).*8.191520442889917e-1-real(sin(q2-q3).*(dq2-dq3)).*3.289899283371657e-1+imag(cos(q6).*(cos(q5).*(sin(q2-q3).*(dq2-dq3).*8.191520442889917e-1+dq4.*sin(q2-q3).*cos(q4).*5.735764363510462e-1+cos(q2-q3).*sin(q4).*(dq2-dq3).*5.735764363510462e-1).*5.735764363510462e-1+sin(q2-q3).*(dq2-dq3).*4.698463103929542e-1-dq4.*sin(q2-q3).*cos(q4).*6.710100716628342e-1-cos(q2-q3).*sin(q4).*(dq2-dq3).*6.710100716628342e-1+dq5.*sin(q5).*(cos(q2-q3).*8.191520442889917e-1-sin(q2-q3).*sin(q4).*5.735764363510462e-1).*5.735764363510462e-1+dq5.*sin(q2-q3).*cos(q4).*cos(q5).*5.735764363510462e-1-dq4.*sin(q2-q3).*sin(q4).*sin(q5).*5.735764363510462e-1+cos(q2-q3).*cos(q4).*sin(q5).*(dq2-dq3).*5.735764363510462e-1))+imag(dq6.*sin(q6).*(cos(q2-q3).*4.698463103929542e-1+sin(q2-q3).*sin(q4).*6.710100716628342e-1+cos(q5).*(cos(q2-q3).*8.191520442889917e-1-sin(q2-q3).*sin(q4).*5.735764363510462e-1).*5.735764363510462e-1-sin(q2-q3).*cos(q4).*sin(q5).*5.735764363510462e-1))+real(cos(q5).*(sin(q2-q3).*(dq2-dq3).*8.191520442889917e-1+dq4.*sin(q2-q3).*cos(q4).*5.735764363510462e-1+cos(q2-q3).*sin(q4).*(dq2-dq3).*5.735764363510462e-1)).*8.191520442889917e-1+real(dq5.*sin(q2-q3).*cos(q4).*cos(q5)).*8.191520442889917e-1-real(dq4.*sin(q2-q3).*sin(q4).*sin(q5)).*8.191520442889917e-1+real(cos(q2-q3).*cos(q4).*sin(q5).*(dq2-dq3)).*8.191520442889917e-1+real(dq4.*sin(q2-q3).*cos(q4)).*4.698463103929542e-1).*2.0).*((imag(sin(q2-q3).*cos(q4).*cos(q5)).*8.191520442889917e-1-real(cos(q6).*(sin(q5).*(cos(q2-q3).*8.191520442889917e-1-sin(q2-q3).*sin(q4).*5.735764363510462e-1).*5.735764363510462e-1+sin(q2-q3).*cos(q4).*cos(q5).*5.735764363510462e-1))+real(sin(q6).*(cos(q2-q3).*cos(q5).*(-8.191520442889917e-1)+sin(q2-q3).*cos(q4).*sin(q5)+sin(q2-q3).*cos(q5).*sin(q4).*5.735764363510462e-1))+imag(sin(q5).*(cos(q2-q3).*8.191520442889917e-1-sin(q2-q3).*sin(q4).*5.735764363510462e-1)).*8.191520442889917e-1)./(real(cos(q2-q3)).*3.289899283371657e-1+real(sin(q2-q3).*cos(q4).*sin(q5)).*8.191520442889917e-1+real(sin(q2-q3).*sin(q4)).*4.698463103929542e-1+imag(sin(q6).*(cos(q2-q3).*sin(q5).*8.191520442889917e-1+sin(q2-q3).*cos(q4).*cos(q5)-sin(q2-q3).*sin(q4).*sin(q5).*5.735764363510462e-1))-real(cos(q5).*(cos(q2-q3).*8.191520442889917e-1-sin(q2-q3).*sin(q4).*5.735764363510462e-1)).*8.191520442889917e-1-imag(cos(q6).*(cos(q2-q3).*4.698463103929542e-1+sin(q2-q3).*sin(q4).*6.710100716628342e-1+cos(q5).*(cos(q2-q3).*8.191520442889917e-1-sin(q2-q3).*sin(q4).*5.735764363510462e-1).*5.735764363510462e-1-sin(q2-q3).*cos(q4).*sin(q5).*5.735764363510462e-1)))-(imag(cos(q6).*(sin(q5).*(cos(q2-q3).*8.191520442889917e-1-sin(q2-q3).*sin(q4).*5.735764363510462e-1).*5.735764363510462e-1+sin(q2-q3).*cos(q4).*cos(q5).*5.735764363510462e-1))+real(sin(q2-q3).*cos(q4).*cos(q5)).*8.191520442889917e-1-imag(sin(q6).*(cos(q2-q3).*cos(q5).*(-8.191520442889917e-1)+sin(q2-q3).*cos(q4).*sin(q5)+sin(q2-q3).*cos(q5).*sin(q4).*5.735764363510462e-1))+real(sin(q5).*(cos(q2-q3).*8.191520442889917e-1-sin(q2-q3).*sin(q4).*5.735764363510462e-1)).*8.191520442889917e-1).*(real(cos(q6).*(cos(q2-q3).*4.698463103929542e-1+sin(q2-q3).*sin(q4).*6.710100716628342e-1+cos(q5).*(cos(q2-q3).*8.191520442889917e-1-sin(q2-q3).*sin(q4).*5.735764363510462e-1).*5.735764363510462e-1-sin(q2-q3).*cos(q4).*sin(q5).*5.735764363510462e-1))+imag(cos(q2-q3)).*3.289899283371657e-1+imag(sin(q2-q3).*cos(q4).*sin(q5)).*8.191520442889917e-1+imag(sin(q2-q3).*sin(q4)).*4.698463103929542e-1-real(sin(q6).*(cos(q2-q3).*sin(q5).*8.191520442889917e-1+sin(q2-q3).*cos(q4).*cos(q5)-sin(q2-q3).*sin(q4).*sin(q5).*5.735764363510462e-1))-imag(cos(q5).*(cos(q2-q3).*8.191520442889917e-1-sin(q2-q3).*sin(q4).*5.735764363510462e-1)).*8.191520442889917e-1).*1.0./(real(cos(q2-q3)).*3.289899283371657e-1+real(sin(q2-q3).*cos(q4).*sin(q5)).*8.191520442889917e-1+real(sin(q2-q3).*sin(q4)).*4.698463103929542e-1+imag(sin(q6).*(cos(q2-q3).*sin(q5).*8.191520442889917e-1+sin(q2-q3).*cos(q4).*cos(q5)-sin(q2-q3).*sin(q4).*sin(q5).*5.735764363510462e-1))-real(cos(q5).*(cos(q2-q3).*8.191520442889917e-1-sin(q2-q3).*sin(q4).*5.735764363510462e-1)).*8.191520442889917e-1-imag(cos(q6).*(cos(q2-q3).*4.698463103929542e-1+sin(q2-q3).*sin(q4).*6.710100716628342e-1+cos(q5).*(cos(q2-q3).*8.191520442889917e-1-sin(q2-q3).*sin(q4).*5.735764363510462e-1).*5.735764363510462e-1-sin(q2-q3).*cos(q4).*sin(q5).*5.735764363510462e-1))).^2).*(real(cos(q2-q3)).*3.289899283371657e-1+real(sin(q2-q3).*cos(q4).*sin(q5)).*8.191520442889917e-1+real(sin(q2-q3).*sin(q4)).*4.698463103929542e-1+imag(sin(q6).*(cos(q2-q3).*sin(q5).*8.191520442889917e-1+sin(q2-q3).*cos(q4).*cos(q5)-sin(q2-q3).*sin(q4).*sin(q5).*5.735764363510462e-1))-real(cos(q5).*(cos(q2-q3).*8.191520442889917e-1-sin(q2-q3).*sin(q4).*5.735764363510462e-1)).*8.191520442889917e-1-imag(cos(q6).*(cos(q2-q3).*4.698463103929542e-1+sin(q2-q3).*sin(q4).*6.710100716628342e-1+cos(q5).*(cos(q2-q3).*8.191520442889917e-1-sin(q2-q3).*sin(q4).*5.735764363510462e-1).*5.735764363510462e-1-sin(q2-q3).*cos(q4).*sin(q5).*5.735764363510462e-1))).^2,0.0,0.0,0.0,